simulink library "GTPR_Library"  (R2021a)
(part 7 of 8)

Mddq = [ddq1.*(ILAxx.*sin(alphaAA-pi./2.0).^2+ILAyy.*cos(alphaAA-pi./2.0).^2+ILAxy.*sin(alphaAA-pi./2.0).*cos(alphaAA-pi./2.0).*2.0)+((((dx-LA.*dq1.*sin(q1).*cos(alphaAA-pi./2.0)).*(y+aA.*cos(alphaAA)-eA.*cos(alphaAA)+LA.*cos(alphaAA).*cos(q1)))./lA-((dy+LA.*dq1.*sin(alphaAA-pi./2.0).*sin(q1)).*(x+aA.*sin(alphaAA)-eA.*sin(alphaAA)+LA.*cos(q1).*sin(alphaAA)))./lA).*((IlAxz.*((LA.*cos(q1).*(dy+LA.*dq1.*sin(alphaAA-pi./2.0).*sin(q1)))./lA+(LA.*cos(alphaAA).*sin(q1).*(dz+LA.*dq1.*sin(pi./2.0).*cos(q1)))./lA+(LA.*dq1.*sin(alphaAA-pi./2.0).*cos(q1).*(z+LA.*sin(q1)))./lA+(LA.*dq1.*sin(pi./2.0).*sin(q1).*(y+aA.*cos(alphaAA)-eA.*cos(alphaAA)+LA.*cos(alphaAA).*cos(q1)))./lA).*(-1.0./2.0))./lA+(IlAyz.*((LA.*cos(q1).*(dx-LA.*dq1.*sin(q1).*cos(alphaAA-pi./2.0)))./lA+(LA.*sin(alphaAA).*sin(q1).*(dz+LA.*dq1.*sin(pi./2.0).*cos(q1)))./lA-(LA.*dq1.*cos(q1).*cos(alphaAA-pi./2.0).*(z+LA.*sin(q1)))./lA+(LA.*dq1.*sin(pi./2.0).*sin(q1).*(x+aA.*sin(alphaAA)-eA.*sin(alphaAA)+LA.*cos(q1).*sin(alphaAA)))./lA))./(lA.*2.0)+(IlAzz.*((LA.*cos(alphaAA).*sin(q1).*(dx-LA.*dq1.*sin(q1).*cos(alphaAA-pi./2.0)))./lA-(LA.*sin(alphaAA).*sin(q1).*(dy+LA.*dq1.*sin(alphaAA-pi./2.0).*sin(q1)))./lA+(LA.*dq1.*sin(alphaAA-pi./2.0).*cos(q1).*(x+aA.*sin(alphaAA)-eA.*sin(alphaAA)+LA.*cos(q1).*sin(alphaAA)))./lA+(LA.*dq1.*cos(q1).*cos(alphaAA-pi./2.0).*(y+aA.*cos(alphaAA)-eA.*cos(alphaAA)+LA.*cos(alphaAA).*cos(q1)))./lA))./(lA.*2.0)).*2.0)./lA+((((dx-LA.*dq1.*sin(q1).*cos(alphaAA-pi./2.0)).*(y+aA.*cos(alphaAA)-eA.*cos(alphaAA)+LA.*cos(alphaAA).*cos(q1)))./lA-((dy+LA.*dq1.*sin(alphaAA-pi./2.0).*sin(q1)).*(x+aA.*sin(alphaAA)-eA.*sin(alphaAA)+LA.*cos(q1).*sin(alphaAA)))./lA).*((IlAxz.*((LA.*sin(alphaAA-pi./2.0).*sin(q1).*(dz+LA.*dq1.*cos(q1)))./lA-(LA.*sin(pi./2.0).*cos(q1).*(dy-LA.*dq1.*cos(alphaAA).*sin(q1)))./lA+(LA.*dq1.*sin(alphaAA-pi./2.0).*cos(q1).*(z+LA.*sin(q1)))./lA+(LA.*dq1.*sin(pi./2.0).*sin(q1).*(y+aA.*cos(alphaAA)-eA.*cos(alphaAA)+LA.*cos(alphaAA).*cos(q1)))./lA))./(lA.*2.0)+(IlAyz.*((LA.*sin(pi./2.0).*cos(q1).*(dx-LA.*dq1.*sin(alphaAA).*sin(q1)))./lA+(LA.*sin(q1).*cos(alphaAA-pi./2.0).*(dz+LA.*dq1.*cos(q1)))./lA+(LA.*dq1.*cos(q1).*cos(alphaAA-pi./2.0).*(z+LA.*sin(q1)))./lA-(LA.*dq1.*sin(pi./2.0).*sin(q1).*(x+aA.*sin(alphaAA)-eA.*sin(alphaAA)+LA.*cos(q1).*sin(alphaAA)))./lA))./(lA.*2.0)-(IlAzz.*((LA.*sin(q1).*cos(alphaAA-pi./2.0).*(dy-LA.*dq1.*cos(alphaAA).*sin(q1)))./lA+(LA.*sin(alphaAA-pi./2.0).*sin(q1).*(dx-LA.*dq1.*sin(alphaAA).*sin(q1)))./lA+(LA.*dq1.*sin(alphaAA-pi./2.0).*cos(q1).*(x+aA.*sin(alphaAA)-eA.*sin(alphaAA)+LA.*cos(q1).*sin(alphaAA)))./lA+(LA.*dq1.*cos(q1).*cos(alphaAA-pi./2.0).*(y+aA.*cos(alphaAA)-eA.*cos(alphaAA)+LA.*cos(alphaAA).*cos(q1)))./lA))./(lA.*2.0)).*2.0)./lA-(((LA.*sin(q1).*cos(alphaAA-pi./2.0).*(y+aA.*cos(alphaAA)-eA.*cos(alphaAA)+LA.*cos(alphaAA).*cos(q1)))./lA+(LA.*sin(alphaAA-pi./2.0).*sin(q1).*(x+aA.*sin(alphaAA)-eA.*sin(alphaAA)+LA.*cos(q1).*sin(alphaAA)))./lA).*((IlAxz.*(((dz+LA.*dq1.*cos(q1)).*(dy+LA.*dq1.*sin(alphaAA-pi./2.0).*sin(q1)))./lA-((dy-LA.*dq1.*cos(alphaAA).*sin(q1)).*(dz+LA.*dq1.*sin(pi./2.0).*cos(q1)))./lA+((z+LA.*sin(q1)).*(ddy+LA.*dq1.^2.*sin(alphaAA-pi./2.0).*cos(q1)+LA.*ddq1.*sin(alphaAA-pi./2.0).*sin(q1)))./lA-((ddz+LA.*ddq1.*sin(pi./2.0).*cos(q1)-LA.*dq1.^2.*sin(pi./2.0).*sin(q1)).*(y+aA.*cos(alphaAA)-eA.*cos(alphaAA)+LA.*cos(alphaAA).*cos(q1)))./lA))./(lA.*2.0)-(IlAzz.*(-((dy-LA.*dq1.*cos(alphaAA).*sin(q1)).*(dx-LA.*dq1.*sin(q1).*cos(alphaAA-pi./2.0)))./lA+((dx-LA.*dq1.*sin(alphaAA).*sin(q1)).*(dy+LA.*dq1.*sin(alphaAA-pi./2.0).*sin(q1)))./lA+((ddy+LA.*dq1.^2.*sin(alphaAA-pi./2.0).*cos(q1)+LA.*ddq1.*sin(alphaAA-pi./2.0).*sin(q1)).*(x+aA.*sin(alphaAA)-eA.*sin(alphaAA)+LA.*cos(q1).*sin(alphaAA)))./lA+((-ddx+LA.*dq1.^2.*cos(q1).*cos(alphaAA-pi./2.0)+LA.*ddq1.*sin(q1).*cos(alphaAA-pi./2.0)).*(y+aA.*cos(alphaAA)-eA.*cos(alphaAA)+LA.*cos(alphaAA).*cos(q1)))./lA))./(lA.*2.0)+(IlAyz.*(((ddz+LA.*ddq1.*sin(pi./2.0).*cos(q1)-LA.*dq1.^2.*sin(pi./2.0).*sin(q1)).*(x+aA.*sin(alphaAA)-eA.*sin(alphaAA)+LA.*cos(q1).*sin(alphaAA)))./lA-((dz+LA.*dq1.*cos(q1)).*(dx-LA.*dq1.*sin(q1).*cos(alphaAA-pi./2.0)))./lA+((dx-LA.*dq1.*sin(alphaAA).*sin(q1)).*(dz+LA.*dq1.*sin(pi./2.0).*cos(q1)))./lA+((z+LA.*sin(q1)).*(-ddx+LA.*dq1.^2.*cos(q1).*cos(alphaAA-pi./2.0)+LA.*ddq1.*sin(q1).*cos(alphaAA-pi./2.0)))./lA))./(lA.*2.0)).*2.0)./lA+(((IlAxz.*(((dx-LA.*dq1.*sin(q1).*cos(alphaAA-pi./2.0)).*(y+aA.*cos(alphaAA)-eA.*cos(alphaAA)+LA.*cos(alphaAA).*cos(q1)))./lA-((dy+LA.*dq1.*sin(alphaAA-pi./2.0).*sin(q1)).*(x+aA.*sin(alphaAA)-eA.*sin(alphaAA)+LA.*cos(q1).*sin(alphaAA)))./lA).*(-1.0./2.0))./lA+(IlAxx.*(((dz+LA.*dq1.*sin(pi./2.0).*cos(q1)).*(y+aA.*cos(alphaAA)-eA.*cos(alphaAA)+LA.*cos(alphaAA).*cos(q1)))./lA-((z+LA.*sin(q1)).*(dy+LA.*dq1.*sin(alphaAA-pi./2.0).*sin(q1)))./lA))./(lA.*2.0)+(IlAxy.*(((z+LA.*sin(q1)).*(dx-LA.*dq1.*sin(q1).*cos(alphaAA-pi./2.0)))./lA-((dz+LA.*dq1.*sin(pi./2.0).*cos(q1)).*(x+aA.*sin(alphaAA)-eA.*sin(alphaAA)+LA.*cos(q1).*sin(alphaAA)))./lA))./(lA.*2.0)).*((LA.*cos(q1).*(dy+LA.*dq1.*sin(alphaAA-pi./2.0).*sin(q1)))./lA+(LA.*cos(alphaAA).*sin(q1).*(dz+LA.*dq1.*sin(pi./2.0).*cos(q1)))./lA+(LA.*dq1.*sin(alphaAA-pi./2.0).*cos(q1).*(z+LA.*sin(q1)))./lA+(LA.*dq1.*sin(pi./2.0).*sin(q1).*(y+aA.*cos(alphaAA)-eA.*cos(alphaAA)+LA.*cos(alphaAA).*cos(q1)))./lA).*2.0)./lA-(((IlAxz.*(((dx-LA.*dq1.*sin(q1).*cos(alphaAA-pi./2.0)).*(y+aA.*cos(alphaAA)-eA.*cos(alphaAA)+LA.*cos(alphaAA).*cos(q1)))./lA-((dy+LA.*dq1.*sin(alphaAA-pi./2.0).*sin(q1)).*(x+aA.*sin(alphaAA)-eA.*sin(alphaAA)+LA.*cos(q1).*sin(alphaAA)))./lA).*(-1.0./2.0))./lA+(IlAxx.*(((dz+LA.*dq1.*sin(pi./2.0).*cos(q1)).*(y+aA.*cos(alphaAA)-eA.*cos(alphaAA)+LA.*cos(alphaAA).*cos(q1)))./lA-((z+LA.*sin(q1)).*(dy+LA.*dq1.*sin(alphaAA-pi./2.0).*sin(q1)))./lA))./(lA.*2.0)+(IlAxy.*(((z+LA.*sin(q1)).*(dx-LA.*dq1.*sin(q1).*cos(alphaAA-pi./2.0)))./lA-((dz+LA.*dq1.*sin(pi./2.0).*cos(q1)).*(x+aA.*sin(alphaAA)-eA.*sin(alphaAA)+LA.*cos(q1).*sin(alphaAA)))./lA))./(lA.*2.0)).*((LA.*sin(alphaAA-pi./2.0).*sin(q1).*(dz+LA.*dq1.*cos(q1)))./lA-(LA.*sin(pi./2.0).*cos(q1).*(dy-LA.*dq1.*cos(alphaAA).*sin(q1)))./lA+(LA.*dq1.*sin(alphaAA-pi./2.0).*cos(q1).*(z+LA.*sin(q1)))./lA+(LA.*dq1.*sin(pi./2.0).*sin(q1).*(y+aA.*cos(alphaAA)-eA.*cos(alphaAA)+LA.*cos(alphaAA).*cos(q1)))./lA).*2.0)./lA-(((IlAxz.*((LA.*sin(q1).*cos(alphaAA-pi./2.0).*(y+aA.*cos(alphaAA)-eA.*cos(alphaAA)+LA.*cos(alphaAA).*cos(q1)))./lA+(LA.*sin(alphaAA-pi./2.0).*sin(q1).*(x+aA.*sin(alphaAA)-eA.*sin(alphaAA)+LA.*cos(q1).*sin(alphaAA)))./lA))./(lA.*2.0)+(IlAxx.*((LA.*sin(pi./2.0).*cos(q1).*(y+aA.*cos(alphaAA)-eA.*cos(alphaAA)+LA.*cos(alphaAA).*cos(q1)))./lA-(LA.*sin(alphaAA-pi./2.0).*sin(q1).*(z+LA.*sin(q1)))./lA))./(lA.*2.0)-(IlAxy.*((LA.*sin(q1).*cos(alphaAA-pi./2.0).*(z+LA.*sin(q1)))./lA+(LA.*sin(pi./2.0).*cos(q1).*(x+aA.*sin(alphaAA)-eA.*sin(alphaAA)+LA.*cos(q1).*sin(alphaAA)))./lA))./(lA.*2.0)).*(((dz+LA.*dq1.*cos(q1)).*(dy+LA.*dq1.*sin(alphaAA-pi./2.0).*sin(q1)))./lA-((dy-LA.*dq1.*cos(alphaAA).*sin(q1)).*(dz+LA.*dq1.*sin(pi./2.0).*cos(q1)))./lA+((z+LA.*sin(q1)).*(ddy+LA.*dq1.^2.*sin(alphaAA-pi./2.0).*cos(q1)+LA.*ddq1.*sin(alphaAA-pi./2.0).*sin(q1)))./lA-((ddz+LA.*ddq1.*sin(pi./2.0).*cos(q1)-LA.*dq1.^2.*sin(pi./2.0).*sin(q1)).*(y+aA.*cos(alphaAA)-eA.*cos(alphaAA)+LA.*cos(alphaAA).*cos(q1)))./lA).*2.0)./lA-(((IlAyz.*(((dx-LA.*dq1.*sin(q1).*cos(alphaAA-pi./2.0)).*(y+aA.*cos(alphaAA)-eA.*cos(alphaAA)+LA.*cos(alphaAA).*cos(q1)))./lA-((dy+LA.*dq1.*sin(alphaAA-pi./2.0).*sin(q1)).*(x+aA.*sin(alphaAA)-eA.*sin(alphaAA)+LA.*cos(q1).*sin(alphaAA)))./lA).*(-1.0./2.0))./lA+(IlAxy.*(((dz+LA.*dq1.*sin(pi./2.0).*cos(q1)).*(y+aA.*cos(alphaAA)-eA.*cos(alphaAA)+LA.*cos(alphaAA).*cos(q1)))./lA-((z+LA.*sin(q1)).*(dy+LA.*dq1.*sin(alphaAA-pi./2.0).*sin(q1)))./lA))./(lA.*2.0)+(IlAyy.*(((z+LA.*sin(q1)).*(dx-LA.*dq1.*sin(q1).*cos(alphaAA-pi./2.0)))./lA-((dz+LA.*dq1.*sin(pi./2.0).*cos(q1)).*(x+aA.*sin(alphaAA)-eA.*sin(alphaAA)+LA.*cos(q1).*sin(alphaAA)))./lA))./(lA.*2.0)).*((LA.*cos(q1).*(dx-LA.*dq1.*sin(q1).*cos(alphaAA-pi./2.0)))./lA+(LA.*sin(alphaAA).*sin(q1).*(dz+LA.*dq1.*sin(pi./2.0).*cos(q1)))./lA-(LA.*dq1.*cos(q1).*cos(alphaAA-pi./2.0).*(z+LA.*sin(q1)))./lA+(LA.*dq1.*sin(pi./2.0).*sin(q1).*(x+aA.*sin(alphaAA)-eA.*sin(alphaAA)+LA.*cos(q1).*sin(alphaAA)))./lA).*2.0)./lA-(((IlAyz.*(((dx-LA.*dq1.*sin(q1).*cos(alphaAA-pi./2.0)).*(y+aA.*cos(alphaAA)-eA.*cos(alphaAA)+LA.*cos(alphaAA).*cos(q1)))./lA-((dy+LA.*dq1.*sin(alphaAA-pi./2.0).*sin(q1)).*(x+aA.*sin(alphaAA)-eA.*sin(alphaAA)+LA.*cos(q1).*sin(alphaAA)))./lA).*(-1.0./2.0))./lA+(IlAxy.*(((dz+LA.*dq1.*sin(pi./2.0).*cos(q1)).*(y+aA.*cos(alphaAA)-eA.*cos(alphaAA)+LA.*cos(alphaAA).*cos(q1)))./lA-((z+LA.*sin(q1)).*(dy+LA.*dq1.*sin(alphaAA-pi./2.0).*sin(q1)))./lA))./(lA.*2.0)+(IlAyy.*(((z+LA.*sin(q1)).*(dx-LA.*dq1.*sin(q1).*cos(alphaAA-pi./2.0)))./lA-((dz+LA.*dq1.*sin(pi./2.0).*cos(q1)).*(x+aA.*sin(alphaAA)-eA.*sin(alphaAA)+LA.*cos(q1).*sin(alphaAA)))./lA))./(lA.*2.0)).*((LA.*sin(pi./2.0).*cos(q1).*(dx-LA.*dq1.*sin(alphaAA).*sin(q1)))./lA+(LA.*sin(q1).*cos(alphaAA-pi./2.0).*(dz+LA.*dq1.*cos(q1)))./lA+(LA.*dq1.*cos(q1).*cos(alphaAA-pi./2.0).*(z+LA.*sin(q1)))./lA-(LA.*dq1.*sin(pi./2.0).*sin(q1).*(x+aA.*sin(alphaAA)-eA.*sin(alphaAA)+LA.*cos(q1).*sin(alphaAA)))./lA).*2.0)./lA-((((dz+LA.*dq1.*sin(pi./2.0).*cos(q1)).*(y+aA.*cos(alphaAA)-eA.*cos(alphaAA)+LA.*cos(alphaAA).*cos(q1)))./lA-((z+LA.*sin(q1)).*(dy+LA.*dq1.*sin(alphaAA-pi./2.0).*sin(q1)))./lA).*((IlAxx.*((LA.*cos(q1).*(dy+LA.*dq1.*sin(alphaAA-pi./2.0).*sin(q1)))./lA+(LA.*cos(alphaAA).*sin(q1).*(dz+LA.*dq1.*sin(pi./2.0).*cos(q1)))./lA+(LA.*dq1.*sin(alphaAA-pi./2.0).*cos(q1).*(z+LA.*sin(q1)))./lA+(LA.*dq1.*sin(pi./2.0).*sin(q1).*(y+aA.*cos(alphaAA)-eA.*cos(alphaAA)+LA.*cos(alphaAA).*cos(q1)))./lA).*(-1.0./2.0))./lA+(IlAxy.*((LA.*cos(q1).*(dx-LA.*dq1.*sin(q1).*cos(alphaAA-pi./2.0)))./lA+(LA.*sin(alphaAA).*sin(q1).*(dz+LA.*dq1.*sin(pi./2.0).*cos(q1)))./lA-(LA.*dq1.*cos(q1).*cos(alphaAA-pi./2.0).*(z+LA.*sin(q1)))./lA+(LA.*dq1.*sin(pi./2.0).*sin(q1).*(x+aA.*sin(alphaAA)-eA.*sin(alphaAA)+LA.*cos(q1).*sin(alphaAA)))./lA))./(lA.*2.0)+(IlAxz.*((LA.*cos(alphaAA).*sin(q1).*(dx-LA.*dq1.*sin(q1).*cos(alphaAA-pi./2.0)))./lA-(LA.*sin(alphaAA).*sin(q1).*(dy+LA.*dq1.*sin(alphaAA-pi./2.0).*sin(q1)))./lA+(LA.*dq1.*sin(alphaAA-pi./2.0).*cos(q1).*(x+aA.*sin(alphaAA)-eA.*sin(alphaAA)+LA.*cos(q1).*sin(alphaAA)))./lA+(LA.*dq1.*cos(q1).*cos(alphaAA-pi./2.0).*(y+aA.*cos(alphaAA)-eA.*cos(alphaAA)+LA.*cos(alphaAA).*cos(q1)))./lA))./(lA.*2.0)).*2.0)./lA-((((dz+LA.*dq1.*sin(pi./2.0).*cos(q1)).*(y+aA.*cos(alphaAA)-eA.*cos(alphaAA)+LA.*cos(alphaAA).*cos(q1)))./lA-((z+LA.*sin(q1)).*(dy+LA.*dq1.*sin(alphaAA-pi./2.0).*sin(q1)))./lA).*((IlAxx.*((LA.*sin(alphaAA-pi./2.0).*sin(q1).*(dz+LA.*dq1.*cos(q1)))./lA-(LA.*sin(pi./2.0).*cos(q1).*(dy-LA.*dq1.*cos(alphaAA).*sin(q1)))./lA+(LA.*dq1.*sin(alphaAA-pi./2.0).*cos(q1).*(z+LA.*sin(q1)))./lA+(LA.*dq1.*sin(pi./2.0).*sin(q1).*(y+aA.*cos(alphaAA)-eA.*cos(alphaAA)+LA.*cos(alphaAA).*cos(q1)))./lA))./(lA.*2.0)+(IlAxy.*((LA.*sin(pi./2.0).*cos(q1).*(dx-LA.*dq1.*sin(alphaAA).*sin(q1)))./lA+(LA.*sin(q1).*cos(alphaAA-pi./2.0).*(dz+LA.*dq1.*cos(q1)))./lA+(LA.*dq1.*cos(q1).*cos(alphaAA-pi./2.0).*(z+LA.*sin(q1)))./lA-(LA.*dq1.*sin(pi./2.0).*sin(q1).*(x+aA.*sin(alphaAA)-eA.*sin(alphaAA)+LA.*cos(q1).*sin(alphaAA)))./lA))./(lA.*2.0)-(IlAxz.*((LA.*sin(q1).*cos(alphaAA-pi./2.0).*(dy-LA.*dq1.*cos(alphaAA).*sin(q1)))./lA+(LA.*sin(alphaAA-pi./2.0).*sin(q1).*(dx-LA.*dq1.*sin(alphaAA).*sin(q1)))./lA+(LA.*dq1.*sin(alphaAA-pi./2.0).*cos(q1).*(x+aA.*sin(alphaAA)-eA.*sin(alphaAA)+LA.*cos(q1).*sin(alphaAA)))./lA+(LA.*dq1.*cos(q1).*cos(alphaAA-pi./2.0).*(y+aA.*cos(alphaAA)-eA.*cos(alphaAA)+LA.*cos(alphaAA).*cos(q1)))./lA))./(lA.*2.0)).*2.0)./lA-(((LA.*sin(pi./2.0).*cos(q1).*(y+aA.*cos(alphaAA)-eA.*cos(alphaAA)+LA.*cos(alphaAA).*cos(q1)))./lA-(LA.*sin(alphaAA-pi./2.0).*sin(q1).*(z+LA.*sin(q1)))./lA).*((IlAxx.*(((dz+LA.*dq1.*cos(q1)).*(dy+LA.*dq1.*sin(alphaAA-pi./2.0).*sin(q1)))./lA-((dy-LA.*dq1.*cos(alphaAA).*sin(q1)).*(dz+LA.*dq1.*sin(pi./2.0).*cos(q1)))./lA+((z+LA.*sin(q1)).*(ddy+LA.*dq1.^2.*sin(alphaAA-pi./2.0).*cos(q1)+LA.*ddq1.*sin(alphaAA-pi./2.0).*sin(q1)))./lA-((ddz+LA.*ddq1.*sin(pi./2.0).*cos(q1)-LA.*dq1.^2.*sin(pi./2.0).*sin(q1)).*(y+aA.*cos(alphaAA)-eA.*cos(alphaAA)+LA.*cos(alphaAA).*cos(q1)))./lA))./(lA.*2.0)-(IlAxz.*(-((dy-LA.*dq1.*cos(alphaAA).*sin(q1)).*(dx-LA.*dq1.*sin(q1).*cos(alphaAA-pi./2.0)))./lA+((dx-LA.*dq1.*sin(alphaAA).*sin(q1)).*(dy+LA.*dq1.*sin(alphaAA-pi./2.0).*sin(q1)))./lA+((ddy+LA.*dq1.^2.*sin(alphaAA-pi./2.0).*cos(q1)+LA.*ddq1.*sin(alphaAA-pi./2.0).*sin(q1)).*(x+aA.*sin(alphaAA)-eA.*sin(alphaAA)+LA.*cos(q1).*sin(alphaAA)))./lA+((-ddx+LA.*dq1.^2.*cos(q1).*cos(alphaAA-pi./2.0)+LA.*ddq1.*sin(q1).*cos(alphaAA-pi./2.0)).*(y+aA.*cos(alphaAA)-eA.*cos(alphaAA)+LA.*cos(alphaAA).*cos(q1)))./lA))./(lA.*2.0)+(IlAxy.*(((ddz+LA.*ddq1.*sin(pi./2.0).*cos(q1)-LA.*dq1.^2.*sin(pi./2.0).*sin(q1)).*(x+aA.*sin(alphaAA)-eA.*sin(alphaAA)+LA.*cos(q1).*sin(alphaAA)))./lA-((dz+LA.*dq1.*cos(q1)).*(dx-LA.*dq1.*sin(q1).*cos(alphaAA-pi./2.0)))./lA+((dx-LA.*dq1.*sin(alphaAA).*sin(q1)).*(dz+LA.*dq1.*sin(pi./2.0).*cos(q1)))./lA+((z+LA.*sin(q1)).*(-ddx+LA.*dq1.^2.*cos(q1).*cos(alphaAA-pi./2.0)+LA.*ddq1.*sin(q1).*cos(alphaAA-pi./2.0)))./lA))./(lA.*2.0)).*2.0)./lA-(((IlAzz.*(((dx-LA.*dq1.*sin(q1).*cos(alphaAA-pi./2.0)).*(y+aA.*cos(alphaAA)-eA.*cos(alphaAA)+LA.*cos(alphaAA).*cos(q1)))./lA-((dy+LA.*dq1.*sin(alphaAA-pi./2.0).*sin(q1)).*(x+aA.*sin(alphaAA)-eA.*sin(alphaAA)+LA.*cos(q1).*sin(alphaAA)))./lA).*(-1.0./2.0))./lA+(IlAxz.*(((dz+LA.*dq1.*sin(pi./2.0).*cos(q1)).*(y+aA.*cos(alphaAA)-eA.*cos(alphaAA)+LA.*cos(alphaAA).*cos(q1)))./lA-((z+LA.*sin(q1)).*(dy+LA.*dq1.*sin(alphaAA-pi./2.0).*sin(q1)))./lA))./(lA.*2.0)+(IlAyz.*(((z+LA.*sin(q1)).*(dx-LA.*dq1.*sin(q1).*cos(alphaAA-pi./2.0)))./lA-((dz+LA.*dq1.*sin(pi./2.0).*cos(q1)).*(x+aA.*sin(alphaAA)-eA.*sin(alphaAA)+LA.*cos(q1).*sin(alphaAA)))./lA))./(lA.*2.0)).*((LA.*cos(alphaAA).*sin(q1).*(dx-LA.*dq1.*sin(q1).*cos(alphaAA-pi./2.0)))./lA-(LA.*sin(alphaAA).*sin(q1).*(dy+LA.*dq1.*sin(alphaAA-pi./2.0).*sin(q1)))./lA+(LA.*dq1.*sin(alphaAA-pi./2.0).*cos(q1).*(x+aA.*sin(alphaAA)-eA.*sin(alphaAA)+LA.*cos(q1).*sin(alphaAA)))./lA+(LA.*dq1.*cos(q1).*cos(alphaAA-pi./2.0).*(y+aA.*cos(alphaAA)-eA.*cos(alphaAA)+LA.*cos(alphaAA).*cos(q1)))./lA).*2.0)./lA+(((IlAzz.*(((dx-LA.*dq1.*sin(q1).*cos(alphaAA-pi./2.0)).*(y+aA.*cos(alphaAA)-eA.*cos(alphaAA)+LA.*cos(alphaAA).*cos(q1)))./lA-((dy+LA.*dq1.*sin(alphaAA-pi./2.0).*sin(q1)).*(x+aA.*sin(alphaAA)-eA.*sin(alphaAA)+LA.*cos(q1).*sin(alphaAA)))./lA).*(-1.0./2.0))./lA+(IlAxz.*(((dz+LA.*dq1.*sin(pi./2.0).*cos(q1)).*(y+aA.*cos(alphaAA)-eA.*cos(alphaAA)+LA.*cos(alphaAA).*cos(q1)))./lA-((z+LA.*sin(q1)).*(dy+LA.*dq1.*sin(alphaAA-pi./2.0).*sin(q1)))./lA))./(lA.*2.0)+(IlAyz.*(((z+LA.*sin(q1)).*(dx-LA.*dq1.*sin(q1).*cos(alphaAA-pi./2.0)))./lA-((dz+LA.*dq1.*sin(pi./2.0).*cos(q1)).*(x+aA.*sin(alphaAA)-eA.*sin(alphaAA)+LA.*cos(q1).*sin(alphaAA)))./lA))./(lA.*2.0)).*((LA.*sin(q1).*cos(alphaAA-pi./2.0).*(dy-LA.*dq1.*cos(alphaAA).*sin(q1)))./lA+(LA.*sin(alphaAA-pi./2.0).*sin(q1).*(dx-LA.*dq1.*sin(alphaAA).*sin(q1)))./lA+(LA.*dq1.*sin(alphaAA-pi./2.0).*cos(q1).*(x+aA.*sin(alphaAA)-eA.*sin(alphaAA)+LA.*cos(q1).*sin(alphaAA)))./lA+(LA.*dq1.*cos(q1).*cos(alphaAA-pi./2.0).*(y+aA.*cos(alphaAA)-eA.*cos(alphaAA)+LA.*cos(alphaAA).*cos(q1)))./lA).*2.0)./lA-((((z+LA.*sin(q1)).*(dx-LA.*dq1.*sin(q1).*cos(alphaAA-pi./2.0)))./lA-((dz+LA.*dq1.*sin(pi./2.0).*cos(q1)).*(x+aA.*sin(alphaAA)-eA.*sin(alphaAA)+LA.*cos(q1).*sin(alphaAA)))./lA).*((IlAxy.*((LA.*cos(q1).*(dy+LA.*dq1.*sin(alphaAA-pi./2.0).*sin(q1)))./lA+(LA.*cos(alphaAA).*sin(q1).*(dz+LA.*dq1.*sin(pi./2.0).*cos(q1)))./lA+(LA.*dq1.*sin(alphaAA-pi./2.0).*cos(q1).*(z+LA.*sin(q1)))./lA+(LA.*dq1.*sin(pi./2.0).*sin(q1).*(y+aA.*cos(alphaAA)-eA.*cos(alphaAA)+LA.*cos(alphaAA).*cos(q1)))./lA).*(-1.0./2.0))./lA+(IlAyy.*((LA.*cos(q1).*(dx-LA.*dq1.*sin(q1).*cos(alphaAA-pi./2.0)))./lA+(LA.*sin(alphaAA).*sin(q1).*(dz+LA.*dq1.*sin(pi./2.0).*cos(q1)))./lA-(LA.*dq1.*cos(q1).*cos(alphaAA-pi./2.0).*(z+LA.*sin(q1)))./lA+(LA.*dq1.*sin(pi./2.0).*sin(q1).*(x+aA.*sin(alphaAA)-eA.*sin(alphaAA)+LA.*cos(q1).*sin(alphaAA)))./lA))./(lA.*2.0)+(IlAyz.*((LA.*cos(alphaAA).*sin(q1).*(dx-LA.*dq1.*sin(q1).*cos(alphaAA-pi./2.0)))./lA-(LA.*sin(alphaAA).*sin(q1).*(dy+LA.*dq1.*sin(alphaAA-pi./2.0).*sin(q1)))./lA+(LA.*dq1.*sin(alphaAA-pi./2.0).*cos(q1).*(x+aA.*sin(alphaAA)-eA.*sin(alphaAA)+LA.*cos(q1).*sin(alphaAA)))./lA+(LA.*dq1.*cos(q1).*cos(alphaAA-pi./2.0).*(y+aA.*cos(alphaAA)-eA.*cos(alphaAA)+LA.*cos(alphaAA).*cos(q1)))./lA))./(lA.*2.0)).*2.0)./lA-((((z+LA.*sin(q1)).*(dx-LA.*dq1.*sin(q1).*cos(alphaAA-pi./2.0)))./lA-((dz+LA.*dq1.*sin(pi./2.0).*cos(q1)).*(x+aA.*sin(alphaAA)-eA.*sin(alphaAA)+LA.*cos(q1).*sin(alphaAA)))./lA).*((IlAxy.*((LA.*sin(alphaAA-pi./2.0).*sin(q1).*(dz+LA.*dq1.*cos(q1)))./lA-(LA.*sin(pi./2.0).*cos(q1).*(dy-LA.*dq1.*cos(alphaAA).*sin(q1)))./lA+(LA.*dq1.*sin(alphaAA-pi./2.0).*cos(q1).*(z+LA.*sin(q1)))./lA+(LA.*dq1.*sin(pi./2.0).*sin(q1).*(y+aA.*cos(alphaAA)-eA.*cos(alphaAA)+LA.*cos(alphaAA).*cos(q1)))./lA))./(lA.*2.0)+(IlAyy.*((LA.*sin(pi./2.0).*cos(q1).*(dx-LA.*dq1.*sin(alphaAA).*sin(q1)))./lA+(LA.*sin(q1).*cos(alphaAA-pi./2.0).*(dz+LA.*dq1.*cos(q1)))./lA+(LA.*dq1.*cos(q1).*cos(alphaAA-pi./2.0).*(z+LA.*sin(q1)))./lA-(LA.*dq1.*sin(pi./2.0).*sin(q1).*(x+aA.*sin(alphaAA)-eA.*sin(alphaAA)+LA.*cos(q1).*sin(alphaAA)))./lA))./(lA.*2.0)-(IlAyz.*((LA.*sin(q1).*cos(alphaAA-pi./2.0).*(dy-LA.*dq1.*cos(alphaAA).*sin(q1)))./lA+(LA.*sin(alphaAA-pi./2.0).*sin(q1).*(dx-LA.*dq1.*sin(alphaAA).*sin(q1)))./lA+(LA.*dq1.*sin(alphaAA-pi./2.0).*cos(q1).*(x+aA.*sin(alphaAA)-eA.*sin(alphaAA)+LA.*cos(q1).*sin(alphaAA)))./lA+(LA.*dq1.*cos(q1).*cos(alphaAA-pi./2.0).*(y+aA.*cos(alphaAA)-eA.*cos(alphaAA)+LA.*cos(alphaAA).*cos(q1)))./lA))./(lA.*2.0)).*2.0)./lA+(((LA.*sin(q1).*cos(alphaAA-pi./2.0).*(z+LA.*sin(q1)))./lA+(LA.*sin(pi./2.0).*cos(q1).*(x+aA.*sin(alphaAA)-eA.*sin(alphaAA)+LA.*cos(q1).*sin(alphaAA)))./lA).*((IlAxy.*(((dz+LA.*dq1.*cos(q1)).*(dy+LA.*dq1.*sin(alphaAA-pi./2.0).*sin(q1)))./lA-((dy-LA.*dq1.*cos(alphaAA).*sin(q1)).*(dz+LA.*dq1.*sin(pi./2.0).*cos(q1)))./lA+((z+LA.*sin(q1)).*(ddy+LA.*dq1.^2.*sin(alphaAA-pi./2.0).*cos(q1)+LA.*ddq1.*sin(alphaAA-pi./2.0).*sin(q1)))./lA-((ddz+LA.*ddq1.*sin(pi./2.0).*cos(q1)-LA.*dq1.^2.*sin(pi./2.0).*sin(q1)).*(y+aA.*cos(alphaAA)-eA.*cos(alphaAA)+LA.*cos(alphaAA).*cos(q1)))./lA))./(lA.*2.0)-(IlAyz.*(-((dy-LA.*dq1.*cos(alphaAA).*sin(q1)).*(dx-LA.*dq1.*sin(q1).*cos(alphaAA-pi./2.0)))./lA+((dx-LA.*dq1.*sin(alphaAA).*sin(q1)).*(dy+LA.*dq1.*sin(alphaAA-pi./2.0).*sin(q1)))./lA+((ddy+LA.*dq1.^2.*sin(alphaAA-pi./2.0).*cos(q1)+LA.*ddq1.*sin(alphaAA-pi./2.0).*sin(q1)).*(x+aA.*sin(alphaAA)-eA.*sin(alphaAA)+LA.*cos(q1).*sin(alphaAA)))./lA+((-ddx+LA.*dq1.^2.*cos(q1).*cos(alphaAA-pi./2.0)+LA.*ddq1.*sin(q1).*cos(alphaAA-pi./2.0)).*(y+aA.*cos(alphaAA)-eA.*cos(alphaAA)+LA.*cos(alphaAA).*cos(q1)))./lA))./(lA.*2.0)+(IlAyy.*(((ddz+LA.*ddq1.*sin(pi./2.0).*cos(q1)-LA.*dq1.^2.*sin(pi./2.0).*sin(q1)).*(x+aA.*sin(alphaAA)-eA.*sin(alphaAA)+LA.*cos(q1).*sin(alphaAA)))./lA-((dz+LA.*dq1.*cos(q1)).*(dx-LA.*dq1.*sin(q1).*cos(alphaAA-pi./2.0)))./lA+((dx-LA.*dq1.*sin(alphaAA).*sin(q1)).*(dz+LA.*dq1.*sin(pi./2.0).*cos(q1)))./lA+((z+LA.*sin(q1)).*(-ddx+LA.*dq1.^2.*cos(q1).*cos(alphaAA-pi./2.0)+LA.*ddq1.*sin(q1).*cos(alphaAA-pi./2.0)))./lA))./(lA.*2.0)).*2.0)./lA+(((IlAzz.*((LA.*sin(q1).*cos(alphaAA-pi./2.0).*(y+aA.*cos(alphaAA)-eA.*cos(alphaAA)+LA.*cos(alphaAA).*cos(q1)))./lA+(LA.*sin(alphaAA-pi./2.0).*sin(q1).*(x+aA.*sin(alphaAA)-eA.*sin(alphaAA)+LA.*cos(q1).*sin(alphaAA)))./lA))./(lA.*2.0)+(IlAxz.*((LA.*sin(pi./2.0).*cos(q1).*(y+aA.*cos(alphaAA)-eA.*cos(alphaAA)+LA.*cos(alphaAA).*cos(q1)))./lA-(LA.*sin(alphaAA-pi./2.0).*sin(q1).*(z+LA.*sin(q1)))./lA))./(lA.*2.0)-(IlAyz.*((LA.*sin(q1).*cos(alphaAA-pi./2.0).*(z+LA.*sin(q1)))./lA+(LA.*sin(pi./2.0).*cos(q1).*(x+aA.*sin(alphaAA)-eA.*sin(alphaAA)+LA.*cos(q1).*sin(alphaAA)))./lA))./(lA.*2.0)).*(-((dy-LA.*dq1.*cos(alphaAA).*sin(q1)).*(dx-LA.*dq1.*sin(q1).*cos(alphaAA-pi./2.0)))./lA+((dx-LA.*dq1.*sin(alphaAA).*sin(q1)).*(dy+LA.*dq1.*sin(alphaAA-pi./2.0).*sin(q1)))./lA+((ddy+LA.*dq1.^2.*sin(alphaAA-pi./2.0).*cos(q1)+LA.*ddq1.*sin(alphaAA-pi./2.0).*sin(q1)).*(x+aA.*sin(alphaAA)-eA.*sin(alphaAA)+LA.*cos(q1).*sin(alphaAA)))./lA+((-ddx+LA.*dq1.^2.*cos(q1).*cos(alphaAA-pi./2.0)+LA.*ddq1.*sin(q1).*cos(alphaAA-pi./2.0)).*(y+aA.*cos(alphaAA)-eA.*cos(alphaAA)+LA.*cos(alphaAA).*cos(q1)))./lA).*2.0)./lA-(((IlAyz.*((LA.*sin(q1).*cos(alphaAA-pi./2.0).*(y+aA.*cos(alphaAA)-eA.*cos(alphaAA)+LA.*cos(alphaAA).*cos(q1)))./lA+(LA.*sin(alphaAA-pi./2.0).*sin(q1).*(x+aA.*sin(alphaAA)-eA.*sin(alphaAA)+LA.*cos(q1).*sin(alphaAA)))./lA))./(lA.*2.0)+(IlAxy.*((LA.*sin(pi./2.0).*cos(q1).*(y+aA.*cos(alphaAA)-eA.*cos(alphaAA)+LA.*cos(alphaAA).*cos(q1)))./lA-(LA.*sin(alphaAA-pi./2.0).*sin(q1).*(z+LA.*sin(q1)))./lA))./(lA.*2.0)-(IlAyy.*((LA.*sin(q1).*cos(alphaAA-pi./2.0).*(z+LA.*sin(q1)))./lA+(LA.*sin(pi./2.0).*cos(q1).*(x+aA.*sin(alphaAA)-eA.*sin(alphaAA)+LA.*cos(q1).*sin(alphaAA)))./lA))./(lA.*2.0)).*(((ddz+LA.*ddq1.*sin(pi./2.0).*cos(q1)-LA.*dq1.^2.*sin(pi./2.0).*sin(q1)).*(x+aA.*sin(alphaAA)-eA.*sin(alphaAA)+LA.*cos(q1).*sin(alphaAA)))./lA-((dz+LA.*dq1.*cos(q1)).*(dx-LA.*dq1.*sin(q1).*cos(alphaAA-pi./2.0)))./lA+((dx-LA.*dq1.*sin(alphaAA).*sin(q1)).*(dz+LA.*dq1.*sin(pi./2.0).*cos(q1)))./lA+((z+LA.*sin(q1)).*(-ddx+LA.*dq1.^2.*cos(q1).*cos(alphaAA-pi./2.0)+LA.*ddq1.*sin(q1).*cos(alphaAA-pi./2.0)))./lA).*2.0)./lA+(LA.*g.*mLA.*cos(q1))./2.0+LA.*g.*mlA.*cos(q1)-(LA.*mlA.*sin(pi./2.0).*cos(q1).*(ddz./2.0-(LA.*ddq1.*sin(pi./2.0).*cos(q1))./2.0+(LA.*dq1.^2.*sin(pi./2.0).*sin(q1))./2.0))./2.0-LA.*mlA.*sin(pi./2.0).*cos(q1).*(ddz./4.0-(LA.*ddq1.*sin(pi./2.0).*cos(q1))./4.0+(LA.*dq1.^2.*sin(pi./2.0).*sin(q1))./4.0)+(LA.*mlA.*sin(q1).*cos(alphaAA-pi./2.0).*(ddx./2.0+(LA.*dq1.^2.*cos(q1).*cos(alphaAA-pi./2.0))./2.0+(LA.*ddq1.*sin(q1).*cos(alphaAA-pi./2.0))./2.0))./2.0+LA.*mlA.*sin(q1).*cos(alphaAA-pi./2.0).*(ddx./4.0+(LA.*dq1.^2.*cos(q1).*cos(alphaAA-pi./2.0))./4.0+(LA.*ddq1.*sin(q1).*cos(alphaAA-pi./2.0))./4.0)+(LA.*mlA.*sin(alphaAA-pi./2.0).*sin(q1).*(ddy.*(-1.0./2.0)+(LA.*dq1.^2.*sin(alphaAA-pi./2.0).*cos(q1))./2.0+(LA.*ddq1.*sin(alphaAA-pi./2.0).*sin(q1))./2.0))./2.0+LA.*mlA.*sin(alphaAA-pi./2.0).*sin(q1).*(ddy.*(-1.0./4.0)+(LA.*dq1.^2.*sin(alphaAA-pi./2.0).*cos(q1))./4.0+(LA.*ddq1.*sin(alphaAA-pi./2.0).*sin(q1))./4.0);ddq2.*(ILBxx.*sin(alphaAB-pi./2.0).^2+ILByy.*cos(alphaAB-pi./2.0).^2+ILBxy.*sin(alphaAB-pi./2.0).*cos(alphaAB-pi./2.0).*2.0)+((((dx-LB.*dq2.*sin(q2).*cos(alphaAB-pi./2.0)).*(y+aB.*cos(alphaAB)-eB.*cos(alphaAB)+LB.*cos(alphaAB).*cos(q2)))./lB-((dy+LB.*dq2.*sin(alphaAB-pi./2.0).*sin(q2)).*(x+aB.*sin(alphaAB)-eB.*sin(alphaAB)+LB.*cos(q2).*sin(alphaAB)))./lB).*((IlBxz.*((LB.*cos(q2).*(dy+LB.*dq2.*sin(alphaAB-pi./2.0).*sin(q2)))./lB+(LB.*cos(alphaAB).*sin(q2).*(dz+LB.*dq2.*sin(pi./2.0).*cos(q2)))./lB+(LB.*dq2.*sin(alphaAB-pi./2.0).*cos(q2).*(z+LB.*sin(q2)))./lB+(LB.*dq2.*sin(pi./2.0).*sin(q2).*(y+aB.*cos(alphaAB)-eB.*cos(alphaAB)+LB.*cos(alphaAB).*cos(q2)))./lB).*(-1.0./2.0))./lB+(IlByz.*((LB.*cos(q2).*(dx-LB.*dq2.*sin(q2).*cos(alphaAB-pi./2.0)))./lB+(LB.*sin(alphaAB).*sin(q2).*(dz+LB.*dq2.*sin(pi./2.0).*cos(q2)))./lB-(LB.*dq2.*cos(q2).*cos(alphaAB-pi./2.0).*(z+LB.*sin(q2)))./lB+(LB.*dq2.*sin(pi./2.0).*sin(q2).*(x+aB.*sin(alphaAB)-eB.*sin(alphaAB)+LB.*cos(q2).*sin(alphaAB)))./lB))./(lB.*2.0)+(IlBzz.*((LB.*cos(alphaAB).*sin(q2).*(dx-LB.*dq2.*sin(q2).*cos(alphaAB-pi./2.0)))./lB-(LB.*sin(alphaAB).*sin(q2).*(dy+LB.*dq2.*sin(alphaAB-pi./2.0).*sin(q2)))./lB+(LB.*dq2.*sin(alphaAB-pi./2.0).*cos(q2).*(x+aB.*sin(alphaAB)-eB.*sin(alphaAB)+LB.*cos(q2).*sin(alphaAB)))./lB+(LB.*dq2.*cos(q2).*cos(alphaAB-pi./2.0).*(y+aB.*cos(alphaAB)-eB.*cos(alphaAB)+LB.*cos(alphaAB).*cos(q2)))./lB))./(lB.*2.0)).*2.0)./lB+((((dx-LB.*dq2.*sin(q2).*cos(alphaAB-pi./2.0)).*(y+aB.*cos(alphaAB)-eB.*cos(alphaAB)+LB.*cos(alphaAB).*cos(q2)))./lB-((dy+LB.*dq2.*sin(alphaAB-pi./2.0).*sin(q2)).*(x+aB.*sin(alphaAB)-eB.*sin(alphaAB)+LB.*cos(q2).*sin(alphaAB)))./lB).*((IlBxz.*((LB.*sin(alphaAB-pi./2.0).*sin(q2).*(dz+LB.*dq2.*cos(q2)))./lB-(LB.*sin(pi./2.0).*cos(q2).*(dy-LB.*dq2.*cos(alphaAB).*sin(q2)))./lB+(LB.*dq2.*sin(alphaAB-pi./2.0).*cos(q2).*(z+LB.*sin(q2)))./lB+(LB.*dq2.*sin(pi./2.0).*sin(q2).*(y+aB.*cos(alphaAB)-eB.*cos(alphaAB)+LB.*cos(alphaAB).*cos(q2)))./lB))./(lB.*2.0)+(IlByz.*((LB.*sin(pi./2.0).*cos(q2).*(dx-LB.*dq2.*sin(alphaAB).*sin(q2)))./lB+(LB.*sin(q2).*cos(alphaAB-pi./2.0).*(dz+LB.*dq2.*cos(q2)))./lB+(LB.*dq2.*cos(q2).*cos(alphaAB-pi./2.0).*(z+LB.*sin(q2)))./lB-(LB.*dq2.*sin(pi./2.0).*sin(q2).*(x+aB.*sin(alphaAB)-eB.*sin(alphaAB)+LB.*cos(q2).*sin(alphaAB)))./lB))./(lB.*2.0)-(IlBzz.*((LB.*sin(q2).*cos(alphaAB-pi./2.0).*(dy-LB.*dq2.*cos(alphaAB).*sin(q2)))./lB+(LB.*sin(alphaAB-pi./2.0).*sin(q2).*(dx-LB.*dq2.*sin(alphaAB).*sin(q2)))./lB+(LB.*dq2.*sin(alphaAB-pi./2.0).*cos(q2).*(x+aB.*sin(alphaAB)-eB.*sin(alphaAB)+LB.*cos(q2).*sin(alphaAB)))./lB+(LB.*dq2.*cos(q2).*cos(alphaAB-pi./2.0).*(y+aB.*cos(alphaAB)-eB.*cos(alphaAB)+LB.*cos(alphaAB).*cos(q2)))./lB))./(lB.*2.0)).*2.0)./lB-(((LB.*sin(q2).*cos(alphaAB-pi./2.0).*(y+aB.*cos(alphaAB)-eB.*cos(alphaAB)+LB.*cos(alphaAB).*cos(q2)))./lB+(LB.*sin(alphaAB-pi./2.0).*sin(q2).*(x+aB.*sin(alphaAB)-eB.*sin(alphaAB)+LB.*cos(q2).*sin(alphaAB)))./lB).*((IlBxz.*(((dz+LB.*dq2.*cos(q2)).*(dy+LB.*dq2.*sin(alphaAB-pi./2.0).*sin(q2)))./lB-((dy-LB.*dq2.*cos(alphaAB).*sin(q2)).*(dz+LB.*dq2.*sin(pi./2.0).*cos(q2)))./lB+((z+LB.*sin(q2)).*(ddy+LB.*dq2.^2.*sin(alphaAB-pi./2.0).*cos(q2)+LB.*ddq2.*sin(alphaAB-pi./2.0).*sin(q2)))./lB-((ddz+LB.*ddq2.*sin(pi./2.0).*cos(q2)-LB.*dq2.^2.*sin(pi./2.0).*sin(q2)).*(y+aB.*cos(alphaAB)-eB.*cos(alphaAB)+LB.*cos(alphaAB).*cos(q2)))./lB))./(lB.*2.0)-(IlBzz.*(-((dy-LB.*dq2.*cos(alphaAB).*sin(q2)).*(dx-LB.*dq2.*sin(q2).*cos(alphaAB-pi./2.0)))./lB+((dx-LB.*dq2.*sin(alphaAB).*sin(q2)).*(dy+LB.*dq2.*sin(alphaAB-pi./2.0).*sin(q2)))./lB+((ddy+LB.*dq2.^2.*sin(alphaAB-pi./2.0).*cos(q2)+LB.*ddq2.*sin(alphaAB-pi./2.0).*sin(q2)).*(x+aB.*sin(alphaAB)-eB.*sin(alphaAB)+LB.*cos(q2).*sin(alphaAB)))./lB+((-ddx+LB.*dq2.^2.*cos(q2).*cos(alphaAB-pi./2.0)+LB.*ddq2.*sin(q2).*cos(alphaAB-pi./2.0)).*(y+aB.*cos(alphaAB)-eB.*cos(alphaAB)+LB.*cos(alphaAB).*cos(q2)))./lB))./(lB.*2.0)+(IlByz.*(((ddz+LB.*ddq2.*sin(pi./2.0).*cos(q2)-LB.*dq2.^2.*sin(pi./2.0).*sin(q2)).*(x+aB.*sin(alphaAB)-eB.*sin(alphaAB)+LB.*cos(q2).*sin(alphaAB)))./lB-((dz+LB.*dq2.*cos(q2)).*(dx-LB.*dq2.*sin(q2).*cos(alphaAB-pi./2.0)))./lB+((dx-LB.*dq2.*sin(alphaAB).*sin(q2)).*(dz+LB.*dq2.*sin(pi./2.0).*cos(q2)))./lB+((z+LB.*sin(q2)).*(-ddx+LB.*dq2.^2.*cos(q2).*cos(alphaAB-pi./2.0)+LB.*ddq2.*sin(q2).*cos(alphaAB-pi./2.0)))./lB))./(lB.*2.0)).*2.0)./lB+(((IlBxz.*(((dx-LB.*dq2.*sin(q2).*cos(alphaAB-pi./2.0)).*(y+aB.*cos(alphaAB)-eB.*cos(alphaAB)+LB.*cos(alphaAB).*cos(q2)))./lB-((dy+LB.*dq2.*sin(alphaAB-pi./2.0).*sin(q2)).*(x+aB.*sin(alphaAB)-eB.*sin(alphaAB)+LB.*cos(q2).*sin(alphaAB)))./lB).*(-1.0./2.0))./lB+(IlBxx.*(((dz+LB.*dq2.*sin(pi./2.0).*cos(q2)).*(y+aB.*cos(alphaAB)-eB.*cos(alphaAB)+LB.*cos(alphaAB).*cos(q2)))./lB-((z+LB.*sin(q2)).*(dy+LB.*dq2.*sin(alphaAB-pi./2.0).*sin(q2)))./lB))./(lB.*2.0)+(IlBxy.*(((z+LB.*sin(q2)).*(dx-LB.*dq2.*sin(q2).*cos(alphaAB-pi./2.0)))./lB-((dz+LB.*dq2.*sin(pi./2.0).*cos(q2)).*(x+aB.*sin(alphaAB)-eB.*sin(alphaAB)+LB.*cos(q2).*sin(alphaAB)))./lB))./(lB.*2.0)).*((LB.*cos(q2).*(dy+LB.*dq2.*sin(alphaAB-pi./2.0).*sin(q2)))./lB+(LB.*cos(alphaAB).*sin(q2).*(dz+LB.*dq2.*sin(pi./2.0).*cos(q2)))./lB+(LB.*dq2.*sin(alphaAB-pi./2.0).*cos(q2).*(z+LB.*sin(q2)))./lB+(LB.*dq2.*sin(pi./2.0).*sin(q2).*(y+aB.*cos(alphaAB)-eB.*cos(alphaAB)+LB.*cos(alphaAB).*cos(q2)))./lB).*2.0)./lB-(((IlBxz.*(((dx-LB.*dq2.*sin(q2).*cos(alphaAB-pi./2.0)).*(y+aB.*cos(alphaAB)-eB.*cos(alphaAB)+LB.*cos(alphaAB).*cos(q2)))./lB-((dy+LB.*dq2.*sin(alphaAB-pi./2.0).*sin(q2)).*(x+aB.*sin(alphaAB)-eB.*sin(alphaAB)+LB.*cos(q2).*sin(alphaAB)))./lB).*(-1.0./2.0))./lB+(IlBxx.*(((dz+LB.*dq2.*sin(pi./2.0).*cos(q2)).*(y+aB.*cos(alphaAB)-eB.*cos(alphaAB)+LB.*cos(alphaAB).*cos(q2)))./lB-((z+LB.*sin(q2)).*(dy+LB.*dq2.*sin(alphaAB-pi./2.0).*sin(q2)))./lB))./(lB.*2.0)+(IlBxy.*(((z+LB.*sin(q2)).*(dx-LB.*dq2.*sin(q2).*cos(alphaAB-pi./2.0)))./lB-((dz+LB.*dq2.*sin(pi./2.0).*cos(q2)).*(x+aB.*sin(alphaAB)-eB.*sin(alphaAB)+LB.*cos(q2).*sin(alphaAB)))./lB))./(lB.*2.0)).*((LB.*sin(alphaAB-pi./2.0).*sin(q2).*(dz+LB.*dq2.*cos(q2)))./lB-(LB.*sin(pi./2.0).*cos(q2).*(dy-LB.*dq2.*cos(alphaAB).*sin(q2)))./lB+(LB.*dq2.*sin(alphaAB-pi./2.0).*cos(q2).*(z+LB.*sin(q2)))./lB+(LB.*dq2.*sin(pi./2.0).*sin(q2).*(y+aB.*cos(alphaAB)-eB.*cos(alphaAB)+LB.*cos(alphaAB).*cos(q2)))./lB).*2.0)./lB-(((IlBxz.*((LB.*sin(q2).*cos(alphaAB-pi./2.0).*(y+aB.*cos(alphaAB)-eB.*cos(alphaAB)+LB.*cos(alphaAB).*cos(q2)))./lB+(LB.*sin(alphaAB-pi./2.0).*sin(q2).*(x+aB.*sin(alphaAB)-eB.*sin(alphaAB)+LB.*cos(q2).*sin(alphaAB)))./lB))./(lB.*2.0)+(IlBxx.*((LB.*sin(pi./2.0).*cos(q2).*(y+aB.*cos(alphaAB)-eB.*cos(alphaAB)+LB.*cos(alphaAB).*cos(q2)))./lB-(LB.*sin(alphaAB-pi./2.0).*sin(q2).*(z+LB.*sin(q2)))./lB))./(lB.*2.0)-(IlBxy.*((LB.*sin(q2).*cos(alphaAB-pi./2.0).*(z+LB.*sin(q2)))./lB+(LB.*sin(pi./2.0).*cos(q2).*(x+aB.*sin(alphaAB)-eB.*sin(alphaAB)+LB.*cos(q2).*sin(alphaAB)))./lB))./(lB.*2.0)).*(((dz+LB.*dq2.*cos(q2)).*(dy+LB.*dq2.*sin(alphaAB-pi./2.0).*sin(q2)))./lB-((dy-LB.*dq2.*cos(alphaAB).*sin(q2)).*(dz+LB.*dq2.*sin(pi./2.0).*cos(q2)))./lB+((z+LB.*sin(q2)).*(ddy+LB.*dq2.^2.*sin(alphaAB-pi./2.0).*cos(q2)+LB.*ddq2.*sin(alphaAB-pi./2.0).*sin(q2)))./lB-((ddz+LB.*ddq2.*sin(pi./2.0).*cos(q2)-LB.*dq2.^2.*sin(pi./2.0).*sin(q2)).*(y+aB.*cos(alphaAB)-eB.*cos(alphaAB)+LB.*cos(alphaAB).*cos(q2)))./lB).*2.0)./lB-(((IlByz.*(((dx-LB.*dq2.*sin(q2).*cos(alphaAB-pi./2.0)).*(y+aB.*cos(alphaAB)-eB.*cos(alphaAB)+LB.*cos(alphaAB).*cos(q2)))./lB-((dy+LB.*dq2.*sin(alphaAB-pi./2.0).*sin(q2)).*(x+aB.*sin(alphaAB)-eB.*sin(alphaAB)+LB.*cos(q2).*sin(alphaAB)))./lB).*(-1.0./2.0))./lB+(IlBxy.*(((dz+LB.*dq2.*sin(pi./2.0).*cos(q2)).*(y+aB.*cos(alphaAB)-eB.*cos(alphaAB)+LB.*cos(alphaAB).*cos(q2)))./lB-((z+LB.*sin(q2)).*(dy+LB.*dq2.*sin(alphaAB-pi./2.0).*sin(q2)))./lB))./(lB.*2.0)+(IlByy.*(((z+LB.*sin(q2)).*(dx-LB.*dq2.*sin(q2).*cos(alphaAB-pi./2.0)))./lB-((dz+LB.*dq2.*sin(pi./2.0).*cos(q2)).*(x+aB.*sin(alphaAB)-eB.*sin(alphaAB)+LB.*cos(q2).*sin(alphaAB)))./lB))./(lB.*2.0)).*((LB.*cos(q2).*(dx-LB.*dq2.*sin(q2).*cos(alphaAB-pi./2.0)))./lB+(LB.*sin(alphaAB).*sin(q2).*(dz+LB.*dq2.*sin(pi./2.0).*cos(q2)))./lB-(LB.*dq2.*cos(q2).*cos(alphaAB-pi./2.0).*(z+LB.*sin(q2)))./lB+(LB.*dq2.*sin(pi./2.0).*sin(q2).*(x+aB.*sin(alphaAB)-eB.*sin(alphaAB)+LB.*cos(q2).*sin(alphaAB)))./lB).*2.0)./lB-(((IlByz.*(((dx-LB.*dq2.*sin(q2).*cos(alphaAB-pi./2.0)).*(y+aB.*cos(alphaAB)-eB.*cos(alphaAB)+LB.*cos(alphaAB).*cos(q2)))./lB-((dy+LB.*dq2.*sin(alphaAB-pi./2.0).*sin(q2)).*(x+aB.*sin(alphaAB)-eB.*sin(alphaAB)+LB.*cos(q2).*sin(alphaAB)))./lB).*(-1.0./2.0))./lB+(IlBxy.*(((dz+LB.*dq2.*sin(pi./2.0).*cos(q2)).*(y+aB.*cos(alphaAB)-eB.*cos(alphaAB)+LB.*cos(alphaAB).*cos(q2)))./lB-((z+LB.*sin(q2)).*(dy+LB.*dq2.*sin(alphaAB-pi./2.0).*sin(q2)))./lB))./(lB.*2.0)+(IlByy.*(((z+LB.*sin(q2)).*(dx-LB.*dq2.*sin(q2).*cos(alphaAB-pi./2.0)))./lB-((dz+LB.*dq2.*sin(pi./2.0).*cos(q2)).*(x+aB.*sin(alphaAB)-eB.*sin(alphaAB)+LB.*cos(q2).*sin(alphaAB)))./lB))./(lB.*2.0)).*((LB.*sin(pi./2.0).*cos(q2).*(dx-LB.*dq2.*sin(alphaAB).*sin(q2)))./lB+(LB.*sin(q2).*cos(alphaAB-pi./2.0).*(dz+LB.*dq2.*cos(q2)))./lB+(LB.*dq2.*cos(q2).*cos(alphaAB-pi./2.0).*(z+LB.*sin(q2)))./lB-(LB.*dq2.*sin(pi./2.0).*sin(q2).*(x+aB.*sin(alphaAB)-eB.*sin(alphaAB)+LB.*cos(q2).*sin(alphaAB)))./lB).*2.0)./lB-((((dz+LB.*dq2.*sin(pi./2.0).*cos(q2)).*(y+aB.*cos(alphaAB)-eB.*cos(alphaAB)+LB.*cos(alphaAB).*cos(q2)))./lB-((z+LB.*sin(q2)).*(dy+LB.*dq2.*sin(alphaAB-pi./2.0).*sin(q2)))./lB).*((IlBxx.*((LB.*cos(q2).*(dy+LB.*dq2.*sin(alphaAB-pi./2.0).*sin(q2)))./lB+(LB.*cos(alphaAB).*sin(q2).*(dz+LB.*dq2.*sin(pi./2.0).*cos(q2)))./lB+(LB.*dq2.*sin(alphaAB-pi./2.0).*cos(q2).*(z+LB.*sin(q2)))./lB+(LB.*dq2.*sin(pi./2.0).*sin(q2).*(y+aB.*cos(alphaAB)-eB.*cos(alphaAB)+LB.*cos(alphaAB).*cos(q2)))./lB).*(-1.0./2.0))./lB+(IlBxy.*((LB.*cos(q2).*(dx-LB.*dq2.*sin(q2).*cos(alphaAB-pi./2.0)))./lB+(LB.*sin(alphaAB).*sin(q2).*(dz+LB.*dq2.*sin(pi./2.0).*cos(q2)))./lB-(LB.*dq2.*cos(q2).*cos(alphaAB-pi./2.0).*(z+LB.*sin(q2)))./lB+(LB.*dq2.*sin(pi./2.0).*sin(q2).*(x+aB.*sin(alphaAB)-eB.*sin(alphaAB)+LB.*cos(q2).*sin(alphaAB)))./lB))./(lB.*2.0)+(IlBxz.*((LB.*cos(alphaAB).*sin(q2).*(dx-LB.*dq2.*sin(q2).*cos(alphaAB-pi./2.0)))./lB-(LB.*sin(alphaAB).*sin(q2).*(dy+LB.*dq2.*sin(alphaAB-pi./2.0).*sin(q2)))./lB+(LB.*dq2.*sin(alphaAB-pi./2.0).*cos(q2).*(x+aB.*sin(alphaAB)-eB.*sin(alphaAB)+LB.*cos(q2).*sin(alphaAB)))./lB+(LB.*dq2.*cos(q2).*cos(alphaAB-pi./2.0).*(y+aB.*cos(alphaAB)-eB.*cos(alphaAB)+LB.*cos(alphaAB).*cos(q2)))./lB))./(lB.*2.0)).*2.0)./lB-((((dz+LB.*dq2.*sin(pi./2.0).*cos(q2)).*(y+aB.*cos(alphaAB)-eB.*cos(alphaAB)+LB.*cos(alphaAB).*cos(q2)))./lB-((z+LB.*sin(q2)).*(dy+LB.*dq2.*sin(alphaAB-pi./2.0).*sin(q2)))./lB).*((IlBxx.*((LB.*sin(alphaAB-pi./2.0).*sin(q2).*(dz+LB.*dq2.*cos(q2)))./lB-(LB.*sin(pi./2.0).*cos(q2).*(dy-LB.*dq2.*cos(alphaAB).*sin(q2)))./lB+(LB.*dq2.*sin(alphaAB-pi./2.0).*cos(q2).*(z+LB.*sin(q2)))./lB+(LB.*dq2.*sin(pi./2.0).*sin(q2).*(y+aB.*cos(alphaAB)-eB.*cos(alphaAB)+LB.*cos(alphaAB).*cos(q2)))./lB))./(lB.*2.0)+(IlBxy.*((LB.*sin(pi./2.0).*cos(q2).*(dx-LB.*dq2.*sin(alphaAB).*sin(q2)))./lB+(LB.*sin(q2).*cos(alphaAB-pi./2.0).*(dz+LB.*dq2.*cos(q2)))./lB+(LB.*dq2.*cos(q2).*cos(alphaAB-pi./2.0).*(z+LB.*sin(q2)))./lB-(LB.*dq2.*sin(pi./2.0).*sin(q2).*(x+aB.*sin(alphaAB)-eB.*sin(alphaAB)+LB.*cos(q2).*sin(alphaAB)))./lB))./(lB.*2.0)-(IlBxz.*((LB.*sin(q2).*cos(alphaAB-pi./2.0).*(dy-LB.*dq2.*cos(alphaAB).*sin(q2)))./lB+(LB.*sin(alphaAB-pi./2.0).*sin(q2).*(dx-LB.*dq2.*sin(alphaAB).*sin(q2)))./lB+(LB.*dq2.*sin(alphaAB-pi./2.0).*cos(q2).*(x+aB.*sin(alphaAB)-eB.*sin(alphaAB)+LB.*cos(q2).*sin(alphaAB)))./lB+(LB.*dq2.*cos(q2).*cos(alphaAB-pi./2.0).*(y+aB.*cos(alphaAB)-eB.*cos(alphaAB)+LB.*cos(alphaAB).*cos(q2)))./lB))./(lB.*2.0)).*2.0)./lB-(((LB.*sin(pi./2.0).*cos(q2).*(y+aB.*cos(alphaAB)-eB.*cos(alphaAB)+LB.*cos(alphaAB).*cos(q2)))./lB-(LB.*sin(alphaAB-pi./2.0).*sin(q2).*(z+LB.*sin(q2)))./lB).*((IlBxx.*(((dz+LB.*dq2.*cos(q2)).*(dy+LB.*dq2.*sin(alphaAB-pi./2.0).*sin(q2)))./lB-((dy-LB.*dq2.*cos(alphaAB).*sin(q2)).*(dz+LB.*dq2.*sin(pi./2.0).*cos(q2)))./lB+((z+LB.*sin(q2)).*(ddy+LB.*dq2.^2.*sin(alphaAB-pi./2.0).*cos(q2)+LB.*ddq2.*sin(alphaAB-pi./2.0).*sin(q2)))./lB-((ddz+LB.*ddq2.*sin(pi./2.0).*cos(q2)-LB.*dq2.^2.*sin(pi./2.0).*sin(q2)).*(y+aB.*cos(alphaAB)-eB.*cos(alphaAB)+LB.*cos(alphaAB).*cos(q2)))./lB))./(lB.*2.0)-(IlBxz.*(-((dy-LB.*dq2.*cos(alphaAB).*sin(q2)).*(dx-LB.*dq2.*sin(q2).*cos(alphaAB-pi./2.0)))./lB+((dx-LB.*dq2.*sin(alphaAB).*sin(q2)).*(dy+LB.*dq2.*sin(alphaAB-pi./2.0).*sin(q2)))./lB+((ddy+LB.*dq2.^2.*sin(alphaAB-pi./2.0).*cos(q2)+LB.*ddq2.*sin(alphaAB-pi./2.0).*sin(q2)).*(x+aB.*sin(alphaAB)-eB.*sin(alphaAB)+LB.*cos(q2).*sin(alphaAB)))./lB+((-ddx+LB.*dq2.^2.*cos(q2).*cos(alphaAB-pi./2.0)+LB.*ddq2.*sin(q2).*cos(alphaAB-pi./2.0)).*(y+aB.*cos(alphaAB)-eB.*cos(alphaAB)+LB.*cos(alphaAB).*cos(q2)))./lB))./(lB.*2.0)+(IlBxy.*(((ddz+LB.*ddq2.*sin(pi./2.0).*cos(q2)-LB.*dq2.^2.*sin(pi./2.0).*sin(q2)).*(x+aB.*sin(alphaAB)-eB.*sin(alphaAB)+LB.*cos(q2).*sin(alphaAB)))./lB-((dz+LB.*dq2.*cos(q2)).*(dx-LB.*dq2.*sin(q2).*cos(alphaAB-pi./2.0)))./lB+((dx-LB.*dq2.*sin(alphaAB).*sin(q2)).*(dz+LB.*dq2.*sin(pi./2.0).*cos(q2)))./lB+((z+LB.*sin(q2)).*(-ddx+LB.*dq2.^2.*cos(q2).*cos(alphaAB-pi./2.0)+LB.*ddq2.*sin(q2).*cos(alphaAB-pi./2.0)))./lB))./(lB.*2.0)).*2.0)./lB-(((IlBzz.*(((dx-LB.*dq2.*sin(q2).*cos(alphaAB-pi./2.0)).*(y+aB.*cos(alphaAB)-eB.*cos(alphaAB)+LB.*cos(alphaAB).*cos(q2)))./lB-((dy+LB.*dq2.*sin(alphaAB-pi./2.0).*sin(q2)).*(x+aB.*sin(alphaAB)-eB.*sin(alphaAB)+LB.*cos(q2).*sin(alphaAB)))./lB).*(-1.0./2.0))./lB+(IlBxz.*(((dz+LB.*dq2.*sin(pi./2.0).*cos(q2)).*(y+aB.*cos(alphaAB)-eB.*cos(alphaAB)+LB.*cos(alphaAB).*cos(q2)))./lB-((z+LB.*sin(q2)).*(dy+LB.*dq2.*sin(alphaAB-pi./2.0).*sin(q2)))./lB))./(lB.*2.0)+(IlByz.*(((z+LB.*sin(q2)).*(dx-LB.*dq2.*sin(q2).*cos(alphaAB-pi./2.0)))./lB-((dz+LB.*dq2.*sin(pi./2.0).*cos(q2)).*(x+aB.*sin(alphaAB)-eB.*sin(alphaAB)+LB.*cos(q2).*sin(alphaAB)))./lB))./(lB.*2.0)).*((LB.*cos(alphaAB).*sin(q2).*(dx-LB.*dq2.*sin(q2).*cos(alphaAB-pi./2.0)))./lB-(LB.*sin(alphaAB).*sin(q2).*(dy+LB.*dq2.*sin(alphaAB-pi./2.0).*sin(q2)))./lB+(LB.*dq2.*sin(alphaAB-pi./2.0).*cos(q2).*(x+aB.*sin(alphaAB)-eB.*sin(alphaAB)+LB.*cos(q2).*sin(alphaAB)))./lB+(LB.*dq2.*cos(q2).*cos(alphaAB-pi./2.0).*(y+aB.*cos(alphaAB)-eB.*cos(alphaAB)+LB.*cos(alphaAB).*cos(q2)))./lB).*2.0)./lB+(((IlBzz.*(((dx-LB.*dq2.*sin(q2).*cos(alphaAB-pi./2.0)).*(y+aB.*cos(alphaAB)-eB.*cos(alphaAB)+LB.*cos(alphaAB).*cos(q2)))./lB-((dy+LB.*dq2.*sin(alphaAB-pi./2.0).*sin(q2)).*(x+aB.*sin(alphaAB)-eB.*sin(alphaAB)+LB.*cos(q2).*sin(alphaAB)))./lB).*(-1.0./2.0))./lB+(IlBxz.*(((dz+LB.*dq2.*sin(pi./2.0).*cos(q2)).*(y+aB.*cos(alphaAB)-eB.*cos(alphaAB)+LB.*cos(alphaAB).*cos(q2)))./lB-((z+LB.*sin(q2)).*(dy+LB.*dq2.*sin(alphaAB-pi./2.0).*sin(q2)))./lB))./(lB.*2.0)+(IlByz.*(((z+LB.*sin(q2)).*(dx-LB.*dq2.*sin(q2).*cos(alphaAB-pi./2.0)))./lB-((dz+LB.*dq2.*sin(pi./2.0).*cos(q2)).*(x+aB.*sin(alphaAB)-eB.*sin(alphaAB)+LB.*cos(q2).*sin(alphaAB)))./lB))./(lB.*2.0)).*((LB.*sin(q2).*cos(alphaAB-pi./2.0).*(dy-LB.*dq2.*cos(alphaAB).*sin(q2)))./lB+(LB.*sin(alphaAB-pi./2.0).*sin(q2).*(dx-LB.*dq2.*sin(alphaAB).*sin(q2)))./lB+(LB.*dq2.*sin(alphaAB-pi./2.0).*cos(q2).*(x+aB.*sin(alphaAB)-eB.*sin(alphaAB)+LB.*cos(q2).*sin(alphaAB)))./lB+(LB.*dq2.*cos(q2).*cos(alphaAB-pi./2.0).*(y+aB.*cos(alphaAB)-eB.*cos(alphaAB)+LB.*cos(alphaAB).*cos(q2)))./lB).*2.0)./lB-((((z+LB.*sin(q2)).*(dx-LB.*dq2.*sin(q2).*cos(alphaAB-pi./2.0)))./lB-((dz+LB.*dq2.*sin(pi./2.0).*cos(q2)).*(x+aB.*sin(alphaAB)-eB.*sin(alphaAB)+LB.*cos(q2).*sin(alphaAB)))./lB).*((IlBxy.*((LB.*cos(q2).*(dy+LB.*dq2.*sin(alphaAB-pi./2.0).*sin(q2)))./lB+(LB.*cos(alphaAB).*sin(q2).*(dz+LB.*dq2.*sin(pi./2.0).*cos(q2)))./lB+(LB.*dq2.*sin(alphaAB-pi./2.0).*cos(q2).*(z+LB.*sin(q2)))./lB+(LB.*dq2.*sin(pi./2.0).*sin(q2).*(y+aB.*cos(alphaAB)-eB.*cos(alphaAB)+LB.*cos(alphaAB).*cos(q2)))./lB).*(-1.0./2.0))./lB+(IlByy.*((LB.*cos(q2).*(dx-LB.*dq2.*sin(q2).*cos(alphaAB-pi./2.0)))./lB+(LB.*sin(alphaAB).*sin(q2).*(dz+LB.*dq2.*sin(pi./2.0).*cos(q2)))./lB-(LB.*dq2.*cos(q2).*cos(alphaAB-pi./2.0).*(z+LB.*sin(q2)))./lB+(LB.*dq2.*sin(pi./2.0).*sin(q2).*(x+aB.*sin(alphaAB)-eB.*sin(alphaAB)+LB.*cos(q2).*sin(alphaAB)))./lB))./(lB.*2.0)+(IlByz.*((LB.*cos(alphaAB).*sin(q2).*(dx-LB.*dq2.*sin(q2).*cos(alphaAB-pi./2.0)))./lB-(LB.*sin(alphaAB).*sin(q2).*(dy+LB.*dq2.*sin(alphaAB-pi./2.0).*sin(q2)))./lB+(LB.*dq2.*sin(alphaAB-pi./2.0).*cos(q2).*(x+aB.*sin(alphaAB)-eB.*sin(alphaAB)+LB.*cos(q2).*sin(alphaAB)))./lB+(LB.*dq2.*cos(q2).*cos(alphaAB-pi./2.0).*(y+aB.*cos(alphaAB)-eB.*cos(alphaAB)+LB.*cos(alphaAB).*cos(q2)))./lB))./(lB.*2.0)).*2.0)./lB-((((z+LB.*sin(q2)).*(dx-LB.*dq2.*sin(q2).*cos(alphaAB-pi./2.0)))./lB-((dz+LB.*dq2.*sin(pi./2.0).*cos(q2)).*(x+aB.*sin(alphaAB)-eB.*sin(alphaAB)+LB.*cos(q2).*sin(alphaAB)))./lB).*((IlBxy.*((LB.*sin(alphaAB-pi./2.0).*sin(q2).*(dz+LB.*dq2.*cos(q2)))./lB-(LB.*sin(pi./2.0).*cos(q2).*(dy-LB.*dq2.*cos(alphaAB).*sin(q2)))./lB+(LB.*dq2.*sin(alphaAB-pi./2.0).*cos(q2).*(z+LB.*sin(q2)))./lB+(LB.*dq2.*sin(pi./2.0).*sin(q2).*(y+aB.*cos(alphaAB)-eB.*cos(alphaAB)+LB.*cos(alphaAB).*cos(q2)))./lB))./(lB.*2.0)+(IlByy.*((LB.*sin(pi./2.0).*cos(q2).*(dx-LB.*dq2.*sin(alphaAB).*sin(q2)))./lB+(LB.*sin(q2).*cos(alphaAB-pi./2.0).*(dz+LB.*dq2.*cos(q2)))./lB+(LB.*dq2.*cos(q2).*cos(alphaAB-pi./2.0).*(z+LB.*sin(q2)))./lB-(LB.*dq2.*sin(pi./2.0).*sin(q2).*(x+aB.*sin(alphaAB)-eB.*sin(alphaAB)+LB.*cos(q2).*sin(alphaAB)))./lB))./(lB.*2.0)-(IlByz.*((LB.*sin(q2).*cos(alphaAB-pi./2.0).*(dy-LB.*dq2.*cos(alphaAB).*sin(q2)))./lB+(LB.*sin(alphaAB-pi./2.0).*sin(q2).*(dx-LB.*dq2.*sin(alphaAB).*sin(q2)))./lB+(LB.*dq2.*sin(alphaAB-pi./2.0).*cos(q2).*(x+aB.*sin(alphaAB)-eB.*sin(alphaAB)+LB.*cos(q2).*sin(alphaAB)))./lB+(LB.*dq2.*cos(q2).*cos(alphaAB-pi./2.0).*(y+aB.*cos(alphaAB)-eB.*cos(alphaAB)+LB.*cos(alphaAB).*cos(q2)))./lB))./(lB.*2.0)).*2.0)./lB+(((LB.*sin(q2).*cos(alphaAB-pi./2.0).*(z+LB.*sin(q2)))./lB+(LB.*sin(pi./2.0).*cos(q2).*(x+aB.*sin(alphaAB)-eB.*sin(alphaAB)+LB.*cos(q2).*sin(alphaAB)))./lB).*((IlBxy.*(((dz+LB.*dq2.*cos(q2)).*(dy+LB.*dq2.*sin(alphaAB-pi./2.0).*sin(q2)))./lB-((dy-LB.*dq2.*cos(alphaAB).*sin(q2)).*(dz+LB.*dq2.*sin(pi./2.0).*cos(q2)))./lB+((z+LB.*sin(q2)).*(ddy+LB.*dq2.^2.*sin(alphaAB-pi./2.0).*cos(q2)+LB.*ddq2.*sin(alphaAB-pi./2.0).*sin(q2)))./lB-((ddz+LB.*ddq2.*sin(pi./2.0).*cos(q2)-LB.*dq2.^2.*sin(pi./2.0).*sin(q2)).*(y+aB.*cos(alphaAB)-eB.*cos(alphaAB)+LB.*cos(alphaAB).*cos(q2)))./lB))./(lB.*2.0)-(IlByz.*(-((dy-LB.*dq2.*cos(alphaAB).*sin(q2)).*(dx-LB.*dq2.*sin(q2).*cos(alphaAB-pi./2.0)))./lB+((dx-LB.*dq2.*sin(alphaAB).*sin(q2)).*(dy+LB.*dq2.*sin(alphaAB-pi./2.0).*sin(q2)))./lB+((ddy+LB.*dq2.^2.*sin(alphaAB-pi./2.0).*cos(q2)+LB.*ddq2.*sin(alphaAB-pi./2.0).*sin(q2)).*(x+aB.*sin(alphaAB)-eB.*sin(alphaAB)+LB.*cos(q2).*sin(alphaAB)))./lB+((-ddx+LB.*dq2.^2.*cos(q2).*cos(alphaAB-pi./2.0)+LB.*ddq2.*sin(q2).*cos(alphaAB-pi./2.0)).*(y+aB.*cos(alphaAB)-eB.*cos(alphaAB)+LB.*cos(alphaAB).*cos(q2)))./lB))./(lB.*2.0)+(IlByy.*(((ddz+LB.*ddq2.*sin(pi./2.0).*cos(q2)-LB.*dq2.^2.*sin(pi./2.0).*sin(q2)).*(x+aB.*sin(alphaAB)-eB.*sin(alphaAB)+LB.*cos(q2).*sin(alphaAB)))./lB-((dz+LB.*dq2.*cos(q2)).*(dx-LB.*dq2.*sin(q2).*cos(alphaAB-pi./2.0)))./lB+((dx-LB.*dq2.*sin(alphaAB).*sin(q2)).*(dz+LB.*dq2.*sin(pi./2.0).*cos(q2)))./lB+((z+LB.*sin(q2)).*(-ddx+LB.*dq2.^2.*cos(q2).*cos(alphaAB-pi./2.0)+LB.*ddq2.*sin(q2).*cos(alphaAB-pi./2.0)))./lB))./(lB.*2.0)).*2.0)./lB+(((IlBzz.*((LB.*sin(q2).*cos(alphaAB-pi./2.0).*(y+aB.*cos(alphaAB)-eB.*cos(alphaAB)+LB.*cos(alphaAB).*cos(q2)))./lB+(LB.*sin(alphaAB-pi./2.0).*sin(q2).*(x+aB.*sin(alphaAB)-eB.*sin(alphaAB)+LB.*cos(q2).*sin(alphaAB)))./lB))./(lB.*2.0)+(IlBxz.*((LB.*sin(pi./2.0).*cos(q2).*(y+aB.*cos(alphaAB)-eB.*cos(alphaAB)+LB.*cos(alphaAB).*cos(q2)))./lB-(LB.*sin(alphaAB-pi./2.0).*sin(q2).*(z+LB.*sin(q2)))./lB))./(lB.*2.0)-(IlByz.*((LB.*sin(q2).*cos(alphaAB-pi./2.0).*(z+LB.*sin(q2)))./lB+(LB.*sin(pi./2.0).*cos(q2).*(x+aB.*sin(alphaAB)-eB.*sin(alphaAB)+LB.*cos(q2).*sin(alphaAB)))./lB))./(lB.*2.0)).*(-((dy-LB.*dq2.*cos(alphaAB).*sin(q2)).*(dx-LB.*dq2.*sin(q2).*cos(alphaAB-pi./2.0)))./lB+((dx-LB.*dq2.*sin(alphaAB).*sin(q2)).*(dy+LB.*dq2.*sin(alphaAB-pi./2.0).*sin(q2)))./lB+((ddy+LB.*dq2.^2.*sin(alphaAB-pi./2.0).*cos(q2)+LB.*ddq2.*sin(alphaAB-pi./2.0).*sin(q2)).*(x+aB.*sin(alphaAB)-eB.*sin(alphaAB)+LB.*cos(q2).*sin(alphaAB)))./lB+((-ddx+LB.*dq2.^2.*cos(q2).*cos(alphaAB-pi./2.0)+LB.*ddq2.*sin(q2).*cos(alphaAB-pi./2.0)).*(y+aB.*cos(alphaAB)-eB.*cos(alphaAB)+LB.*cos(alphaAB).*cos(q2)))./lB).*2.0)./lB-(((IlByz.*((LB.*sin(q2).*cos(alphaAB-pi./2.0).*(y+aB.*cos(alphaAB)-eB.*cos(alphaAB)+LB.*cos(alphaAB).*cos(q2)))./lB+(LB.*sin(alphaAB-pi./2.0).*sin(q2).*(x+aB.*sin(alphaAB)-eB.*sin(alphaAB)+LB.*cos(q2).*sin(alphaAB)))./lB))./(lB.*2.0)+(IlBxy.*((LB.*sin(pi./2.0).*cos(q2).*(y+aB.*cos(alphaAB)-eB.*cos(alphaAB)+LB.*cos(alphaAB).*cos(q2)))./lB-(LB.*sin(alphaAB-pi./2.0).*sin(q2).*(z+LB.*sin(q2)))./lB))./(lB.*2.0)-(IlByy.*((LB.*sin(q2).*cos(alphaAB-pi./2.0).*(z+LB.*sin(q2)))./lB+(LB.*sin(pi./2.0).*cos(q2).*(x+aB.*sin(alphaAB)-eB.*sin(alphaAB)+LB.*cos(q2).*sin(alphaAB)))./lB))./(lB.*2.0)).*(((ddz+LB.*ddq2.*sin(pi./2.0).*cos(q2)-LB.*dq2.^2.*sin(pi./2.0).*sin(q2)).*(x+aB.*sin(alphaAB)-eB.*sin(alphaAB)+LB.*cos(q2).*sin(alphaAB)))./lB-((dz+LB.*dq2.*cos(q2)).*(dx-LB.*dq2.*sin(q2).*cos(alphaAB-pi./2.0)))./lB+((dx-LB.*dq2.*sin(alphaAB).*sin(q2)).*(dz+LB.*dq2.*sin(pi./2.0).*cos(q2)))./lB+((z+LB.*sin(q2)).*(-ddx+LB.*dq2.^2.*cos(q2).*cos(alphaAB-pi./2.0)+LB.*ddq2.*sin(q2).*cos(alphaAB-pi./2.0)))./lB).*2.0)./lB+(LB.*g.*mLB.*cos(q2))./2.0+LB.*g.*mlB.*cos(q2)-(LB.*mlB.*sin(pi./2.0).*cos(q2).*(ddz./2.0-(LB.*ddq2.*sin(pi./2.0).*cos(q2))./2.0+(LB.*dq2.^2.*sin(pi./2.0).*sin(q2))./2.0))./2.0-LB.*mlB.*sin(pi./2.0).*cos(q2).*(ddz./4.0-(LB.*ddq2.*sin(pi./2.0).*cos(q2))./4.0+(LB.*dq2.^2.*sin(pi./2.0).*sin(q2))./4.0)+(LB.*mlB.*sin(q2).*cos(alphaAB-pi./2.0).*(ddx./2.0+(LB.*dq2.^2.*cos(q2).*cos(alphaAB-pi./2.0))./2.0+(LB.*ddq2.*sin(q2).*cos(alphaAB-pi./2.0))./2.0))./2.0+LB.*mlB.*sin(q2).*cos(alphaAB-pi./2.0).*(ddx./4.0+(LB.*dq2.^2.*cos(q2).*cos(alphaAB-pi./2.0))./4.0+(LB.*ddq2.*sin(q2).*cos(alphaAB-pi./2.0))./4.0)+(LB.*mlB.*sin(alphaAB-pi./2.0).*sin(q2).*(ddy.*(-1.0./2.0)+(LB.*dq2.^2.*sin(alphaAB-pi./2.0).*cos(q2))./2.0+(LB.*ddq2.*sin(alphaAB-pi./2.0).*sin(q2))./2.0))./2.0+LB.*mlB.*sin(alphaAB-pi./2.0).*sin(q2).*(ddy.*(-1.0./4.0)+(LB.*dq2.^2.*sin(alphaAB-pi./2.0).*cos(q2))./4.0+(LB.*ddq2.*sin(alphaAB-pi./2.0).*sin(q2))./4.0);ddq3.*(ILCxx.*sin(alphaAC-pi./2.0).^2+ILCyy.*cos(alphaAC-pi./2.0).^2+ILCxy.*sin(alphaAC-pi./2.0).*cos(alphaAC-pi./2.0).*2.0)+((((dx-LC.*dq3.*sin(q3).*cos(alphaAC-pi./2.0)).*(y+aC.*cos(alphaAC)-eC.*cos(alphaAC)+LC.*cos(alphaAC).*cos(q3)))./lC-((dy+LC.*dq3.*sin(alphaAC-pi./2.0).*sin(q3)).*(x+aC.*sin(alphaAC)-eC.*sin(alphaAC)+LC.*cos(q3).*sin(alphaAC)))./lC).*((IlCxz.*((LC.*cos(q3).*(dy+LC.*dq3.*sin(alphaAC-pi./2.0).*sin(q3)))./lC+(LC.*cos(alphaAC).*sin(q3).*(dz+LC.*dq3.*sin(pi./2.0).*cos(q3)))./lC+(LC.*dq3.*sin(alphaAC-pi./2.0).*cos(q3).*(z+LC.*sin(q3)))./lC+(LC.*dq3.*sin(pi./2.0).*sin(q3).*(y+aC.*cos(alphaAC)-eC.*cos(alphaAC)+LC.*cos(alphaAC).*cos(q3)))./lC).*(-1.0./2.0))./lC+(IlCyz.*((LC.*cos(q3).*(dx-LC.*dq3.*sin(q3).*cos(alphaAC-pi./2.0)))./lC+(LC.*sin(alphaAC).*sin(q3).*(dz+LC.*dq3.*sin(pi./2.0).*cos(q3)))./lC-(LC.*dq3.*cos(q3).*cos(alphaAC-pi./2.0).*(z+LC.*sin(q3)))./lC+(LC.*dq3.*sin(pi./2.0).*sin(q3).*(x+aC.*sin(alphaAC)-eC.*sin(alphaAC)+LC.*cos(q3).*sin(alphaAC)))./lC))./(lC.*2.0)+(IlCzz.*((LC.*cos(alphaAC).*sin(q3).*(dx-LC.*dq3.*sin(q3).*cos(alphaAC-pi./2.0)))./lC-(LC.*sin(alphaAC).*sin(q3).*(dy+LC.*dq3.*sin(alphaAC-pi./2.0).*sin(q3)))./lC+(LC.*dq3.*sin(alphaAC-pi./2.0).*cos(q3).*(x+aC.*sin(alphaAC)-eC.*sin(alphaAC)+LC.*cos(q3).*sin(alphaAC)))./lC+(LC.*dq3.*cos(q3).*cos(alphaAC-pi./2.0).*(y+aC.*cos(alphaAC)-eC.*cos(alphaAC)+LC.*cos(alphaAC).*cos(q3)))./lC))./(lC.*2.0)).*2.0)./lC+((((dx-LC.*dq3.*sin(q3).*cos(alphaAC-pi./2.0)).*(y+aC.*cos(alphaAC)-eC.*cos(alphaAC)+LC.*cos(alphaAC).*cos(q3)))./lC-((dy+LC.*dq3.*sin(alphaAC-pi./2.0).*sin(q3)).*(x+aC.*sin(alphaAC)-eC.*sin(alphaAC)+LC.*cos(q3).*sin(alphaAC)))./lC).*((IlCxz.*((LC.*sin(alphaAC-pi./2.0).*sin(q3).*(dz+LC.*dq3.*cos(q3)))./lC-(LC.*sin(pi./2.0).*cos(q3).*(dy-LC.*dq3.*cos(alphaAC).*sin(q3)))./lC+(LC.*dq3.*sin(alphaAC-pi./2.0).*cos(q3).*(z+LC.*sin(q3)))./lC+(LC.*dq3.*sin(pi./2.0).*sin(q3).*(y+aC.*cos(alphaAC)-eC.*cos(alphaAC)+LC.*cos(alphaAC).*cos(q3)))./lC))./(lC.*2.0)+(IlCyz.*((LC.*sin(pi./2.0).*cos(q3).*(dx-LC.*dq3.*sin(alphaAC).*sin(q3)))./lC+(LC.*sin(q3).*cos(alphaAC-pi./2.0).*(dz+LC.*dq3.*cos(q3)))./lC+(LC.*dq3.*cos(q3).*cos(alphaAC-pi./2.0).*(z+LC.*sin(q3)))./lC-(LC.*dq3.*sin(pi./2.0).*sin(q3).*(x+aC.*sin(alphaAC)-eC.*sin(alphaAC)+LC.*cos(q3).*sin(alphaAC)))./lC))./(lC.*2.0)-(IlCzz.*((LC.*sin(q3).*cos(alphaAC-pi./2.0).*(dy-LC.*dq3.*cos(alphaAC).*sin(q3)))./lC+(LC.*sin(alphaAC-pi./2.0).*sin(q3).*(dx-LC.*dq3.*sin(alphaAC).*sin(q3)))./lC+(LC.*dq3.*sin(alphaAC-pi./2.0).*cos(q3).*(x+aC.*sin(alphaAC)-eC.*sin(alphaAC)+LC.*cos(q3).*sin(alphaAC)))./lC+(LC.*dq3.*cos(q3).*cos(alphaAC-pi./2.0).*(y+aC.*cos(alphaAC)-eC.*cos(alphaAC)+LC.*cos(alphaAC).*cos(q3)))./lC))./(lC.*2.0)).*2.0)./lC-(((LC.*sin(q3).*cos(alphaAC-pi./2.0).*(y+aC.*cos(alphaAC)-eC.*cos(alphaAC)+LC.*cos(alphaAC).*cos(q3)))./lC+(LC.*sin(alphaAC-pi./2.0).*sin(q3).*(x+aC.*sin(alphaAC)-eC.*sin(alphaAC)+LC.*cos(q3).*sin(alphaAC)))./lC).*((IlCxz.*(((dz+LC.*dq3.*cos(q3)).*(dy+LC.*dq3.*sin(alphaAC-pi./2.0).*sin(q3)))./lC-((dy-LC.*dq3.*cos(alphaAC).*sin(q3)).*(dz+LC.*dq3.*sin(pi./2.0).*cos(q3)))./lC+((z+LC.*sin(q3)).*(ddy+LC.*dq3.^2.*sin(alphaAC-pi./2.0).*cos(q3)+LC.*ddq3.*sin(alphaAC-pi./2.0).*sin(q3)))./lC-((ddz+LC.*ddq3.*sin(pi./2.0).*cos(q3)-LC.*dq3.^2.*sin(pi./2.0).*sin(q3)).*(y+aC.*cos(alphaAC)-eC.*cos(alphaAC)+LC.*cos(alphaAC).*cos(q3)))./lC))./(lC.*2.0)-(IlCzz.*(-((dy-LC.*dq3.*cos(alphaAC).*sin(q3)).*(dx-LC.*dq3.*sin(q3).*cos(alphaAC-pi./2.0)))./lC+((dx-LC.*dq3.*sin(alphaAC).*sin(q3)).*(dy+LC.*dq3.*sin(alphaAC-pi./2.0).*sin(q3)))./lC+((ddy+LC.*dq3.^2.*sin(alphaAC-pi./2.0).*cos(q3)+LC.*ddq3.*sin(alphaAC-pi./2.0).*sin(q3)).*(x+aC.*sin(alphaAC)-eC.*sin(alphaAC)+LC.*cos(q3).*sin(alphaAC)))./lC+((-ddx+LC.*dq3.^2.*cos(q3).*cos(alphaAC-pi./2.0)+LC.*ddq3.*sin(q3).*cos(alphaAC-pi./2.0)).*(y+aC.*cos(alphaAC)-eC.*cos(alphaAC)+LC.*cos(alphaAC).*cos(q3)))./lC))./(lC.*2.0)+(IlCyz.*(((ddz+LC.*ddq3.*sin(pi./2.0).*cos(q3)-LC.*dq3.^2.*sin(pi./2.0).*sin(q3)).*(x+aC.*sin(alphaAC)-eC.*sin(alphaAC)+LC.*cos(q3).*sin(alphaAC)))./lC-((dz+LC.*dq3.*cos(q3)).*(dx-LC.*dq3.*sin(q3).*cos(alphaAC-pi./2.0)))./lC+((dx-LC.*dq3.*sin(alphaAC).*sin(q3)).*(dz+LC.*dq3.*sin(pi./2.0).*cos(q3)))./lC+((z+LC.*sin(q3)).*(-ddx+LC.*dq3.^2.*cos(q3).*cos(alphaAC-pi./2.0)+LC.*ddq3.*sin(q3).*cos(alphaAC-pi./2.0)))./lC))./(lC.*2.0)).*2.0)./lC+(((IlCxz.*(((dx-LC.*dq3.*sin(q3).*cos(alphaAC-pi./2.0)).*(y+aC.*cos(alphaAC)-eC.*cos(alphaAC)+LC.*cos(alphaAC).*cos(q3)))./lC-((dy+LC.*dq3.*sin(alphaAC-pi./2.0).*sin(q3)).*(x+aC.*sin(alphaAC)-eC.*sin(alphaAC)+LC.*cos(q3).*sin(alphaAC)))./lC).*(-1.0./2.0))./lC+(IlCxx.*(((dz+LC.*dq3.*sin(pi./2.0).*cos(q3)).*(y+aC.*cos(alphaAC)-eC.*cos(alphaAC)+LC.*cos(alphaAC).*cos(q3)))./lC-((z+LC.*sin(q3)).*(dy+LC.*dq3.*sin(alphaAC-pi./2.0).*sin(q3)))./lC))./(lC.*2.0)+(IlCxy.*(((z+LC.*sin(q3)).*(dx-LC.*dq3.*sin(q3).*cos(alphaAC-pi./2.0)))./lC-((dz+LC.*dq3.*sin(pi./2.0).*cos(q3)).*(x+aC.*sin(alphaAC)-eC.*sin(alphaAC)+LC.*cos(q3).*sin(alphaAC)))./lC))./(lC.*2.0)).*((LC.*cos(q3).*(dy+LC.*dq3.*sin(alphaAC-pi./2.0).*sin(q3)))./lC+(LC.*cos(alphaAC).*sin(q3).*(dz+LC.*dq3.*sin(pi./2.0).*cos(q3)))./lC+(LC.*dq3.*sin(alphaAC-pi./2.0).*cos(q3).*(z+LC.*sin(q3)))./lC+(LC.*dq3.*sin(pi./2.0).*sin(q3).*(y+aC.*cos(alphaAC)-eC.*cos(alphaAC)+LC.*cos(alphaAC).*cos(q3)))./lC).*2.0)./lC-(((IlCxz.*(((dx-LC.*dq3.*sin(q3).*cos(alphaAC-pi./2.0)).*(y+aC.*cos(alphaAC)-eC.*cos(alphaAC)+LC.*cos(alphaAC).*cos(q3)))./lC-((dy+LC.*dq3.*sin(alphaAC-pi./2.0).*sin(q3)).*(x+aC.*sin(alphaAC)-eC.*sin(alphaAC)+LC.*cos(q3).*sin(alphaAC)))./lC).*(-1.0./2.0))./lC+(IlCxx.*(((dz+LC.*dq3.*sin(pi./2.0).*cos(q3)).*(y+aC.*cos(alphaAC)-eC.*cos(alphaAC)+LC.*cos(alphaAC).*cos(q3)))./lC-((z+LC.*sin(q3)).*(dy+LC.*dq3.*sin(alphaAC-pi./2.0).*sin(q3)))./lC))./(lC.*2.0)+(IlCxy.*(((z+LC.*sin(q3)).*(dx-LC.*dq3.*sin(q3).*cos(alphaAC-pi./2.0)))./lC-((dz+LC.*dq3.*sin(pi./2.0).*cos(q3)).*(x+aC.*sin(alphaAC)-eC.*sin(alphaAC)+LC.*cos(q3).*sin(alphaAC)))./lC))./(lC.*2.0)).*((LC.*sin(alphaAC-pi./2.0).*sin(q3).*(dz+LC.*dq3.*cos(q3)))./lC-(LC.*sin(pi./2.0).*cos(q3).*(dy-LC.*dq3.*cos(alphaAC).*sin(q3)))./lC+(LC.*dq3.*sin(alphaAC-pi./2.0).*cos(q3).*(z+LC.*sin(q3)))./lC+(LC.*dq3.*sin(pi./2.0).*sin(q3).*(y+aC.*cos(alphaAC)-eC.*cos(alphaAC)+LC.*cos(alphaAC).*cos(q3)))./lC).*2.0)./lC-(((IlCxz.*((LC.*sin(q3).*cos(alphaAC-pi./2.0).*(y+aC.*cos(alphaAC)-eC.*cos(alphaAC)+LC.*cos(alphaAC).*cos(q3)))./lC+(LC.*sin(alphaAC-pi./2.0).*sin(q3).*(x+aC.*sin(alphaAC)-eC.*sin(alphaAC)+LC.*cos(q3).*sin(alphaAC)))./lC))./(lC.*2.0)+(IlCxx.*((LC.*sin(pi./2.0).*cos(q3).*(y+aC.*cos(alphaAC)-eC.*cos(alphaAC)+LC.*cos(alphaAC).*cos(q3)))./lC-(LC.*sin(alphaAC-pi./2.0).*sin(q3).*(z+LC.*sin(q3)))./lC))./(lC.*2.0)-(IlCxy.*((LC.*sin(q3).*cos(alphaAC-pi./2.0).*(z+LC.*sin(q3)))./lC+(LC.*sin(pi./2.0).*cos(q3).*(x+aC.*sin(alphaAC)-eC.*sin(alphaAC)+LC.*cos(q3).*sin(alphaAC)))./lC))./(lC.*2.0)).*(((dz+LC.*dq3.*cos(q3)).*(dy+LC.*dq3.*sin(alphaAC-pi./2.0).*sin(q3)))./lC-((dy-LC.*dq3.*cos(alphaAC).*sin(q3)).*(dz+LC.*dq3.*sin(pi./2.0).*cos(q3)))./lC+((z+LC.*sin(q3)).*(ddy+LC.*dq3.^2.*sin(alphaAC-pi./2.0).*cos(q3)+LC.*ddq3.*sin(alphaAC-pi./2.0).*sin(q3)))./lC-((ddz+LC.*ddq3.*sin(pi./2.0).*cos(q3)-LC.*dq3.^2.*sin(pi./2.0).*sin(q3)).*(y+aC.*cos(alphaAC)-eC.*cos(alphaAC)+LC.*cos(alphaAC).*cos(q3)))./lC).*2.0)./lC-(((IlCyz.*(((dx-LC.*dq3.*sin(q3).*cos(alphaAC-pi./2.0)).*(y+aC.*cos(alphaAC)-eC.*cos(alphaAC)+LC.*cos(alphaAC).*cos(q3)))./lC-((dy+LC.*dq3.*sin(alphaAC-pi./2.0).*sin(q3)).*(x+aC.*sin(alphaAC)-eC.*sin(alphaAC)+LC.*cos(q3).*sin(alphaAC)))./lC).*(-1.0./2.0))./lC+(IlCxy.*(((dz+LC.*dq3.*sin(pi./2.0).*cos(q3)).*(y+aC.*cos(alphaAC)-eC.*cos(alphaAC)+LC.*cos(alphaAC).*cos(q3)))./lC-((z+LC.*sin(q3)).*(dy+LC.*dq3.*sin(alphaAC-pi./2.0).*sin(q3)))./lC))./(lC.*2.0)+(IlCyy.*(((z+LC.*sin(q3)).*(dx-LC.*dq3.*sin(q3).*cos(alphaAC-pi./2.0)))./lC-((dz+LC.*dq3.*sin(pi./2.0).*cos(q3)).*(x+aC.*sin(alphaAC)-eC.*sin(alphaAC)+LC.*cos(q3).*sin(alphaAC)))./lC))./(lC.*2.0)).*((LC.*cos(q3).*(dx-LC.*dq3.*sin(q3).*cos(alphaAC-pi./2.0)))./lC+(LC.*sin(alphaAC).*sin(q3).*(dz+LC.*dq3.*sin(pi./2.0).*cos(q3)))./lC-(LC.*dq3.*cos(q3).*cos(alphaAC-pi./2.0).*(z+LC.*sin(q3)))./lC+(LC.*dq3.*sin(pi./2.0).*sin(q3).*(x+aC.*sin(alphaAC)-eC.*sin(alphaAC)+LC.*cos(q3).*sin(alphaAC)))./lC).*2.0)./lC-(((IlCyz.*(((dx-LC.*dq3.*sin(q3).*cos(alphaAC-pi./2.0)).*(y+aC.*cos(alphaAC)-eC.*cos(alphaAC)+LC.*cos(alphaAC).*cos(q3)))./lC-((dy+LC.*dq3.*sin(alphaAC-pi./2.0).*sin(q3)).*(x+aC.*sin(alphaAC)-eC.*sin(alphaAC)+LC.*cos(q3).*sin(alphaAC)))./lC).*(-1.0./2.0))./lC+(IlCxy.*(((dz+LC.*dq3.*sin(pi./2.0).*cos(q3)).*(y+aC.*cos(alphaAC)-eC.*cos(alphaAC)+LC.*cos(alphaAC).*cos(q3)))./lC-((z+LC.*sin(q3)).*(dy+LC.*dq3.*sin(alphaAC-pi./2.0).*sin(q3)))./lC))./(lC.*2.0)+(IlCyy.*(((z+LC.*sin(q3)).*(dx-LC.*dq3.*sin(q3).*cos(alphaAC-pi./2.0)))./lC-((dz+LC.*dq3.*sin(pi./2.0).*cos(q3)).*(x+aC.*sin(alphaAC)-eC.*sin(alphaAC)+LC.*cos(q3).*sin(alphaAC)))./lC))./(lC.*2.0)).*((LC.*sin(pi./2.0).*cos(q3).*(dx-LC.*dq3.*sin(alphaAC).*sin(q3)))./lC+(LC.*sin(q3).*cos(alphaAC-pi./2.0).*(dz+LC.*dq3.*cos(q3)))./lC+(LC.*dq3.*cos(q3).*cos(alphaAC-pi./2.0).*(z+LC.*sin(q3)))./lC-(LC.*dq3.*sin(pi./2.0).*sin(q3).*(x+aC.*sin(alphaAC)-eC.*sin(alphaAC)+LC.*cos(q3).*sin(alphaAC)))./lC).*2.0)./lC-((((dz+LC.*dq3.*sin(pi./2.0).*cos(q3)).*(y+aC.*cos(alphaAC)-eC.*cos(alphaAC)+LC.*cos(alphaAC).*cos(q3)))./lC-((z+LC.*sin(q3)).*(dy+LC.*dq3.*sin(alphaAC-pi./2.0).*sin(q3)))./lC).*((IlCxx.*((LC.*cos(q3).*(dy+LC.*dq3.*sin(alphaAC-pi./2.0).*sin(q3)))./lC+(LC.*cos(alphaAC).*sin(q3).*(dz+LC.*dq3.*sin(pi./2.0).*cos(q3)))./lC+(LC.*dq3.*sin(alphaAC-pi./2.0).*cos(q3).*(z+LC.*sin(q3)))./lC+(LC.*dq3.*sin(pi./2.0).*sin(q3).*(y+aC.*cos(alphaAC)-eC.*cos(alphaAC)+LC.*cos(alphaAC).*cos(q3)))./lC).*(-1.0./2.0))./lC+(IlCxy.*((LC.*cos(q3).*(dx-LC.*dq3.*sin(q3).*cos(alphaAC-pi./2.0)))./lC+(LC.*sin(alphaAC).*sin(q3).*(dz+LC.*dq3.*sin(pi./2.0).*cos(q3)))./lC-(LC.*dq3.*cos(q3).*cos(alphaAC-pi./2.0).*(z+LC.*sin(q3)))./lC+(LC.*dq3.*sin(pi./2.0).*sin(q3).*(x+aC.*sin(alphaAC)-eC.*sin(alphaAC)+LC.*cos(q3).*sin(alphaAC)))./lC))./(lC.*2.0)+(IlCxz.*((LC.*cos(alphaAC).*sin(q3).*(dx-LC.*dq3.*sin(q3).*cos(alphaAC-pi./2.0)))./lC-(LC.*sin(alphaAC).*sin(q3).*(dy+LC.*dq3.*sin(alphaAC-pi./2.0).*sin(q3)))./lC+(LC.*dq3.*sin(alphaAC-pi./2.0).*cos(q3).*(x+aC.*sin(alphaAC)-eC.*sin(alphaAC)+LC.*cos(q3).*sin(alphaAC)))./lC+(LC.*dq3.*cos(q3).*cos(alphaAC-pi./2.0).*(y+aC.*cos(alphaAC)-eC.*cos(alphaAC)+LC.*cos(alphaAC).*cos(q3)))./lC))./(lC.*2.0)).*2.0)./lC-((((dz+LC.*dq3.*sin(pi./2.0).*cos(q3)).*(y+aC.*cos(alphaAC)-eC.*cos(alphaAC)+LC.*cos(alphaAC).*cos(q3)))./lC-((z+LC.*sin(q3)).*(dy+LC.*dq3.*sin(alphaAC-pi./2.0).*sin(q3)))./lC).*((IlCxx.*((LC.*sin(alphaAC-pi./2.0).*sin(q3).*(dz+LC.*dq3.*cos(q3)))./lC-(LC.*sin(pi./2.0).*cos(q3).*(dy-LC.*dq3.*cos(alphaAC).*sin(q3)))./lC+(LC.*dq3.*sin(alphaAC-pi./2.0).*cos(q3).*(z+LC.*sin(q3)))./lC+(LC.*dq3.*sin(pi./2.0).*sin(q3).*(y+aC.*cos(alphaAC)-eC.*cos(alphaAC)+LC.*cos(alphaAC).*cos(q3)))./lC))./(lC.*2.0)+(IlCxy.*((LC.*sin(pi./2.0).*cos(q3).*(dx-LC.*dq3.*sin(alphaAC).*sin(q3)))./lC+(LC.*sin(q3).*cos(alphaAC-pi./2.0).*(dz+LC.*dq3.*cos(q3)))./lC+(LC.*dq3.*cos(q3).*cos(alphaAC-pi./2.0).*(z+LC.*sin(q3)))./lC-(LC.*dq3.*sin(pi./2.0).*sin(q3).*(x+aC.*sin(alphaAC)-eC.*sin(alphaAC)+LC.*cos(q3).*sin(alphaAC)))./lC))./(lC.*2.0)-(IlCxz.*((LC.*sin(q3).*cos(alphaAC-pi./2.0).*(dy-LC.*dq3.*cos(alphaAC).*sin(q3)))./lC+(LC.*sin(alphaAC-pi./2.0).*sin(q3).*(dx-LC.*dq3.*sin(alphaAC).*sin(q3)))./lC+(LC.*dq3.*sin(alphaAC-pi./2.0).*cos(q3).*(x+aC.*sin(alphaAC)-eC.*sin(alphaAC)+LC.*cos(q3).*sin(alphaAC)))./lC+(LC.*dq3.*cos(q3).*cos(alphaAC-pi./2.0).*(y+aC.*cos(alphaAC)-eC.*cos(alphaAC)+LC.*cos(alphaAC).*cos(q3)))./lC))./(lC.*2.0)).*2.0)./lC-(((LC.*sin(pi./2.0).*cos(q3).*(y+aC.*cos(alphaAC)-eC.*cos(alphaAC)+LC.*cos(alphaAC).*cos(q3)))./lC-(LC.*sin(alphaAC-pi./2.0).*sin(q3).*(z+LC.*sin(q3)))./lC).*((IlCxx.*(((dz+LC.*dq3.*cos(q3)).*(dy+LC.*dq3.*sin(alphaAC-pi./2.0).*sin(q3)))./lC-((dy-LC.*dq3.*cos(alphaAC).*sin(q3)).*(dz+LC.*dq3.*sin(pi./2.0).*cos(q3)))./lC+((z+LC.*sin(q3)).*(ddy+LC.*dq3.^2.*sin(alphaAC-pi./2.0).*cos(q3)+LC.*ddq3.*sin(alphaAC-pi./2.0).*sin(q3)))./lC-((ddz+LC.*ddq3.*sin(pi./2.0).*cos(q3)-LC.*dq3.^2.*sin(pi./2.0).*sin(q3)).*(y+aC.*cos(alphaAC)-eC.*cos(alphaAC)+LC.*cos(alphaAC).*cos(q3)))./lC))./(lC.*2.0)-(IlCxz.*(-((dy-LC.*dq3.*cos(alphaAC).*sin(q3)).*(dx-LC.*dq3.*sin(q3).*cos(alphaAC-pi./2.0)))./lC+((dx-LC.*dq3.*sin(alphaAC).*sin(q3)).*(dy+LC.*dq3.*sin(alphaAC-pi./2.0).*sin(q3)))./lC+((ddy+LC.*dq3.^2.*sin(alphaAC-pi./2.0).*cos(q3)+LC.*ddq3.*sin(alphaAC-pi./2.0).*sin(q3)).*(x+aC.*sin(alphaAC)-eC.*sin(alphaAC)+LC.*cos(q3).*sin(alphaAC)))./lC+((-ddx+LC.*dq3.^2.*cos(q3).*cos(alphaAC-pi./2.0)+LC.*ddq3.*sin(q3).*cos(alphaAC-pi./2.0)).*(y+aC.*cos(alphaAC)-eC.*cos(alphaAC)+LC.*cos(alphaAC).*cos(q3)))./lC))./(lC.*2.0)+(IlCxy.*(((ddz+LC.*ddq3.*sin(pi./2.0).*cos(q3)-LC.*dq3.^2.*sin(pi./2.0).*sin(q3)).*(x+aC.*sin(alphaAC)-eC.*sin(alphaAC)+LC.*cos(q3).*sin(alphaAC)))./lC-((dz+LC.*dq3.*cos(q3)).*(dx-LC.*dq3.*sin(q3).*cos(alphaAC-pi./2.0)))./lC+((dx-LC.*dq3.*sin(alphaAC).*sin(q3)).*(dz+LC.*dq3.*sin(pi./2.0).*cos(q3)))./lC+((z+LC.*sin(q3)).*(-ddx+LC.*dq3.^2.*cos(q3).*cos(alphaAC-pi./2.0)+LC.*ddq3.*sin(q3).*cos(alphaAC-pi./2.0)))./lC))./(lC.*2.0)).*2.0)./lC-(((IlCzz.*(((dx-LC.*dq3.*sin(q3).*cos(alphaAC-pi./2.0)).*(y+aC.*cos(alphaAC)-eC.*cos(alphaAC)+LC.*cos(alphaAC).*cos(q3)))./lC-((dy+LC.*dq3.*sin(alphaAC-pi./2.0).*sin(q3)).*(x+aC.*sin(alphaAC)-eC.*sin(alphaAC)+LC.*cos(q3).*sin(alphaAC)))./lC).*(-1.0./2.0))./lC+(IlCxz.*(((dz+LC.*dq3.*sin(pi./2.0).*cos(q3)).*(y+aC.*cos(alphaAC)-eC.*cos(alphaAC)+LC.*cos(alphaAC).*cos(q3)))./lC-((z+LC.*sin(q3)).*(dy+LC.*dq3.*sin(alphaAC-pi./2.0).*sin(q3)))./lC))./(lC.*2.0)+(IlCyz.*(((z+LC.*sin(q3)).*(dx-LC.*dq3.*sin(q3).*cos(alphaAC-pi./2.0)))./lC-((dz+LC.*dq3.*sin(pi./2.0).*cos(q3)).*(x+aC.*sin(alphaAC)-eC.*sin(alphaAC)+LC.*cos(q3).*sin(alphaAC)))./lC))./(lC.*2.0)).*((LC.*cos(alphaAC).*sin(q3).*(dx-LC.*dq3.*sin(q3).*cos(alphaAC-pi./2.0)))./lC-(LC.*sin(alphaAC).*sin(q3).*(dy+LC.*dq3.*sin(alphaAC-pi./2.0).*sin(q3)))./lC+(LC.*dq3.*sin(alphaAC-pi./2.0).*cos(q3).*(x+aC.*sin(alphaAC)-eC.*sin(alphaAC)+LC.*cos(q3).*sin(alphaAC)))./lC+(LC.*dq3.*cos(q3).*cos(alphaAC-pi./2.0).*(y+aC.*cos(alphaAC)-eC.*cos(alphaAC)+LC.*cos(alphaAC).*cos(q3)))./lC).*2.0)./lC+(((IlCzz.*(((dx-LC.*dq3.*sin(q3).*cos(alphaAC-pi./2.0)).*(y+aC.*cos(alphaAC)-eC.*cos(alphaAC)+LC.*cos(alphaAC).*cos(q3)))./lC-((dy+LC.*dq3.*sin(alphaAC-pi./2.0).*sin(q3)).*(x+aC.*sin(alphaAC)-eC.*sin(alphaAC)+LC.*cos(q3).*sin(alphaAC)))./lC).*(-1.0./2.0))./lC+(IlCxz.*(((dz+LC.*dq3.*sin(pi./2.0).*cos(q3)).*(y+aC.*cos(alphaAC)-eC.*cos(alphaAC)+LC.*cos(alphaAC).*cos(q3)))./lC-((z+LC.*sin(q3)).*(dy+LC.*dq3.*sin(alphaAC-pi./2.0).*sin(q3)))./lC))./(lC.*2.0)+(IlCyz.*(((z+LC.*sin(q3)).*(dx-LC.*dq3.*sin(q3).*cos(alphaAC-pi./2.0)))./lC-((dz+LC.*dq3.*sin(pi./2.0).*cos(q3)).*(x+aC.*sin(alphaAC)-eC.*sin(alphaAC)+LC.*cos(q3).*sin(alphaAC)))./lC))./(lC.*2.0)).*((LC.*sin(q3).*cos(alphaAC-pi./2.0).*(dy-LC.*dq3.*cos(alphaAC).*sin(q3)))./lC+(LC.*sin(alphaAC-pi./2.0).*sin(q3).*(dx-LC.*dq3.*sin(alphaAC).*sin(q3)))./lC+(LC.*dq3.*sin(alphaAC-pi./2.0).*cos(q3).*(x+aC.*sin(alphaAC)-eC.*sin(alphaAC)+LC.*cos(q3).*sin(alphaAC)))./lC+(LC.*dq3.*cos(q3).*cos(alphaAC-pi./2.0).*(y+aC.*cos(alphaAC)-eC.*cos(alphaAC)+LC.*cos(alphaAC).*cos(q3)))./lC).*2.0)./lC-((((z+LC.*sin(q3)).*(dx-LC.*dq3.*sin(q3).*cos(alphaAC-pi./2.0)))./lC-((dz+LC.*dq3.*sin(pi./2.0).*cos(q3)).*(x+aC.*sin(alphaAC)-eC.*sin(alphaAC)+LC.*cos(q3).*sin(alphaAC)))./lC).*((IlCxy.*((LC.*cos(q3).*(dy+LC.*dq3.*sin(alphaAC-pi./2.0).*sin(q3)))./lC+(LC.*cos(alphaAC).*sin(q3).*(dz+LC.*dq3.*sin(pi./2.0).*cos(q3)))./lC+(LC.*dq3.*sin(alphaAC-pi./2.0).*cos(q3).*(z+LC.*sin(q3)))./lC+(LC.*dq3.*sin(pi./2.0).*sin(q3).*(y+aC.*cos(alphaAC)-eC.*cos(alphaAC)+LC.*cos(alphaAC).*cos(q3)))./lC).*(-1.0./2.0))./lC+(IlCyy.*((LC.*cos(q3).*(dx-LC.*dq3.*sin(q3).*cos(alphaAC-pi./2.0)))./lC+(LC.*sin(alphaAC).*sin(q3).*(dz+LC.*dq3.*sin(pi./2.0).*cos(q3)))./lC-(LC.*dq3.*cos(q3).*cos(alphaAC-pi./2.0).*(z+LC.*sin(q3)))./lC+(LC.*dq3.*sin(pi./2.0).*sin(q3).*(x+aC.*sin(alphaAC)-eC.*sin(alphaAC)+LC.*cos(q3).*sin(alphaAC)))./lC))./(lC.*2.0)+(IlCyz.*((LC.*cos(alphaAC).*sin(q3).*(dx-LC.*dq3.*sin(q3).*cos(alphaAC-pi./2.0)))./lC-(LC.*sin(alphaAC).*sin(q3).*(dy+LC.*dq3.*sin(alphaAC-pi./2.0).*sin(q3)))./lC+(LC.*dq3.*sin(alphaAC-pi./2.0).*cos(q3).*(x+aC.*sin(alphaAC)-eC.*sin(alphaAC)+LC.*cos(q3).*sin(alphaAC)))./lC+(LC.*dq3.*cos(q3).*cos(alphaAC-pi./2.0).*(y+aC.*cos(alphaAC)-eC.*cos(alphaAC)+LC.*cos(alphaAC).*cos(q3)))./lC))./(lC.*2.0)).*2.0)./lC-((((z+LC.*sin(q3)).*(dx-LC.*dq3.*sin(q3).*cos(alphaAC-pi./2.0)))./lC-((dz+LC.*dq3.*sin(pi./2.0).*cos(q3)).*(x+aC.*sin(alphaAC)-eC.*sin(alphaAC)+LC.*cos(q3).*sin(alphaAC)))./lC).*((IlCxy.*((LC.*sin(alphaAC-pi./2.0).*sin(q3).*(dz+LC.*dq3.*cos(q3)))./lC-(LC.*sin(pi./2.0).*cos(q3).*(dy-LC.*dq3.*cos(alphaAC).*sin(q3)))./lC+(LC.*dq3.*sin(alphaAC-pi./2.0).*cos(q3).*(z+LC.*sin(q3)))./lC+(LC.*dq3.*sin(pi./2.0).*sin(q3).*(y+aC.*cos(alphaAC)-eC.*cos(alphaAC)+LC.*cos(alphaAC).*cos(q3)))./lC))./(lC.*2.0)+(IlCyy.*((LC.*sin(pi./2.0).*cos(q3).*(dx-LC.*dq3.*sin(alphaAC).*sin(q3)))./lC+(LC.*sin(q3).*cos(alphaAC-pi./2.0).*(dz+LC.*dq3.*cos(q3)))./lC+(LC.*dq3.*cos(q3).*cos(alphaAC-pi./2.0).*(z+LC.*sin(q3)))./lC-(LC.*dq3.*sin(pi./2.0).*sin(q3).*(x+aC.*sin(alphaAC)-eC.*sin(alphaAC)+LC.*cos(q3).*sin(alphaAC)))./lC))./(lC.*2.0)-(IlCyz.*((LC.*sin(q3).*cos(alphaAC-pi./2.0).*(dy-LC.*dq3.*cos(alphaAC).*sin(q3)))./lC+(LC.*sin(alphaAC-pi./2.0).*sin(q3).*(dx-LC.*dq3.*sin(alphaAC).*sin(q3)))./lC+(LC.*dq3.*sin(alphaAC-pi./2.0).*cos(q3).*(x+aC.*sin(alphaAC)-eC.*sin(alphaAC)+LC.*cos(q3).*sin(alphaAC)))./lC+(LC.*dq3.*cos(q3).*cos(alphaAC-pi./2.0).*(y+aC.*cos(alphaAC)-eC.*cos(alphaAC)+LC.*cos(alphaAC).*cos(q3)))./lC))./(lC.*2.0)).*2.0)./lC+(((LC.*sin(q3).*cos(alphaAC-pi./2.0).*(z+LC.*sin(q3)))./lC+(LC.*sin(pi./2.0).*cos(q3).*(x+aC.*sin(alphaAC)-eC.*sin(alphaAC)+LC.*cos(q3).*sin(alphaAC)))./lC).*((IlCxy.*(((dz+LC.*dq3.*cos(q3)).*(dy+LC.*dq3.*sin(alphaAC-pi./2.0).*sin(q3)))./lC-((dy-LC.*dq3.*cos(alphaAC).*sin(q3)).*(dz+LC.*dq3.*sin(pi./2.0).*cos(q3)))./lC+((z+LC.*sin(q3)).*(ddy+LC.*dq3.^2.*sin(alphaAC-pi./2.0).*cos(q3)+LC.*ddq3.*sin(alphaAC-pi./2.0).*sin(q3)))./lC-((ddz+LC.*ddq3.*sin(pi./2.0).*cos(q3)-LC.*dq3.^2.*sin(pi./2.0).*sin(q3)).*(y+aC.*cos(alphaAC)-eC.*cos(alphaAC)+LC.*cos(alphaAC).*cos(q3)))./lC))./(lC.*2.0)-(IlCyz.*(-((dy-LC.*dq3.*cos(alphaAC).*sin(q3)).*(dx-LC.*dq3.*sin(q3).*cos(alphaAC-pi./2.0)))./lC+((dx-LC.*dq3.*sin(alphaAC).*sin(q3)).*(dy+LC.*dq3.*sin(alphaAC-pi./2.0).*sin(q3)))./lC+((ddy+LC.*dq3.^2.*sin(alphaAC-pi./2.0).*cos(q3)+LC.*ddq3.*sin(alphaAC-pi./2.0).*sin(q3)).*(x+aC.*sin(alphaAC)-eC.*sin(alphaAC)+LC.*cos(q3).*sin(alphaAC)))./lC+((-ddx+LC.*dq3.^2.*cos(q3).*cos(alphaAC-pi./2.0)+LC.*ddq3.*sin(q3).*cos(alphaAC-pi./2.0)).*(y+aC.*cos(alphaAC)-eC.*cos(alphaAC)+LC.*cos(alphaAC).*cos(q3)))./lC))./(lC.*2.0)+(IlCyy.*(((ddz+LC.*ddq3.*sin(pi./2.0).*cos(q3)-LC.*dq3.^2.*sin(pi./2.0).*sin(q3)).*(x+aC.*sin(alphaAC)-eC.*sin(alphaAC)+LC.*cos(q3).*sin(alphaAC)))./lC-((dz+LC.*dq3.*cos(q3)).*(dx-LC.*dq3.*sin(q3).*cos(alphaAC-pi./2.0)))./lC+((dx-LC.*dq3.*sin(alphaAC).*sin(q3)).*(dz+LC.*dq3.*sin(pi./2.0).*cos(q3)))./lC+((z+LC.*sin(q3)).*(-ddx+LC.*dq3.^2.*cos(q3).*cos(alphaAC-pi./2.0)+LC.*ddq3.*sin(q3).*cos(alphaAC-pi./2.0)))./lC))./(lC.*2.0)).*2.0)./lC+(((IlCzz.*((LC.*sin(q3).*cos(alphaAC-pi./2.0).*(y+aC.*cos(alphaAC)-eC.*cos(alphaAC)+LC.*cos(alphaAC).*cos(q3)))./lC+(LC.*sin(alphaAC-pi./2.0).*sin(q3).*(x+aC.*sin(alphaAC)-eC.*sin(alphaAC)+LC.*cos(q3).*sin(alphaAC)))./lC))./(lC.*2.0)+(IlCxz.*((LC.*sin(pi./2.0).*cos(q3).*(y+aC.*cos(alphaAC)-eC.*cos(alphaAC)+LC.*cos(alphaAC).*cos(q3)))./lC-(LC.*sin(alphaAC-pi./2.0).*sin(q3).*(z+LC.*sin(q3)))./lC))./(lC.*2.0)-(IlCyz.*((LC.*sin(q3).*cos(alphaAC-pi./2.0).*(z+LC.*sin(q3)))./lC+(LC.*sin(pi./2.0).*cos(q3).*(x+aC.*sin(alphaAC)-eC.*sin(alphaAC)+LC.*cos(q3).*sin(alphaAC)))./lC))./(lC.*2.0)).*(-((dy-LC.*dq3.*cos(alphaAC).*sin(q3)).*(dx-LC.*dq3.*sin(q3).*cos(alphaAC-pi./2.0)))./lC+((dx-LC.*dq3.*sin(alphaAC).*sin(q3)).*(dy+LC.*dq3.*sin(alphaAC-pi./2.0).*sin(q3)))./lC+((ddy+LC.*dq3.^2.*sin(alphaAC-pi./2.0).*cos(q3)+LC.*ddq3.*sin(alphaAC-pi./2.0).*sin(q3)).*(x+aC.*sin(alphaAC)-eC.*sin(alphaAC)+LC.*cos(q3).*sin(alphaAC)))./lC+((-ddx+LC.*dq3.^2.*cos(q3).*cos(alphaAC-pi./2.0)+LC.*ddq3.*sin(q3).*cos(alphaAC-pi./2.0)).*(y+aC.*cos(alphaAC)-eC.*cos(alphaAC)+LC.*cos(alphaAC).*cos(q3)))./lC).*2.0)./lC-(((IlCyz.*((LC.*sin(q3).*cos(alphaAC-pi./2.0).*(y+aC.*cos(alphaAC)-eC.*cos(alphaAC)+LC.*cos(alphaAC).*cos(q3)))./lC+(LC.*sin(alphaAC-pi./2.0).*sin(q3).*(x+aC.*sin(alphaAC)-eC.*sin(alphaAC)+LC.*cos(q3).*sin(alphaAC)))./lC))./(lC.*2.0)+(IlCxy.*((LC.*sin(pi./2.0).*cos(q3).*(y+aC.*cos(alphaAC)-eC.*cos(alphaAC)+LC.*cos(alphaAC).*cos(q3)))./lC-(LC.*sin(alphaAC-pi./2.0).*sin(q3).*(z+LC.*sin(q3)))./lC))./(lC.*2.0)-(IlCyy.*((LC.*sin(q3).*cos(alphaAC-pi./2.0).*(z+LC.*sin(q3)))./lC+(LC.*sin(pi./2.0).*cos(q3).*(x+aC.*sin(alphaAC)-eC.*sin(alphaAC)+LC.*cos(q3).*sin(alphaAC)))./lC))./(lC.*2.0)).*(((ddz+LC.*ddq3.*sin(pi./2.0).*cos(q3)-LC.*dq3.^2.*sin(pi./2.0).*sin(q3)).*(x+aC.*sin(alphaAC)-eC.*sin(alphaAC)+LC.*cos(q3).*sin(alphaAC)))./lC-((dz+LC.*dq3.*cos(q3)).*(dx-LC.*dq3.*sin(q3).*cos(alphaAC-pi./2.0)))./lC+((dx-LC.*dq3.*sin(alphaAC).*sin(q3)).*(dz+LC.*dq3.*sin(pi./2.0).*cos(q3)))./lC+((z+LC.*sin(q3)).*(-ddx+LC.*dq3.^2.*cos(q3).*cos(alphaAC-pi./2.0)+LC.*ddq3.*sin(q3).*cos(alphaAC-pi./2.0)))./lC).*2.0)./lC+(LC.*g.*mLC.*cos(q3))./2.0+LC.*g.*mlC.*cos(q3)-(LC.*mlC.*sin(pi./2.0).*cos(q3).*(ddz./2.0-(LC.*ddq3.*sin(pi./2.0).*cos(q3))./2.0+(LC.*dq3.^2.*sin(pi./2.0).*sin(q3))./2.0))./2.0-LC.*mlC.*sin(pi./2.0).*cos(q3).*(ddz./4.0-(LC.*ddq3.*sin(pi./2.0).*cos(q3))./4.0+(LC.*dq3.^2.*sin(pi./2.0).*sin(q3))./4.0)+(LC.*mlC.*sin(q3).*cos(alphaAC-pi./2.0).*(ddx./2.0+(LC.*dq3.^2.*cos(q3).*cos(alphaAC-pi./2.0))./2.0+(LC.*ddq3.*sin(q3).*cos(alphaAC-pi./2.0))./2.0))./2.0+LC.*mlC.*sin(q3).*cos(alphaAC-pi./2.0).*(ddx./4.0+(LC.*dq3.^2.*cos(q3).*cos(alphaAC-pi./2.0))./4.0+(LC.*ddq3.*sin(q3).*cos(alphaAC-pi./2.0))./4.0)+(LC.*mlC.*sin(alphaAC-pi./2.0).*sin(q3).*(ddy.*(-1.0./2.0)+(LC.*dq3.^2.*sin(alphaAC-pi./2.0).*cos(q3))./2.0+(LC.*ddq3.*sin(alphaAC-pi./2.0).*sin(q3))./2.0))./2.0+LC.*mlC.*sin(alphaAC-pi./2.0).*sin(q3).*(ddy.*(-1.0./4.0)+(LC.*dq3.^2.*sin(alphaAC-pi./2.0).*cos(q3))./4.0+(LC.*ddq3.*sin(alphaAC-pi./2.0).*sin(q3))./4.0)];
dGammasdq = reshape([LA.*cos(q1).*(z+LA.*sin(q1)).*2.0-LA.*cos(alphaAA).*sin(q1).*(y+aA.*cos(alphaAA)-eA.*cos(alphaAA)+LA.*cos(alphaAA).*cos(q1)).*2.0-LA.*sin(alphaAA).*sin(q1).*(x+aA.*sin(alphaAA)-eA.*sin(alphaAA)+LA.*cos(q1).*sin(alphaAA)).*2.0,0.0,0.0,0.0,LB.*cos(q2).*(z+LB.*sin(q2)).*2.0-LB.*cos(alphaAB).*sin(q2).*(y+aB.*cos(alphaAB)-eB.*cos(alphaAB)+LB.*cos(alphaAB).*cos(q2)).*2.0-LB.*sin(alphaAB).*sin(q2).*(x+aB.*sin(alphaAB)-eB.*sin(alphaAB)+LB.*cos(q2).*sin(alphaAB)).*2.0,0.0,0.0,0.0,LC.*cos(q3).*(z+LC.*sin(q3)).*2.0-LC.*cos(alphaAC).*sin(q3).*(y+aC.*cos(alphaAC)-eC.*cos(alphaAC)+LC.*cos(alphaAC).*cos(q3)).*2.0-LC.*sin(alphaAC).*sin(q3).*(x+aC.*sin(alphaAC)-eC.*sin(alphaAC)+LC.*cos(q3).*sin(alphaAC)).*2.0],[3,3]);


lambda = dGammasdxyz\(Mxyz - J'*Fext);

lambdaA = lambda(1);
lambdaB = lambda(2);
lambdaC = lambda(3);

M = reshape([ILAxx.*sin(alphaAA-pi./2.0).^2+ILAyy.*cos(alphaAA-pi./2.0).^2+(((LA.*sin(pi./2.0).*cos(q1).*(y+aA.*cos(alphaAA)-eA.*cos(alphaAA)+LA.*cos(alphaAA).*cos(q1)))./lA-(LA.*sin(alphaAA-pi./2.0).*sin(q1).*(z+LA.*sin(q1)))./lA).*((IlAxz.*((LA.*sin(q1).*cos(alphaAA-pi./2.0).*(y+aA.*cos(alphaAA)-eA.*cos(alphaAA)+LA.*cos(alphaAA).*cos(q1)))./lA+(LA.*sin(alphaAA-pi./2.0).*sin(q1).*(x+aA.*sin(alphaAA)-eA.*sin(alphaAA)+LA.*cos(q1).*sin(alphaAA)))./lA))./(lA.*2.0)+(IlAxx.*((LA.*sin(pi./2.0).*cos(q1).*(y+aA.*cos(alphaAA)-eA.*cos(alphaAA)+LA.*cos(alphaAA).*cos(q1)))./lA-(LA.*sin(alphaAA-pi./2.0).*sin(q1).*(z+LA.*sin(q1)))./lA))./(lA.*2.0)-(IlAxy.*((LA.*sin(q1).*cos(alphaAA-pi./2.0).*(z+LA.*sin(q1)))./lA+(LA.*sin(pi./2.0).*cos(q1).*(x+aA.*sin(alphaAA)-eA.*sin(alphaAA)+LA.*cos(q1).*sin(alphaAA)))./lA))./(lA.*2.0)).*4.0)./lA-(((LA.*sin(q1).*cos(alphaAA-pi./2.0).*(z+LA.*sin(q1)))./lA+(LA.*sin(pi./2.0).*cos(q1).*(x+aA.*sin(alphaAA)-eA.*sin(alphaAA)+LA.*cos(q1).*sin(alphaAA)))./lA).*((IlAyz.*((LA.*sin(q1).*cos(alphaAA-pi./2.0).*(y+aA.*cos(alphaAA)-eA.*cos(alphaAA)+LA.*cos(alphaAA).*cos(q1)))./lA+(LA.*sin(alphaAA-pi./2.0).*sin(q1).*(x+aA.*sin(alphaAA)-eA.*sin(alphaAA)+LA.*cos(q1).*sin(alphaAA)))./lA))./(lA.*2.0)+(IlAxy.*((LA.*sin(pi./2.0).*cos(q1).*(y+aA.*cos(alphaAA)-eA.*cos(alphaAA)+LA.*cos(alphaAA).*cos(q1)))./lA-(LA.*sin(alphaAA-pi./2.0).*sin(q1).*(z+LA.*sin(q1)))./lA))./(lA.*2.0)-(IlAyy.*((LA.*sin(q1).*cos(alphaAA-pi./2.0).*(z+LA.*sin(q1)))./lA+(LA.*sin(pi./2.0).*cos(q1).*(x+aA.*sin(alphaAA)-eA.*sin(alphaAA)+LA.*cos(q1).*sin(alphaAA)))./lA))./(lA.*2.0)).*4.0)./lA+ILAxy.*sin(alphaAA-pi./2.0).*cos(alphaAA-pi./2.0).*2.0+(((LA.*sin(q1).*cos(alphaAA-pi./2.0).*(y+aA.*cos(alphaAA)-eA.*cos(alphaAA)+LA.*cos(alphaAA).*cos(q1)))./lA+(LA.*sin(alphaAA-pi./2.0).*sin(q1).*(x+aA.*sin(alphaAA)-eA.*sin(alphaAA)+LA.*cos(q1).*sin(alphaAA)))./lA).*((IlAzz.*((LA.*sin(q1).*cos(alphaAA-pi./2.0).*(y+aA.*cos(alphaAA)-eA.*cos(alphaAA)+LA.*cos(alphaAA).*cos(q1)))./lA+(LA.*sin(alphaAA-pi./2.0).*sin(q1).*(x+aA.*sin(alphaAA)-eA.*sin(alphaAA)+LA.*cos(q1).*sin(alphaAA)))./lA))./(lA.*2.0)+(IlAxz.*((LA.*sin(pi./2.0).*cos(q1).*(y+aA.*cos(alphaAA)-eA.*cos(alphaAA)+LA.*cos(alphaAA).*cos(q1)))./lA-(LA.*sin(alphaAA-pi./2.0).*sin(q1).*(z+LA.*sin(q1)))./lA))./(lA.*2.0)-(IlAyz.*((LA.*sin(q1).*cos(alphaAA-pi./2.0).*(z+LA.*sin(q1)))./lA+(LA.*sin(pi./2.0).*cos(q1).*(x+aA.*sin(alphaAA)-eA.*sin(alphaAA)+LA.*cos(q1).*sin(alphaAA)))./lA))./(lA.*2.0)).*4.0)./lA+(LA.^2.*mlA.*sin(q1).^2.*cos(alphaAA-pi./2.0).^2)./2.0+(LA.^2.*mlA.*sin(alphaAA-pi./2.0).^2.*sin(q1).^2)./2.0+(LA.^2.*mlA.*sin(pi./2.0).^2.*cos(q1).^2)./2.0,0.0,0.0,0.0,ILBxx.*sin(alphaAB-pi./2.0).^2+ILByy.*cos(alphaAB-pi./2.0).^2+(((LB.*sin(pi./2.0).*cos(q2).*(y+aB.*cos(alphaAB)-eB.*cos(alphaAB)+LB.*cos(alphaAB).*cos(q2)))./lB-(LB.*sin(alphaAB-pi./2.0).*sin(q2).*(z+LB.*sin(q2)))./lB).*((IlBxz.*((LB.*sin(q2).*cos(alphaAB-pi./2.0).*(y+aB.*cos(alphaAB)-eB.*cos(alphaAB)+LB.*cos(alphaAB).*cos(q2)))./lB+(LB.*sin(alphaAB-pi./2.0).*sin(q2).*(x+aB.*sin(alphaAB)-eB.*sin(alphaAB)+LB.*cos(q2).*sin(alphaAB)))./lB))./(lB.*2.0)+(IlBxx.*((LB.*sin(pi./2.0).*cos(q2).*(y+aB.*cos(alphaAB)-eB.*cos(alphaAB)+LB.*cos(alphaAB).*cos(q2)))./lB-(LB.*sin(alphaAB-pi./2.0).*sin(q2).*(z+LB.*sin(q2)))./lB))./(lB.*2.0)-(IlBxy.*((LB.*sin(q2).*cos(alphaAB-pi./2.0).*(z+LB.*sin(q2)))./lB+(LB.*sin(pi./2.0).*cos(q2).*(x+aB.*sin(alphaAB)-eB.*sin(alphaAB)+LB.*cos(q2).*sin(alphaAB)))./lB))./(lB.*2.0)).*4.0)./lB-(((LB.*sin(q2).*cos(alphaAB-pi./2.0).*(z+LB.*sin(q2)))./lB+(LB.*sin(pi./2.0).*cos(q2).*(x+aB.*sin(alphaAB)-eB.*sin(alphaAB)+LB.*cos(q2).*sin(alphaAB)))./lB).*((IlByz.*((LB.*sin(q2).*cos(alphaAB-pi./2.0).*(y+aB.*cos(alphaAB)-eB.*cos(alphaAB)+LB.*cos(alphaAB).*cos(q2)))./lB+(LB.*sin(alphaAB-pi./2.0).*sin(q2).*(x+aB.*sin(alphaAB)-eB.*sin(alphaAB)+LB.*cos(q2).*sin(alphaAB)))./lB))./(lB.*2.0)+(IlBxy.*((LB.*sin(pi./2.0).*cos(q2).*(y+aB.*cos(alphaAB)-eB.*cos(alphaAB)+LB.*cos(alphaAB).*cos(q2)))./lB-(LB.*sin(alphaAB-pi./2.0).*sin(q2).*(z+LB.*sin(q2)))./lB))./(lB.*2.0)-(IlByy.*((LB.*sin(q2).*cos(alphaAB-pi./2.0).*(z+LB.*sin(q2)))./lB+(LB.*sin(pi./2.0).*cos(q2).*(x+aB.*sin(alphaAB)-eB.*sin(alphaAB)+LB.*cos(q2).*sin(alphaAB)))./lB))./(lB.*2.0)).*4.0)./lB+ILBxy.*sin(alphaAB-pi./2.0).*cos(alphaAB-pi./2.0).*2.0+(((LB.*sin(q2).*cos(alphaAB-pi./2.0).*(y+aB.*cos(alphaAB)-eB.*cos(alphaAB)+LB.*cos(alphaAB).*cos(q2)))./lB+(LB.*sin(alphaAB-pi./2.0).*sin(q2).*(x+aB.*sin(alphaAB)-eB.*sin(alphaAB)+LB.*cos(q2).*sin(alphaAB)))./lB).*((IlBzz.*((LB.*sin(q2).*cos(alphaAB-pi./2.0).*(y+aB.*cos(alphaAB)-eB.*cos(alphaAB)+LB.*cos(alphaAB).*cos(q2)))./lB+(LB.*sin(alphaAB-pi./2.0).*sin(q2).*(x+aB.*sin(alphaAB)-eB.*sin(alphaAB)+LB.*cos(q2).*sin(alphaAB)))./lB))./(lB.*2.0)+(IlBxz.*((LB.*sin(pi./2.0).*cos(q2).*(y+aB.*cos(alphaAB)-eB.*cos(alphaAB)+LB.*cos(alphaAB).*cos(q2)))./lB-(LB.*sin(alphaAB-pi./2.0).*sin(q2).*(z+LB.*sin(q2)))./lB))./(lB.*2.0)-(IlByz.*((LB.*sin(q2).*cos(alphaAB-pi./2.0).*(z+LB.*sin(q2)))./lB+(LB.*sin(pi./2.0).*cos(q2).*(x+aB.*sin(alphaAB)-eB.*sin(alphaAB)+LB.*cos(q2).*sin(alphaAB)))./lB))./(lB.*2.0)).*4.0)./lB+(LB.^2.*mlB.*sin(q2).^2.*cos(alphaAB-pi./2.0).^2)./2.0+(LB.^2.*mlB.*sin(alphaAB-pi./2.0).^2.*sin(q2).^2)./2.0+(LB.^2.*mlB.*sin(pi./2.0).^2.*cos(q2).^2)./2.0,0.0,0.0,0.0,ILCxx.*sin(alphaAC-pi./2.0).^2+ILCyy.*cos(alphaAC-pi./2.0).^2+(((LC.*sin(pi./2.0).*cos(q3).*(y+aC.*cos(alphaAC)-eC.*cos(alphaAC)+LC.*cos(alphaAC).*cos(q3)))./lC-(LC.*sin(alphaAC-pi./2.0).*sin(q3).*(z+LC.*sin(q3)))./lC).*((IlCxz.*((LC.*sin(q3).*cos(alphaAC-pi./2.0).*(y+aC.*cos(alphaAC)-eC.*cos(alphaAC)+LC.*cos(alphaAC).*cos(q3)))./lC+(LC.*sin(alphaAC-pi./2.0).*sin(q3).*(x+aC.*sin(alphaAC)-eC.*sin(alphaAC)+LC.*cos(q3).*sin(alphaAC)))./lC))./(lC.*2.0)+(IlCxx.*((LC.*sin(pi./2.0).*cos(q3).*(y+aC.*cos(alphaAC)-eC.*cos(alphaAC)+LC.*cos(alphaAC).*cos(q3)))./lC-(LC.*sin(alphaAC-pi./2.0).*sin(q3).*(z+LC.*sin(q3)))./lC))./(lC.*2.0)-(IlCxy.*((LC.*sin(q3).*cos(alphaAC-pi./2.0).*(z+LC.*sin(q3)))./lC+(LC.*sin(pi./2.0).*cos(q3).*(x+aC.*sin(alphaAC)-eC.*sin(alphaAC)+LC.*cos(q3).*sin(alphaAC)))./lC))./(lC.*2.0)).*4.0)./lC-(((LC.*sin(q3).*cos(alphaAC-pi./2.0).*(z+LC.*sin(q3)))./lC+(LC.*sin(pi./2.0).*cos(q3).*(x+aC.*sin(alphaAC)-eC.*sin(alphaAC)+LC.*cos(q3).*sin(alphaAC)))./lC).*((IlCyz.*((LC.*sin(q3).*cos(alphaAC-pi./2.0).*(y+aC.*cos(alphaAC)-eC.*cos(alphaAC)+LC.*cos(alphaAC).*cos(q3)))./lC+(LC.*sin(alphaAC-pi./2.0).*sin(q3).*(x+aC.*sin(alphaAC)-eC.*sin(alphaAC)+LC.*cos(q3).*sin(alphaAC)))./lC))./(lC.*2.0)+(IlCxy.*((LC.*sin(pi./2.0).*cos(q3).*(y+aC.*cos(alphaAC)-eC.*cos(alphaAC)+LC.*cos(alphaAC).*cos(q3)))./lC-(LC.*sin(alphaAC-pi./2.0).*sin(q3).*(z+LC.*sin(q3)))./lC))./(lC.*2.0)-(IlCyy.*((LC.*sin(q3).*cos(alphaAC-pi./2.0).*(z+LC.*sin(q3)))./lC+(LC.*sin(pi./2.0).*cos(q3).*(x+aC.*sin(alphaAC)-eC.*sin(alphaAC)+LC.*cos(q3).*sin(alphaAC)))./lC))./(lC.*2.0)).*4.0)./lC+ILCxy.*sin(alphaAC-pi./2.0).*cos(alphaAC-pi./2.0).*2.0+(((LC.*sin(q3).*cos(alphaAC-pi./2.0).*(y+aC.*cos(alphaAC)-eC.*cos(alphaAC)+LC.*cos(alphaAC).*cos(q3)))./lC+(LC.*sin(alphaAC-pi./2.0).*sin(q3).*(x+aC.*sin(alphaAC)-eC.*sin(alphaAC)+LC.*cos(q3).*sin(alphaAC)))./lC).*((IlCzz.*((LC.*sin(q3).*cos(alphaAC-pi./2.0).*(y+aC.*cos(alphaAC)-eC.*cos(alphaAC)+LC.*cos(alphaAC).*cos(q3)))./lC+(LC.*sin(alphaAC-pi./2.0).*sin(q3).*(x+aC.*sin(alphaAC)-eC.*sin(alphaAC)+LC.*cos(q3).*sin(alphaAC)))./lC))./(lC.*2.0)+(IlCxz.*((LC.*sin(pi./2.0).*cos(q3).*(y+aC.*cos(alphaAC)-eC.*cos(alphaAC)+LC.*cos(alphaAC).*cos(q3)))./lC-(LC.*sin(alphaAC-pi./2.0).*sin(q3).*(z+LC.*sin(q3)))./lC))./(lC.*2.0)-(IlCyz.*((LC.*sin(q3).*cos(alphaAC-pi./2.0).*(z+LC.*sin(q3)))./lC+(LC.*sin(pi./2.0).*cos(q3).*(x+aC.*sin(alphaAC)-eC.*sin(alphaAC)+LC.*cos(q3).*sin(alphaAC)))./lC))./(lC.*2.0)).*4.0)./lC+(LC.^2.*mlC.*sin(q3).^2.*cos(alphaAC-pi./2.0).^2)./2.0+(LC.^2.*mlC.*sin(alphaAC-pi./2.0).^2.*sin(q3).^2)./2.0+(LC.^2.*mlC.*sin(pi./2.0).^2.*cos(q3).^2)./2.0],[3,3]);
f = [-lambdaA.*(LA.*cos(q1).*(z+LA.*sin(q1)).*-2.0+LA.*cos(alphaAA).*sin(q1).*(y+aA.*cos(alphaAA)-eA.*cos(alphaAA)+LA.*cos(alphaAA).*cos(q1)).*2.0+LA.*sin(alphaAA).*sin(q1).*(x+aA.*sin(alphaAA)-eA.*sin(alphaAA)+LA.*cos(q1).*sin(alphaAA)).*2.0)-((((dx-LA.*dq1.*sin(q1).*cos(alphaAA-pi./2.0)).*(y+aA.*cos(alphaAA)-eA.*cos(alphaAA)+LA.*cos(alphaAA).*cos(q1)))./lA-((dy+LA.*dq1.*sin(alphaAA-pi./2.0).*sin(q1)).*(x+aA.*sin(alphaAA)-eA.*sin(alphaAA)+LA.*cos(q1).*sin(alphaAA)))./lA).*((IlAxz.*((LA.*cos(q1).*(dy+LA.*dq1.*sin(alphaAA-pi./2.0).*sin(q1)))./lA+(LA.*cos(alphaAA).*sin(q1).*(dz+LA.*dq1.*sin(pi./2.0).*cos(q1)))./lA+(LA.*dq1.*sin(alphaAA-pi./2.0).*cos(q1).*(z+LA.*sin(q1)))./lA+(LA.*dq1.*sin(pi./2.0).*sin(q1).*(y+aA.*cos(alphaAA)-eA.*cos(alphaAA)+LA.*cos(alphaAA).*cos(q1)))./lA).*(-1.0./2.0))./lA+(IlAyz.*((LA.*cos(q1).*(dx-LA.*dq1.*sin(q1).*cos(alphaAA-pi./2.0)))./lA+(LA.*sin(alphaAA).*sin(q1).*(dz+LA.*dq1.*sin(pi./2.0).*cos(q1)))./lA-(LA.*dq1.*cos(q1).*cos(alphaAA-pi./2.0).*(z+LA.*sin(q1)))./lA+(LA.*dq1.*sin(pi./2.0).*sin(q1).*(x+aA.*sin(alphaAA)-eA.*sin(alphaAA)+LA.*cos(q1).*sin(alphaAA)))./lA))./(lA.*2.0)+(IlAzz.*((LA.*cos(alphaAA).*sin(q1).*(dx-LA.*dq1.*sin(q1).*cos(alphaAA-pi./2.0)))./lA-(LA.*sin(alphaAA).*sin(q1).*(dy+LA.*dq1.*sin(alphaAA-pi./2.0).*sin(q1)))./lA+(LA.*dq1.*sin(alphaAA-pi./2.0).*cos(q1).*(x+aA.*sin(alphaAA)-eA.*sin(alphaAA)+LA.*cos(q1).*sin(alphaAA)))./lA+(LA.*dq1.*cos(q1).*cos(alphaAA-pi./2.0).*(y+aA.*cos(alphaAA)-eA.*cos(alphaAA)+LA.*cos(alphaAA).*cos(q1)))./lA))./(lA.*2.0)).*2.0)./lA-((((dx-LA.*dq1.*sin(q1).*cos(alphaAA-pi./2.0)).*(y+aA.*cos(alphaAA)-eA.*cos(alphaAA)+LA.*cos(alphaAA).*cos(q1)))./lA-((dy+LA.*dq1.*sin(alphaAA-pi./2.0).*sin(q1)).*(x+aA.*sin(alphaAA)-eA.*sin(alphaAA)+LA.*cos(q1).*sin(alphaAA)))./lA).*((IlAxz.*((LA.*sin(alphaAA-pi./2.0).*sin(q1).*(dz+LA.*dq1.*cos(q1)))./lA-(LA.*sin(pi./2.0).*cos(q1).*(dy-LA.*dq1.*cos(alphaAA).*sin(q1)))./lA+(LA.*dq1.*sin(alphaAA-pi./2.0).*cos(q1).*(z+LA.*sin(q1)))./lA+(LA.*dq1.*sin(pi./2.0).*sin(q1).*(y+aA.*cos(alphaAA)-eA.*cos(alphaAA)+LA.*cos(alphaAA).*cos(q1)))./lA))./(lA.*2.0)+(IlAyz.*((LA.*sin(pi./2.0).*cos(q1).*(dx-LA.*dq1.*sin(alphaAA).*sin(q1)))./lA+(LA.*sin(q1).*cos(alphaAA-pi./2.0).*(dz+LA.*dq1.*cos(q1)))./lA+(LA.*dq1.*cos(q1).*cos(alphaAA-pi./2.0).*(z+LA.*sin(q1)))./lA-(LA.*dq1.*sin(pi./2.0).*sin(q1).*(x+aA.*sin(alphaAA)-eA.*sin(alphaAA)+LA.*cos(q1).*sin(alphaAA)))./lA))./(lA.*2.0)-(IlAzz.*((LA.*sin(q1).*cos(alphaAA-pi./2.0).*(dy-LA.*dq1.*cos(alphaAA).*sin(q1)))./lA+(LA.*sin(alphaAA-pi./2.0).*sin(q1).*(dx-LA.*dq1.*sin(alphaAA).*sin(q1)))./lA+(LA.*dq1.*sin(alphaAA-pi./2.0).*cos(q1).*(x+aA.*sin(alphaAA)-eA.*sin(alphaAA)+LA.*cos(q1).*sin(alphaAA)))./lA+(LA.*dq1.*cos(q1).*cos(alphaAA-pi./2.0).*(y+aA.*cos(alphaAA)-eA.*cos(alphaAA)+LA.*cos(alphaAA).*cos(q1)))./lA))./(lA.*2.0)).*2.0)./lA+(((IlAxz.*((LA.*sin(q1).*cos(alphaAA-pi./2.0).*(y+aA.*cos(alphaAA)-eA.*cos(alphaAA)+LA.*cos(alphaAA).*cos(q1)))./lA+(LA.*sin(alphaAA-pi./2.0).*sin(q1).*(x+aA.*sin(alphaAA)-eA.*sin(alphaAA)+LA.*cos(q1).*sin(alphaAA)))./lA))./(lA.*2.0)+(IlAxx.*((LA.*sin(pi./2.0).*cos(q1).*(y+aA.*cos(alphaAA)-eA.*cos(alphaAA)+LA.*cos(alphaAA).*cos(q1)))./lA-(LA.*sin(alphaAA-pi./2.0).*sin(q1).*(z+LA.*sin(q1)))./lA))./(lA.*2.0)-(IlAxy.*((LA.*sin(q1).*cos(alphaAA-pi./2.0).*(z+LA.*sin(q1)))./lA+(LA.*sin(pi./2.0).*cos(q1).*(x+aA.*sin(alphaAA)-eA.*sin(alphaAA)+LA.*cos(q1).*sin(alphaAA)))./lA))./(lA.*2.0)).*(((dz+LA.*dq1.*cos(q1)).*(dy+LA.*dq1.*sin(alphaAA-pi./2.0).*sin(q1)))./lA-((dy-LA.*dq1.*cos(alphaAA).*sin(q1)).*(dz+LA.*dq1.*sin(pi./2.0).*cos(q1)))./lA+((ddy+LA.*dq1.^2.*sin(alphaAA-pi./2.0).*cos(q1)).*(z+LA.*sin(q1)))./lA-((ddz-LA.*dq1.^2.*sin(pi./2.0).*sin(q1)).*(y+aA.*cos(alphaAA)-eA.*cos(alphaAA)+LA.*cos(alphaAA).*cos(q1)))./lA).*2.0)./lA-(((IlAxz.*(((dx-LA.*dq1.*sin(q1).*cos(alphaAA-pi./2.0)).*(y+aA.*cos(alphaAA)-eA.*cos(alphaAA)+LA.*cos(alphaAA).*cos(q1)))./lA-((dy+LA.*dq1.*sin(alphaAA-pi./2.0).*sin(q1)).*(x+aA.*sin(alphaAA)-eA.*sin(alphaAA)+LA.*cos(q1).*sin(alphaAA)))./lA).*(-1.0./2.0))./lA+(IlAxx.*(((dz+LA.*dq1.*sin(pi./2.0).*cos(q1)).*(y+aA.*cos(alphaAA)-eA.*cos(alphaAA)+LA.*cos(alphaAA).*cos(q1)))./lA-((z+LA.*sin(q1)).*(dy+LA.*dq1.*sin(alphaAA-pi./2.0).*sin(q1)))./lA))./(lA.*2.0)+(IlAxy.*(((z+LA.*sin(q1)).*(dx-LA.*dq1.*sin(q1).*cos(alphaAA-pi./2.0)))./lA-((dz+LA.*dq1.*sin(pi./2.0).*cos(q1)).*(x+aA.*sin(alphaAA)-eA.*sin(alphaAA)+LA.*cos(q1).*sin(alphaAA)))./lA))./(lA.*2.0)).*((LA.*cos(q1).*(dy+LA.*dq1.*sin(alphaAA-pi./2.0).*sin(q1)))./lA+(LA.*cos(alphaAA).*sin(q1).*(dz+LA.*dq1.*sin(pi./2.0).*cos(q1)))./lA+(LA.*dq1.*sin(alphaAA-pi./2.0).*cos(q1).*(z+LA.*sin(q1)))./lA+(LA.*dq1.*sin(pi./2.0).*sin(q1).*(y+aA.*cos(alphaAA)-eA.*cos(alphaAA)+LA.*cos(alphaAA).*cos(q1)))./lA).*2.0)./lA+(((IlAxz.*(((dx-LA.*dq1.*sin(q1).*cos(alphaAA-pi./2.0)).*(y+aA.*cos(alphaAA)-eA.*cos(alphaAA)+LA.*cos(alphaAA).*cos(q1)))./lA-((dy+LA.*dq1.*sin(alphaAA-pi./2.0).*sin(q1)).*(x+aA.*sin(alphaAA)-eA.*sin(alphaAA)+LA.*cos(q1).*sin(alphaAA)))./lA).*(-1.0./2.0))./lA+(IlAxx.*(((dz+LA.*dq1.*sin(pi./2.0).*cos(q1)).*(y+aA.*cos(alphaAA)-eA.*cos(alphaAA)+LA.*cos(alphaAA).*cos(q1)))./lA-((z+LA.*sin(q1)).*(dy+LA.*dq1.*sin(alphaAA-pi./2.0).*sin(q1)))./lA))./(lA.*2.0)+(IlAxy.*(((z+LA.*sin(q1)).*(dx-LA.*dq1.*sin(q1).*cos(alphaAA-pi./2.0)))./lA-((dz+LA.*dq1.*sin(pi./2.0).*cos(q1)).*(x+aA.*sin(alphaAA)-eA.*sin(alphaAA)+LA.*cos(q1).*sin(alphaAA)))./lA))./(lA.*2.0)).*((LA.*sin(alphaAA-pi./2.0).*sin(q1).*(dz+LA.*dq1.*cos(q1)))./lA-(LA.*sin(pi./2.0).*cos(q1).*(dy-LA.*dq1.*cos(alphaAA).*sin(q1)))./lA+(LA.*dq1.*sin(alphaAA-pi./2.0).*cos(q1).*(z+LA.*sin(q1)))./lA+(LA.*dq1.*sin(pi./2.0).*sin(q1).*(y+aA.*cos(alphaAA)-eA.*cos(alphaAA)+LA.*cos(alphaAA).*cos(q1)))./lA).*2.0)./lA+(((LA.*sin(q1).*cos(alphaAA-pi./2.0).*(y+aA.*cos(alphaAA)-eA.*cos(alphaAA)+LA.*cos(alphaAA).*cos(q1)))./lA+(LA.*sin(alphaAA-pi./2.0).*sin(q1).*(x+aA.*sin(alphaAA)-eA.*sin(alphaAA)+LA.*cos(q1).*sin(alphaAA)))./lA).*((IlAxz.*(((dz+LA.*dq1.*cos(q1)).*(dy+LA.*dq1.*sin(alphaAA-pi./2.0).*sin(q1)))./lA-((dy-LA.*dq1.*cos(alphaAA).*sin(q1)).*(dz+LA.*dq1.*sin(pi./2.0).*cos(q1)))./lA+((ddy+LA.*dq1.^2.*sin(alphaAA-pi./2.0).*cos(q1)).*(z+LA.*sin(q1)))./lA-((ddz-LA.*dq1.^2.*sin(pi./2.0).*sin(q1)).*(y+aA.*cos(alphaAA)-eA.*cos(alphaAA)+LA.*cos(alphaAA).*cos(q1)))./lA))./(lA.*2.0)-(IlAyz.*(((dz+LA.*dq1.*cos(q1)).*(dx-LA.*dq1.*sin(q1).*cos(alphaAA-pi./2.0)))./lA+((z+LA.*sin(q1)).*(ddx-LA.*dq1.^2.*cos(q1).*cos(alphaAA-pi./2.0)))./lA-((dx-LA.*dq1.*sin(alphaAA).*sin(q1)).*(dz+LA.*dq1.*sin(pi./2.0).*cos(q1)))./lA-((ddz-LA.*dq1.^2.*sin(pi./2.0).*sin(q1)).*(x+aA.*sin(alphaAA)-eA.*sin(alphaAA)+LA.*cos(q1).*sin(alphaAA)))./lA))./(lA.*2.0)+(IlAzz.*(((ddx-LA.*dq1.^2.*cos(q1).*cos(alphaAA-pi./2.0)).*(y+aA.*cos(alphaAA)-eA.*cos(alphaAA)+LA.*cos(alphaAA).*cos(q1)))./lA+((dy-LA.*dq1.*cos(alphaAA).*sin(q1)).*(dx-LA.*dq1.*sin(q1).*cos(alphaAA-pi./2.0)))./lA-((dx-LA.*dq1.*sin(alphaAA).*sin(q1)).*(dy+LA.*dq1.*sin(alphaAA-pi./2.0).*sin(q1)))./lA-((ddy+LA.*dq1.^2.*sin(alphaAA-pi./2.0).*cos(q1)).*(x+aA.*sin(alphaAA)-eA.*sin(alphaAA)+LA.*cos(q1).*sin(alphaAA)))./lA))./(lA.*2.0)).*2.0)./lA-(((IlAyz.*((LA.*sin(q1).*cos(alphaAA-pi./2.0).*(y+aA.*cos(alphaAA)-eA.*cos(alphaAA)+LA.*cos(alphaAA).*cos(q1)))./lA+(LA.*sin(alphaAA-pi./2.0).*sin(q1).*(x+aA.*sin(alphaAA)-eA.*sin(alphaAA)+LA.*cos(q1).*sin(alphaAA)))./lA))./(lA.*2.0)+(IlAxy.*((LA.*sin(pi./2.0).*cos(q1).*(y+aA.*cos(alphaAA)-eA.*cos(alphaAA)+LA.*cos(alphaAA).*cos(q1)))./lA-(LA.*sin(alphaAA-pi./2.0).*sin(q1).*(z+LA.*sin(q1)))./lA))./(lA.*2.0)-(IlAyy.*((LA.*sin(q1).*cos(alphaAA-pi./2.0).*(z+LA.*sin(q1)))./lA+(LA.*sin(pi./2.0).*cos(q1).*(x+aA.*sin(alphaAA)-eA.*sin(alphaAA)+LA.*cos(q1).*sin(alphaAA)))./lA))./(lA.*2.0)).*(((dz+LA.*dq1.*cos(q1)).*(dx-LA.*dq1.*sin(q1).*cos(alphaAA-pi./2.0)))./lA+((z+LA.*sin(q1)).*(ddx-LA.*dq1.^2.*cos(q1).*cos(alphaAA-pi./2.0)))./lA-((dx-LA.*dq1.*sin(alphaAA).*sin(q1)).*(dz+LA.*dq1.*sin(pi./2.0).*cos(q1)))./lA-((ddz-LA.*dq1.^2.*sin(pi./2.0).*sin(q1)).*(x+aA.*sin(alphaAA)-eA.*sin(alphaAA)+LA.*cos(q1).*sin(alphaAA)))./lA).*2.0)./lA+(((IlAzz.*((LA.*sin(q1).*cos(alphaAA-pi./2.0).*(y+aA.*cos(alphaAA)-eA.*cos(alphaAA)+LA.*cos(alphaAA).*cos(q1)))./lA+(LA.*sin(alphaAA-pi./2.0).*sin(q1).*(x+aA.*sin(alphaAA)-eA.*sin(alphaAA)+LA.*cos(q1).*sin(alphaAA)))./lA))./(lA.*2.0)+(IlAxz.*((LA.*sin(pi./2.0).*cos(q1).*(y+aA.*cos(alphaAA)-eA.*cos(alphaAA)+LA.*cos(alphaAA).*cos(q1)))./lA-(LA.*sin(alphaAA-pi./2.0).*sin(q1).*(z+LA.*sin(q1)))./lA))./(lA.*2.0)-(IlAyz.*((LA.*sin(q1).*cos(alphaAA-pi./2.0).*(z+LA.*sin(q1)))./lA+(LA.*sin(pi./2.0).*cos(q1).*(x+aA.*sin(alphaAA)-eA.*sin(alphaAA)+LA.*cos(q1).*sin(alphaAA)))./lA))./(lA.*2.0)).*(((ddx-LA.*dq1.^2.*cos(q1).*cos(alphaAA-pi./2.0)).*(y+aA.*cos(alphaAA)-eA.*cos(alphaAA)+LA.*cos(alphaAA).*cos(q1)))./lA+((dy-LA.*dq1.*cos(alphaAA).*sin(q1)).*(dx-LA.*dq1.*sin(q1).*cos(alphaAA-pi./2.0)))./lA-((dx-LA.*dq1.*sin(alphaAA).*sin(q1)).*(dy+LA.*dq1.*sin(alphaAA-pi./2.0).*sin(q1)))./lA-((ddy+LA.*dq1.^2.*sin(alphaAA-pi./2.0).*cos(q1)).*(x+aA.*sin(alphaAA)-eA.*sin(alphaAA)+LA.*cos(q1).*sin(alphaAA)))./lA).*2.0)./lA+(((IlAyz.*(((dx-LA.*dq1.*sin(q1).*cos(alphaAA-pi./2.0)).*(y+aA.*cos(alphaAA)-eA.*cos(alphaAA)+LA.*cos(alphaAA).*cos(q1)))./lA-((dy+LA.*dq1.*sin(alphaAA-pi./2.0).*sin(q1)).*(x+aA.*sin(alphaAA)-eA.*sin(alphaAA)+LA.*cos(q1).*sin(alphaAA)))./lA).*(-1.0./2.0))./lA+(IlAxy.*(((dz+LA.*dq1.*sin(pi./2.0).*cos(q1)).*(y+aA.*cos(alphaAA)-eA.*cos(alphaAA)+LA.*cos(alphaAA).*cos(q1)))./lA-((z+LA.*sin(q1)).*(dy+LA.*dq1.*sin(alphaAA-pi./2.0).*sin(q1)))./lA))./(lA.*2.0)+(IlAyy.*(((z+LA.*sin(q1)).*(dx-LA.*dq1.*sin(q1).*cos(alphaAA-pi./2.0)))./lA-((dz+LA.*dq1.*sin(pi./2.0).*cos(q1)).*(x+aA.*sin(alphaAA)-eA.*sin(alphaAA)+LA.*cos(q1).*sin(alphaAA)))./lA))./(lA.*2.0)).*((LA.*cos(q1).*(dx-LA.*dq1.*sin(q1).*cos(alphaAA-pi./2.0)))./lA+(LA.*sin(alphaAA).*sin(q1).*(dz+LA.*dq1.*sin(pi./2.0).*cos(q1)))./lA-(LA.*dq1.*cos(q1).*cos(alphaAA-pi./2.0).*(z+LA.*sin(q1)))./lA+(LA.*dq1.*sin(pi./2.0).*sin(q1).*(x+aA.*sin(alphaAA)-eA.*sin(alphaAA)+LA.*cos(q1).*sin(alphaAA)))./lA).*2.0)./lA+(((IlAyz.*(((dx-LA.*dq1.*sin(q1).*cos(alphaAA-pi./2.0)).*(y+aA.*cos(alphaAA)-eA.*cos(alphaAA)+LA.*cos(alphaAA).*cos(q1)))./lA-((dy+LA.*dq1.*sin(alphaAA-pi./2.0).*sin(q1)).*(x+aA.*sin(alphaAA)-eA.*sin(alphaAA)+LA.*cos(q1).*sin(alphaAA)))./lA).*(-1.0./2.0))./lA+(IlAxy.*(((dz+LA.*dq1.*sin(pi./2.0).*cos(q1)).*(y+aA.*cos(alphaAA)-eA.*cos(alphaAA)+LA.*cos(alphaAA).*cos(q1)))./lA-((z+LA.*sin(q1)).*(dy+LA.*dq1.*sin(alphaAA-pi./2.0).*sin(q1)))./lA))./(lA.*2.0)+(IlAyy.*(((z+LA.*sin(q1)).*(dx-LA.*dq1.*sin(q1).*cos(alphaAA-pi./2.0)))./lA-((dz+LA.*dq1.*sin(pi./2.0).*cos(q1)).*(x+aA.*sin(alphaAA)-eA.*sin(alphaAA)+LA.*cos(q1).*sin(alphaAA)))./lA))./(lA.*2.0)).*((LA.*sin(pi./2.0).*cos(q1).*(dx-LA.*dq1.*sin(alphaAA).*sin(q1)))./lA+(LA.*sin(q1).*cos(alphaAA-pi./2.0).*(dz+LA.*dq1.*cos(q1)))./lA+(LA.*dq1.*cos(q1).*cos(alphaAA-pi./2.0).*(z+LA.*sin(q1)))./lA-(LA.*dq1.*sin(pi./2.0).*sin(q1).*(x+aA.*sin(alphaAA)-eA.*sin(alphaAA)+LA.*cos(q1).*sin(alphaAA)))./lA).*2.0)./lA+((((dz+LA.*dq1.*sin(pi./2.0).*cos(q1)).*(y+aA.*cos(alphaAA)-eA.*cos(alphaAA)+LA.*cos(alphaAA).*cos(q1)))./lA-((z+LA.*sin(q1)).*(dy+LA.*dq1.*sin(alphaAA-pi./2.0).*sin(q1)))./lA).*((IlAxx.*((LA.*cos(q1).*(dy+LA.*dq1.*sin(alphaAA-pi./2.0).*sin(q1)))./lA+(LA.*cos(alphaAA).*sin(q1).*(dz+LA.*dq1.*sin(pi./2.0).*cos(q1)))./lA+(LA.*dq1.*sin(alphaAA-pi./2.0).*cos(q1).*(z+LA.*sin(q1)))./lA+(LA.*dq1.*sin(pi./2.0).*sin(q1).*(y+aA.*cos(alphaAA)-eA.*cos(alphaAA)+LA.*cos(alphaAA).*cos(q1)))./lA).*(-1.0./2.0))./lA+(IlAxy.*((LA.*cos(q1).*(dx-LA.*dq1.*sin(q1).*cos(alphaAA-pi./2.0)))./lA+(LA.*sin(alphaAA).*sin(q1).*(dz+LA.*dq1.*sin(pi./2.0).*cos(q1)))./lA-(LA.*dq1.*cos(q1).*cos(alphaAA-pi./2.0).*(z+LA.*sin(q1)))./lA+(LA.*dq1.*sin(pi./2.0).*sin(q1).*(x+aA.*sin(alphaAA)-eA.*sin(alphaAA)+LA.*cos(q1).*sin(alphaAA)))./lA))./(lA.*2.0)+(IlAxz.*((LA.*cos(alphaAA).*sin(q1).*(dx-LA.*dq1.*sin(q1).*cos(alphaAA-pi./2.0)))./lA-(LA.*sin(alphaAA).*sin(q1).*(dy+LA.*dq1.*sin(alphaAA-pi./2.0).*sin(q1)))./lA+(LA.*dq1.*sin(alphaAA-pi./2.0).*cos(q1).*(x+aA.*sin(alphaAA)-eA.*sin(alphaAA)+LA.*cos(q1).*sin(alphaAA)))./lA+(LA.*dq1.*cos(q1).*cos(alphaAA-pi./2.0).*(y+aA.*cos(alphaAA)-eA.*cos(alphaAA)+LA.*cos(alphaAA).*cos(q1)))./lA))./(lA.*2.0)).*2.0)./lA+((((dz+LA.*dq1.*sin(pi./2.0).*cos(q1)).*(y+aA.*cos(alphaAA)-eA.*cos(alphaAA)+LA.*cos(alphaAA).*cos(q1)))./lA-((z+LA.*sin(q1)).*(dy+LA.*dq1.*sin(alphaAA-pi./2.0).*sin(q1)))./lA).*((IlAxx.*((LA.*sin(alphaAA-pi./2.0).*sin(q1).*(dz+LA.*dq1.*cos(q1)))./lA-(LA.*sin(pi./2.0).*cos(q1).*(dy-LA.*dq1.*cos(alphaAA).*sin(q1)))./lA+(LA.*dq1.*sin(alphaAA-pi./2.0).*cos(q1).*(z+LA.*sin(q1)))./lA+(LA.*dq1.*sin(pi./2.0).*sin(q1).*(y+aA.*cos(alphaAA)-eA.*cos(alphaAA)+LA.*cos(alphaAA).*cos(q1)))./lA))./(lA.*2.0)+(IlAxy.*((LA.*sin(pi./2.0).*cos(q1).*(dx-LA.*dq1.*sin(alphaAA).*sin(q1)))./lA+(LA.*sin(q1).*cos(alphaAA-pi./2.0).*(dz+LA.*dq1.*cos(q1)))./lA+(LA.*dq1.*cos(q1).*cos(alphaAA-pi./2.0).*(z+LA.*sin(q1)))./lA-(LA.*dq1.*sin(pi./2.0).*sin(q1).*(x+aA.*sin(alphaAA)-eA.*sin(alphaAA)+LA.*cos(q1).*sin(alphaAA)))./lA))./(lA.*2.0)-(IlAxz.*((LA.*sin(q1).*cos(alphaAA-pi./2.0).*(dy-LA.*dq1.*cos(alphaAA).*sin(q1)))./lA+(LA.*sin(alphaAA-pi./2.0).*sin(q1).*(dx-LA.*dq1.*sin(alphaAA).*sin(q1)))./lA+(LA.*dq1.*sin(alphaAA-pi./2.0).*cos(q1).*(x+aA.*sin(alphaAA)-eA.*sin(alphaAA)+LA.*cos(q1).*sin(alphaAA)))./lA+(LA.*dq1.*cos(q1).*cos(alphaAA-pi./2.0).*(y+aA.*cos(alphaAA)-eA.*cos(alphaAA)+LA.*cos(alphaAA).*cos(q1)))./lA))./(lA.*2.0)).*2.0)./lA+(((IlAzz.*(((dx-LA.*dq1.*sin(q1).*cos(alphaAA-pi./2.0)).*(y+aA.*cos(alphaAA)-eA.*cos(alphaAA)+LA.*cos(alphaAA).*cos(q1)))./lA-((dy+LA.*dq1.*sin(alphaAA-pi./2.0).*sin(q1)).*(x+aA.*sin(alphaAA)-eA.*sin(alphaAA)+LA.*cos(q1).*sin(alphaAA)))./lA).*(-1.0./2.0))./lA+(IlAxz.*(((dz+LA.*dq1.*sin(pi./2.0).*cos(q1)).*(y+aA.*cos(alphaAA)-eA.*cos(alphaAA)+LA.*cos(alphaAA).*cos(q1)))./lA-((z+LA.*sin(q1)).*(dy+LA.*dq1.*sin(alphaAA-pi./2.0).*sin(q1)))./lA))./(lA.*2.0)+(IlAyz.*(((z+LA.*sin(q1)).*(dx-LA.*dq1.*sin(q1).*cos(alphaAA-pi./2.0)))./lA-((dz+LA.*dq1.*sin(pi./2.0).*cos(q1)).*(x+aA.*sin(alphaAA)-eA.*sin(alphaAA)+LA.*cos(q1).*sin(alphaAA)))./lA))./(lA.*2.0)).*((LA.*cos(alphaAA).*sin(q1).*(dx-LA.*dq1.*sin(q1).*cos(alphaAA-pi./2.0)))./lA-(LA.*sin(alphaAA).*sin(q1).*(dy+LA.*dq1.*sin(alphaAA-pi./2.0).*sin(q1)))./lA+(LA.*dq1.*sin(alphaAA-pi./2.0).*cos(q1).*(x+aA.*sin(alphaAA)-eA.*sin(alphaAA)+LA.*cos(q1).*sin(alphaAA)))./lA+(LA.*dq1.*cos(q1).*cos(alphaAA-pi./2.0).*(y+aA.*cos(alphaAA)-eA.*cos(alphaAA)+LA.*cos(alphaAA).*cos(q1)))./lA).*2.0)./lA-(((IlAzz.*(((dx-LA.*dq1.*sin(q1).*cos(alphaAA-pi./2.0)).*(y+aA.*cos(alphaAA)-eA.*cos(alphaAA)+LA.*cos(alphaAA).*cos(q1)))./lA-((dy+LA.*dq1.*sin(alphaAA-pi./2.0).*sin(q1)).*(x+aA.*sin(alphaAA)-eA.*sin(alphaAA)+LA.*cos(q1).*sin(alphaAA)))./lA).*(-1.0./2.0))./lA+(IlAxz.*(((dz+LA.*dq1.*sin(pi./2.0).*cos(q1)).*(y+aA.*cos(alphaAA)-eA.*cos(alphaAA)+LA.*cos(alphaAA).*cos(q1)))./lA-((z+LA.*sin(q1)).*(dy+LA.*dq1.*sin(alphaAA-pi./2.0).*sin(q1)))./lA))./(lA.*2.0)+(IlAyz.*(((z+LA.*sin(q1)).*(dx-LA.*dq1.*sin(q1).*cos(alphaAA-pi./2.0)))./lA-((dz+LA.*dq1.*sin(pi./2.0).*cos(q1)).*(x+aA.*sin(alphaAA)-eA.*sin(alphaAA)+LA.*cos(q1).*sin(alphaAA)))./lA))./(lA.*2.0)).*((LA.*sin(q1).*cos(alphaAA-pi./2.0).*(dy-LA.*dq1.*cos(alphaAA).*sin(q1)))./lA+(LA.*sin(alphaAA-pi./2.0).*sin(q1).*(dx-LA.*dq1.*sin(alphaAA).*sin(q1)))./lA+(LA.*dq1.*sin(alphaAA-pi./2.0).*cos(q1).*(x+aA.*sin(alphaAA)-eA.*sin(alphaAA)+LA.*cos(q1).*sin(alphaAA)))./lA+(LA.*dq1.*cos(q1).*cos(alphaAA-pi./2.0).*(y+aA.*cos(alphaAA)-eA.*cos(alphaAA)+LA.*cos(alphaAA).*cos(q1)))./lA).*2.0)./lA+((((z+LA.*sin(q1)).*(dx-LA.*dq1.*sin(q1).*cos(alphaAA-pi./2.0)))./lA-((dz+LA.*dq1.*sin(pi./2.0).*cos(q1)).*(x+aA.*sin(alphaAA)-eA.*sin(alphaAA)+LA.*cos(q1).*sin(alphaAA)))./lA).*((IlAxy.*((LA.*cos(q1).*(dy+LA.*dq1.*sin(alphaAA-pi./2.0).*sin(q1)))./lA+(LA.*cos(alphaAA).*sin(q1).*(dz+LA.*dq1.*sin(pi./2.0).*cos(q1)))./lA+(LA.*dq1.*sin(alphaAA-pi./2.0).*cos(q1).*(z+LA.*sin(q1)))./lA+(LA.*dq1.*sin(pi./2.0).*sin(q1).*(y+aA.*cos(alphaAA)-eA.*cos(alphaAA)+LA.*cos(alphaAA).*cos(q1)))./lA).*(-1.0./2.0))./lA+(IlAyy.*((LA.*cos(q1).*(dx-LA.*dq1.*sin(q1).*cos(alphaAA-pi./2.0)))./lA+(LA.*sin(alphaAA).*sin(q1).*(dz+LA.*dq1.*sin(pi./2.0).*cos(q1)))./lA-(LA.*dq1.*cos(q1).*cos(alphaAA-pi./2.0).*(z+LA.*sin(q1)))./lA+(LA.*dq1.*sin(pi./2.0).*sin(q1).*(x+aA.*sin(alphaAA)-eA.*sin(alphaAA)+LA.*cos(q1).*sin(alphaAA)))./lA))./(lA.*2.0)+(IlAyz.*((LA.*cos(alphaAA).*sin(q1).*(dx-LA.*dq1.*sin(q1).*cos(alphaAA-pi./2.0)))./lA-(LA.*sin(alphaAA).*sin(q1).*(dy+LA.*dq1.*sin(alphaAA-pi./2.0).*sin(q1)))./lA+(LA.*dq1.*sin(alphaAA-pi./2.0).*cos(q1).*(x+aA.*sin(alphaAA)-eA.*sin(alphaAA)+LA.*cos(q1).*sin(alphaAA)))./lA+(LA.*dq1.*cos(q1).*cos(alphaAA-pi./2.0).*(y+aA.*cos(alphaAA)-eA.*cos(alphaAA)+LA.*cos(alphaAA).*cos(q1)))./lA))./(lA.*2.0)).*2.0)./lA+((((z+LA.*sin(q1)).*(dx-LA.*dq1.*sin(q1).*cos(alphaAA-pi./2.0)))./lA-((dz+LA.*dq1.*sin(pi./2.0).*cos(q1)).*(x+aA.*sin(alphaAA)-eA.*sin(alphaAA)+LA.*cos(q1).*sin(alphaAA)))./lA).*((IlAxy.*((LA.*sin(alphaAA-pi./2.0).*sin(q1).*(dz+LA.*dq1.*cos(q1)))./lA-(LA.*sin(pi./2.0).*cos(q1).*(dy-LA.*dq1.*cos(alphaAA).*sin(q1)))./lA+(LA.*dq1.*sin(alphaAA-pi./2.0).*cos(q1).*(z+LA.*sin(q1)))./lA+(LA.*dq1.*sin(pi./2.0).*sin(q1).*(y+aA.*cos(alphaAA)-eA.*cos(alphaAA)+LA.*cos(alphaAA).*cos(q1)))./lA))./(lA.*2.0)+(IlAyy.*((LA.*sin(pi./2.0).*cos(q1).*(dx-LA.*dq1.*sin(alphaAA).*sin(q1)))./lA+(LA.*sin(q1).*cos(alphaAA-pi./2.0).*(dz+LA.*dq1.*cos(q1)))./lA+(LA.*dq1.*cos(q1).*cos(alphaAA-pi./2.0).*(z+LA.*sin(q1)))./lA-(LA.*dq1.*sin(pi./2.0).*sin(q1).*(x+aA.*sin(alphaAA)-eA.*sin(alphaAA)+LA.*cos(q1).*sin(alphaAA)))./lA))./(lA.*2.0)-(IlAyz.*((LA.*sin(q1).*cos(alphaAA-pi./2.0).*(dy-LA.*dq1.*cos(alphaAA).*sin(q1)))./lA+(LA.*sin(alphaAA-pi./2.0).*sin(q1).*(dx-LA.*dq1.*sin(alphaAA).*sin(q1)))./lA+(LA.*dq1.*sin(alphaAA-pi./2.0).*cos(q1).*(x+aA.*sin(alphaAA)-eA.*sin(alphaAA)+LA.*cos(q1).*sin(alphaAA)))./lA+(LA.*dq1.*cos(q1).*cos(alphaAA-pi./2.0).*(y+aA.*cos(alphaAA)-eA.*cos(alphaAA)+LA.*cos(alphaAA).*cos(q1)))./lA))./(lA.*2.0)).*2.0)./lA+(((LA.*sin(pi./2.0).*cos(q1).*(y+aA.*cos(alphaAA)-eA.*cos(alphaAA)+LA.*cos(alphaAA).*cos(q1)))./lA-(LA.*sin(alphaAA-pi./2.0).*sin(q1).*(z+LA.*sin(q1)))./lA).*((IlAxx.*(((dz+LA.*dq1.*cos(q1)).*(dy+LA.*dq1.*sin(alphaAA-pi./2.0).*sin(q1)))./lA-((dy-LA.*dq1.*cos(alphaAA).*sin(q1)).*(dz+LA.*dq1.*sin(pi./2.0).*cos(q1)))./lA+((ddy+LA.*dq1.^2.*sin(alphaAA-pi./2.0).*cos(q1)).*(z+LA.*sin(q1)))./lA-((ddz-LA.*dq1.^2.*sin(pi./2.0).*sin(q1)).*(y+aA.*cos(alphaAA)-eA.*cos(alphaAA)+LA.*cos(alphaAA).*cos(q1)))./lA))./(lA.*2.0)-(IlAxy.*(((dz+LA.*dq1.*cos(q1)).*(dx-LA.*dq1.*sin(q1).*cos(alphaAA-pi./2.0)))./lA+((z+LA.*sin(q1)).*(ddx-LA.*dq1.^2.*cos(q1).*cos(alphaAA-pi./2.0)))./lA-((dx-LA.*dq1.*sin(alphaAA).*sin(q1)).*(dz+LA.*dq1.*sin(pi./2.0).*cos(q1)))./lA-((ddz-LA.*dq1.^2.*sin(pi./2.0).*sin(q1)).*(x+aA.*sin(alphaAA)-eA.*sin(alphaAA)+LA.*cos(q1).*sin(alphaAA)))./lA))./(lA.*2.0)+(IlAxz.*(((ddx-LA.*dq1.^2.*cos(q1).*cos(alphaAA-pi./2.0)).*(y+aA.*cos(alphaAA)-eA.*cos(alphaAA)+LA.*cos(alphaAA).*cos(q1)))./lA+((dy-LA.*dq1.*cos(alphaAA).*sin(q1)).*(dx-LA.*dq1.*sin(q1).*cos(alphaAA-pi./2.0)))./lA-((dx-LA.*dq1.*sin(alphaAA).*sin(q1)).*(dy+LA.*dq1.*sin(alphaAA-pi./2.0).*sin(q1)))./lA-((ddy+LA.*dq1.^2.*sin(alphaAA-pi./2.0).*cos(q1)).*(x+aA.*sin(alphaAA)-eA.*sin(alphaAA)+LA.*cos(q1).*sin(alphaAA)))./lA))./(lA.*2.0)).*2.0)./lA-(((LA.*sin(q1).*cos(alphaAA-pi./2.0).*(z+LA.*sin(q1)))./lA+(LA.*sin(pi./2.0).*cos(q1).*(x+aA.*sin(alphaAA)-eA.*sin(alphaAA)+LA.*cos(q1).*sin(alphaAA)))./lA).*((IlAxy.*(((dz+LA.*dq1.*cos(q1)).*(dy+LA.*dq1.*sin(alphaAA-pi./2.0).*sin(q1)))./lA-((dy-LA.*dq1.*cos(alphaAA).*sin(q1)).*(dz+LA.*dq1.*sin(pi./2.0).*cos(q1)))./lA+((ddy+LA.*dq1.^2.*sin(alphaAA-pi./2.0).*cos(q1)).*(z+LA.*sin(q1)))./lA-((ddz-LA.*dq1.^2.*sin(pi./2.0).*sin(q1)).*(y+aA.*cos(alphaAA)-eA.*cos(alphaAA)+LA.*cos(alphaAA).*cos(q1)))./lA))./(lA.*2.0)-(IlAyy.*(((dz+LA.*dq1.*cos(q1)).*(dx-LA.*dq1.*sin(q1).*cos(alphaAA-pi./2.0)))./lA+((z+LA.*sin(q1)).*(ddx-LA.*dq1.^2.*cos(q1).*cos(alphaAA-pi./2.0)))./lA-((dx-LA.*dq1.*sin(alphaAA).*sin(q1)).*(dz+LA.*dq1.*sin(pi./2.0).*cos(q1)))./lA-((ddz-LA.*dq1.^2.*sin(pi./2.0).*sin(q1)).*(x+aA.*sin(alphaAA)-eA.*sin(alphaAA)+LA.*cos(q1).*sin(alphaAA)))./lA))./(lA.*2.0)+(IlAyz.*(((ddx-LA.*dq1.^2.*cos(q1).*cos(alphaAA-pi./2.0)).*(y+aA.*cos(alphaAA)-eA.*cos(alphaAA)+LA.*cos(alphaAA).*cos(q1)))./lA+((dy-LA.*dq1.*cos(alphaAA).*sin(q1)).*(dx-LA.*dq1.*sin(q1).*cos(alphaAA-pi./2.0)))./lA-((dx-LA.*dq1.*sin(alphaAA).*sin(q1)).*(dy+LA.*dq1.*sin(alphaAA-pi./2.0).*sin(q1)))./lA-((ddy+LA.*dq1.^2.*sin(alphaAA-pi./2.0).*cos(q1)).*(x+aA.*sin(alphaAA)-eA.*sin(alphaAA)+LA.*cos(q1).*sin(alphaAA)))./lA))./(lA.*2.0)).*2.0)./lA-(LA.*g.*mLA.*cos(q1))./2.0-LA.*g.*mlA.*cos(q1)-(LA.*mlA.*sin(q1).*cos(alphaAA-pi./2.0).*(ddx./2.0+(LA.*dq1.^2.*cos(q1).*cos(alphaAA-pi./2.0))./2.0))./2.0-LA.*mlA.*sin(q1).*cos(alphaAA-pi./2.0).*(ddx./4.0+(LA.*dq1.^2.*cos(q1).*cos(alphaAA-pi./2.0))./4.0)+(LA.*mlA.*sin(alphaAA-pi./2.0).*sin(q1).*(ddy./2.0-(LA.*dq1.^2.*sin(alphaAA-pi./2.0).*cos(q1))./2.0))./2.0+LA.*mlA.*sin(alphaAA-pi./2.0).*sin(q1).*(ddy./4.0-(LA.*dq1.^2.*sin(alphaAA-pi./2.0).*cos(q1))./4.0)+(LA.*mlA.*sin(pi./2.0).*cos(q1).*(ddz./2.0+(LA.*dq1.^2.*sin(pi./2.0).*sin(q1))./2.0))./2.0+LA.*mlA.*sin(pi./2.0).*cos(q1).*(ddz./4.0+(LA.*dq1.^2.*sin(pi./2.0).*sin(q1))./4.0);-lambdaB.*(LB.*cos(q2).*(z+LB.*sin(q2)).*-2.0+LB.*cos(alphaAB).*sin(q2).*(y+aB.*cos(alphaAB)-eB.*cos(alphaAB)+LB.*cos(alphaAB).*cos(q2)).*2.0+LB.*sin(alphaAB).*sin(q2).*(x+aB.*sin(alphaAB)-eB.*sin(alphaAB)+LB.*cos(q2).*sin(alphaAB)).*2.0)-((((dx-LB.*dq2.*sin(q2).*cos(alphaAB-pi./2.0)).*(y+aB.*cos(alphaAB)-eB.*cos(alphaAB)+LB.*cos(alphaAB).*cos(q2)))./lB-((dy+LB.*dq2.*sin(alphaAB-pi./2.0).*sin(q2)).*(x+aB.*sin(alphaAB)-eB.*sin(alphaAB)+LB.*cos(q2).*sin(alphaAB)))./lB).*((IlBxz.*((LB.*cos(q2).*(dy+LB.*dq2.*sin(alphaAB-pi./2.0).*sin(q2)))./lB+(LB.*cos(alphaAB).*sin(q2).*(dz+LB.*dq2.*sin(pi./2.0).*cos(q2)))./lB+(LB.*dq2.*sin(alphaAB-pi./2.0).*cos(q2).*(z+LB.*sin(q2)))./lB+(LB.*dq2.*sin(pi./2.0).*sin(q2).*(y+aB.*cos(alphaAB)-eB.*cos(alphaAB)+LB.*cos(alphaAB).*cos(q2)))./lB).*(-1.0./2.0))./lB+(IlByz.*((LB.*cos(q2).*(dx-LB.*dq2.*sin(q2).*cos(alphaAB-pi./2.0)))./lB+(LB.*sin(alphaAB).*sin(q2).*(dz+LB.*dq2.*sin(pi./2.0).*cos(q2)))./lB-(LB.*dq2.*cos(q2).*cos(alphaAB-pi./2.0).*(z+LB.*sin(q2)))./lB+(LB.*dq2.*sin(pi./2.0).*sin(q2).*(x+aB.*sin(alphaAB)-eB.*sin(alphaAB)+LB.*cos(q2).*sin(alphaAB)))./lB))./(lB.*2.0)+(IlBzz.*((LB.*cos(alphaAB).*sin(q2).*(dx-LB.*dq2.*sin(q2).*cos(alphaAB-pi./2.0)))./lB-(LB.*sin(alphaAB).*sin(q2).*(dy+LB.*dq2.*sin(alphaAB-pi./2.0).*sin(q2)))./lB+(LB.*dq2.*sin(alphaAB-pi./2.0).*cos(q2).*(x+aB.*sin(alphaAB)-eB.*sin(alphaAB)+LB.*cos(q2).*sin(alphaAB)))./lB+(LB.*dq2.*cos(q2).*cos(alphaAB-pi./2.0).*(y+aB.*cos(alphaAB)-eB.*cos(alphaAB)+LB.*cos(alphaAB).*cos(q2)))./lB))./(lB.*2.0)).*2.0)./lB-((((dx-LB.*dq2.*sin(q2).*cos(alphaAB-pi./2.0)).*(y+aB.*cos(alphaAB)-eB.*cos(alphaAB)+LB.*cos(alphaAB).*cos(q2)))./lB-((dy+LB.*dq2.*sin(alphaAB-pi./2.0).*sin(q2)).*(x+aB.*sin(alphaAB)-eB.*sin(alphaAB)+LB.*cos(q2).*sin(alphaAB)))./lB).*((IlBxz.*((LB.*sin(alphaAB-pi./2.0).*sin(q2).*(dz+LB.*dq2.*cos(q2)))./lB-(LB.*sin(pi./2.0).*cos(q2).*(dy-LB.*dq2.*cos(alphaAB).*sin(q2)))./lB+(LB.*dq2.*sin(alphaAB-pi./2.0).*cos(q2).*(z+LB.*sin(q2)))./lB+(LB.*dq2.*sin(pi./2.0).*sin(q2).*(y+aB.*cos(alphaAB)-eB.*cos(alphaAB)+LB.*cos(alphaAB).*cos(q2)))./lB))./(lB.*2.0)+(IlByz.*((LB.*sin(pi./2.0).*cos(q2).*(dx-LB.*dq2.*sin(alphaAB).*sin(q2)))./lB+(LB.*sin(q2).*cos(alphaAB-pi./2.0).*(dz+LB.*dq2.*cos(q2)))./lB+(LB.*dq2.*cos(q2).*cos(alphaAB-pi./2.0).*(z+LB.*sin(q2)))./lB-(LB.*dq2.*sin(pi./2.0).*sin(q2).*(x+aB.*sin(alphaAB)-eB.*sin(alphaAB)+LB.*cos(q2).*sin(alphaAB)))./lB))./(lB.*2.0)-(IlBzz.*((LB.*sin(q2).*cos(alphaAB-pi./2.0).*(dy-LB.*dq2.*cos(alphaAB).*sin(q2)))./lB+(LB.*sin(alphaAB-pi./2.0).*sin(q2).*(dx-LB.*dq2.*sin(alphaAB).*sin(q2)))./lB+(LB.*dq2.*sin(alphaAB-pi./2.0).*cos(q2).*(x+aB.*sin(alphaAB)-eB.*sin(alphaAB)+LB.*cos(q2).*sin(alphaAB)))./lB+(LB.*dq2.*cos(q2).*cos(alphaAB-pi./2.0).*(y+aB.*cos(alphaAB)-eB.*cos(alphaAB)+LB.*cos(alphaAB).*cos(q2)))./lB))./(lB.*2.0)).*2.0)./lB+(((IlBxz.*((LB.*sin(q2).*cos(alphaAB-pi./2.0).*(y+aB.*cos(alphaAB)-eB.*cos(alphaAB)+LB.*cos(alphaAB).*cos(q2)))./lB+(LB.*sin(alphaAB-pi./2.0).*sin(q2).*(x+aB.*sin(alphaAB)-eB.*sin(alphaAB)+LB.*cos(q2).*sin(alphaAB)))./lB))./(lB.*2.0)+(IlBxx.*((LB.*sin(pi./2.0).*cos(q2).*(y+aB.*cos(alphaAB)-eB.*cos(alphaAB)+LB.*cos(alphaAB).*cos(q2)))./lB-(LB.*sin(alphaAB-pi./2.0).*sin(q2).*(z+LB.*sin(q2)))./lB))./(lB.*2.0)-(IlBxy.*((LB.*sin(q2).*cos(alphaAB-pi./2.0).*(z+LB.*sin(q2)))./lB+(LB.*sin(pi./2.0).*cos(q2).*(x+aB.*sin(alphaAB)-eB.*sin(alphaAB)+LB.*cos(q2).*sin(alphaAB)))./lB))./(lB.*2.0)).*(((dz+LB.*dq2.*cos(q2)).*(dy+LB.*dq2.*sin(alphaAB-pi./2.0).*sin(q2)))./lB-((dy-LB.*dq2.*cos(alphaAB).*sin(q2)).*(dz+LB.*dq2.*sin(pi./2.0).*cos(q2)))./lB+((ddy+LB.*dq2.^2.*sin(alphaAB-pi./2.0).*cos(q2)).*(z+LB.*sin(q2)))./lB-((ddz-LB.*dq2.^2.*sin(pi./2.0).*sin(q2)).*(y+aB.*cos(alphaAB)-eB.*cos(alphaAB)+LB.*cos(alphaAB).*cos(q2)))./lB).*2.0)./lB-(((IlBxz.*(((dx-LB.*dq2.*sin(q2).*cos(alphaAB-pi./2.0)).*(y+aB.*cos(alphaAB)-eB.*cos(alphaAB)+LB.*cos(alphaAB).*cos(q2)))./lB-((dy+LB.*dq2.*sin(alphaAB-pi./2.0).*sin(q2)).*(x+aB.*sin(alphaAB)-eB.*sin(alphaAB)+LB.*cos(q2).*sin(alphaAB)))./lB).*(-1.0./2.0))./lB+(IlBxx.*(((dz+LB.*dq2.*sin(pi./2.0).*cos(q2)).*(y+aB.*cos(alphaAB)-eB.*cos(alphaAB)+LB.*cos(alphaAB).*cos(q2)))./lB-((z+LB.*sin(q2)).*(dy+LB.*dq2.*sin(alphaAB-pi./2.0).*sin(q2)))./lB))./(lB.*2.0)+(IlBxy.*(((z+LB.*sin(q2)).*(dx-LB.*dq2.*sin(q2).*cos(alphaAB-pi./2.0)))./lB-((dz+LB.*dq2.*sin(pi./2.0).*cos(q2)).*(x+aB.*sin(alphaAB)-eB.*sin(alphaAB)+LB.*cos(q2).*sin(alphaAB)))./lB))./(lB.*2.0)).*((LB.*cos(q2).*(dy+LB.*dq2.*sin(alphaAB-pi./2.0).*sin(q2)))./lB+(LB.*cos(alphaAB).*sin(q2).*(dz+LB.*dq2.*sin(pi./2.0).*cos(q2)))./lB+(LB.*dq2.*sin(alphaAB-pi./2.0).*cos(q2).*(z+LB.*sin(q2)))./lB+(LB.*dq2.*sin(pi./2.0).*sin(q2).*(y+aB.*cos(alphaAB)-eB.*cos(alphaAB)+LB.*cos(alphaAB).*cos(q2)))./lB).*2.0)./lB+(((IlBxz.*(((dx-LB.*dq2.*sin(q2).*cos(alphaAB-pi./2.0)).*(y+aB.*cos(alphaAB)-eB.*cos(alphaAB)+LB.*cos(alphaAB).*cos(q2)))./lB-((dy+LB.*dq2.*sin(alphaAB-pi./2.0).*sin(q2)).*(x+aB.*sin(alphaAB)-eB.*sin(alphaAB)+LB.*cos(q2).*sin(alphaAB)))./lB).*(-1.0./2.0))./lB+(IlBxx.*(((dz+LB.*dq2.*sin(pi./2.0).*cos(q2)).*(y+aB.*cos(alphaAB)-eB.*cos(alphaAB)+LB.*cos(alphaAB).*cos(q2)))./lB-((z+LB.*sin(q2)).*(dy+LB.*dq2.*sin(alphaAB-pi./2.0).*sin(q2)))./lB))./(lB.*2.0)+(IlBxy.*(((z+LB.*sin(q2)).*(dx-LB.*dq2.*sin(q2).*cos(alphaAB-pi./2.0)))./lB-((dz+LB.*dq2.*sin(pi./2.0).*cos(q2)).*(x+aB.*sin(alphaAB)-eB.*sin(alphaAB)+LB.*cos(q2).*sin(alphaAB)))./lB))./(lB.*2.0)).*((LB.*sin(alphaAB-pi./2.0).*sin(q2).*(dz+LB.*dq2.*cos(q2)))./lB-(LB.*sin(pi./2.0).*cos(q2).*(dy-LB.*dq2.*cos(alphaAB).*sin(q2)))./lB+(LB.*dq2.*sin(alphaAB-pi./2.0).*cos(q2).*(z+LB.*sin(q2)))./lB+(LB.*dq2.*sin(pi./2.0).*sin(q2).*(y+aB.*cos(alphaAB)-eB.*cos(alphaAB)+LB.*cos(alphaAB).*cos(q2)))./lB).*2.0)./lB+(((LB.*sin(q2).*cos(alphaAB-pi./2.0).*(y+aB.*cos(alphaAB)-eB.*cos(alphaAB)+LB.*cos(alphaAB).*cos(q2)))./lB+(LB.*sin(alphaAB-pi./2.0).*sin(q2).*(x+aB.*sin(alphaAB)-eB.*sin(alphaAB)+LB.*cos(q2).*sin(alphaAB)))./lB).*((IlBxz.*(((dz+LB.*dq2.*cos(q2)).*(dy+LB.*dq2.*sin(alphaAB-pi./2.0).*sin(q2)))./lB-((dy-LB.*dq2.*cos(alphaAB).*sin(q2)).*(dz+LB.*dq2.*sin(pi./2.0).*cos(q2)))./lB+((ddy+LB.*dq2.^2.*sin(alphaAB-pi./2.0).*cos(q2)).*(z+LB.*sin(q2)))./lB-((ddz-LB.*dq2.^2.*sin(pi./2.0).*sin(q2)).*(y+aB.*cos(alphaAB)-eB.*cos(alphaAB)+LB.*cos(alphaAB).*cos(q2)))./lB))./(lB.*2.0)-(IlByz.*(((dz+LB.*dq2.*cos(q2)).*(dx-LB.*dq2.*sin(q2).*cos(alphaAB-pi./2.0)))./lB+((z+LB.*sin(q2)).*(ddx-LB.*dq2.^2.*cos(q2).*cos(alphaAB-pi./2.0)))./lB-((dx-LB.*dq2.*sin(alphaAB).*sin(q2)).*(dz+LB.*dq2.*sin(pi./2.0).*cos(q2)))./lB-((ddz-LB.*dq2.^2.*sin(pi./2.0).*sin(q2)).*(x+aB.*sin(alphaAB)-eB.*sin(alphaAB)+LB.*cos(q2).*sin(alphaAB)))./lB))./(lB.*2.0)+(IlBzz.*(((ddx-LB.*dq2.^2.*cos(q2).*cos(alphaAB-pi./2.0)).*(y+aB.*cos(alphaAB)-eB.*cos(alphaAB)+LB.*cos(alphaAB).*cos(q2)))./lB+((dy-LB.*dq2.*cos(alphaAB).*sin(q2)).*(dx-LB.*dq2.*sin(q2).*cos(alphaAB-pi./2.0)))./lB-((dx-LB.*dq2.*sin(alphaAB).*sin(q2)).*(dy+LB.*dq2.*sin(alphaAB-pi./2.0).*sin(q2)))./lB-((ddy+LB.*dq2.^2.*sin(alphaAB-pi./2.0).*cos(q2)).*(x+aB.*sin(alphaAB)-eB.*sin(alphaAB)+LB.*cos(q2).*sin(alphaAB)))./lB))./(lB.*2.0)).*2.0)./lB-(((IlByz.*((LB.*sin(q2).*cos(alphaAB-pi./2.0).*(y+aB.*cos(alphaAB)-eB.*cos(alphaAB)+LB.*cos(alphaAB).*cos(q2)))./lB+(LB.*sin(alphaAB-pi./2.0).*sin(q2).*(x+aB.*sin(alphaAB)-eB.*sin(alphaAB)+LB.*cos(q2).*sin(alphaAB)))./lB))./(lB.*2.0)+(IlBxy.*((LB.*sin(pi./2.0).*cos(q2).*(y+aB.*cos(alphaAB)-eB.*cos(alphaAB)+LB.*cos(alphaAB).*cos(q2)))./lB-(LB.*sin(alphaAB-pi./2.0).*sin(q2).*(z+LB.*sin(q2)))./lB))./(lB.*2.0)-(IlByy.*((LB.*sin(q2).*cos(alphaAB-pi./2.0).*(z+LB.*sin(q2)))./lB+(LB.*sin(pi./2.0).*cos(q2).*(x+aB.*sin(alphaAB)-eB.*sin(alphaAB)+LB.*cos(q2).*sin(alphaAB)))./lB))./(lB.*2.0)).*(((dz+LB.*dq2.*cos(q2)).*(dx-LB.*dq2.*sin(q2).*cos(alphaAB-pi./2.0)))./lB+((z+LB.*sin(q2)).*(ddx-LB.*dq2.^2.*cos(q2).*cos(alphaAB-pi./2.0)))./lB-((dx-LB.*dq2.*sin(alphaAB).*sin(q2)).*(dz+LB.*dq2.*sin(pi./2.0).*cos(q2)))./lB-((ddz-LB.*dq2.^2.*sin(pi./2.0).*sin(q2)).*(x+aB.*sin(alphaAB)-eB.*sin(alphaAB)+LB.*cos(q2).*sin(alphaAB)))./lB).*2.0)./lB+(((IlBzz.*((LB.*sin(q2).*cos(alphaAB-pi./2.0).*(y+aB.*cos(alphaAB)-eB.*cos(alphaAB)+LB.*cos(alphaAB).*cos(q2)))./lB+(LB.*sin(alphaAB-pi./2.0).*sin(q2).*(x+aB.*sin(alphaAB)-eB.*sin(alphaAB)+LB.*cos(q2).*sin(alphaAB)))./lB))./(lB.*2.0)+(IlBxz.*((LB.*sin(pi./2.0).*cos(q2).*(y+aB.*cos(alphaAB)-eB.*cos(alphaAB)+LB.*cos(alphaAB).*cos(q2)))./lB-(LB.*sin(alphaAB-pi./2.0).*sin(q2).*(z+LB.*sin(q2)))./lB))./(lB.*2.0)-(IlByz.*((LB.*sin(q2).*cos(alphaAB-pi./2.0).*(z+LB.*sin(q2)))./lB+(LB.*sin(pi./2.0).*cos(q2).*(x+aB.*sin(alphaAB)-eB.*sin(alphaAB)+LB.*cos(q2).*sin(alphaAB)))./lB))./(lB.*2.0)).*(((ddx-LB.*dq2.^2.*cos(q2).*cos(alphaAB-pi./2.0)).*(y+aB.*cos(alphaAB)-eB.*cos(alphaAB)+LB.*cos(alphaAB).*cos(q2)))./lB+((dy-LB.*dq2.*cos(alphaAB).*sin(q2)).*(dx-LB.*dq2.*sin(q2).*cos(alphaAB-pi./2.0)))./lB-((dx-LB.*dq2.*sin(alphaAB).*sin(q2)).*(dy+LB.*dq2.*sin(alphaAB-pi./2.0).*sin(q2)))./lB-((ddy+LB.*dq2.^2.*sin(alphaAB-pi./2.0).*cos(q2)).*(x+aB.*sin(alphaAB)-eB.*sin(alphaAB)+LB.*cos(q2).*sin(alphaAB)))./lB).*2.0)./lB+(((IlByz.*(((dx-LB.*dq2.*sin(q2).*cos(alphaAB-pi./2.0)).*(y+aB.*cos(alphaAB)-eB.*cos(alphaAB)+LB.*cos(alphaAB).*cos(q2)))./lB-((dy+LB.*dq2.*sin(alphaAB-pi./2.0).*sin(q2)).*(x+aB.*sin(alphaAB)-eB.*sin(alphaAB)+LB.*cos(q2).*sin(alphaAB)))./lB).*(-1.0./2.0))./lB+(IlBxy.*(((dz+LB.*dq2.*sin(pi./2.0).*cos(q2)).*(y+aB.*cos(alphaAB)-eB.*cos(alphaAB)+LB.*cos(alphaAB).*cos(q2)))./lB-((z+LB.*sin(q2)).*(dy+LB.*dq2.*sin(alphaAB-pi./2.0).*sin(q2)))./lB))./(lB.*2.0)+(IlByy.*(((z+LB.*sin(q2)).*(dx-LB.*dq2.*sin(q2).*cos(alphaAB-pi./2.0)))./lB-((dz+LB.*dq2.*sin(pi./2.0).*cos(q2)).*(x+aB.*sin(alphaAB)-eB.*sin(alphaAB)+LB.*cos(q2).*sin(alphaAB)))./lB))./(lB.*2.0)).*((LB.*cos(q2).*(dx-LB.*dq2.*sin(q2).*cos(alphaAB-pi./2.0)))./lB+(LB.*sin(alphaAB).*sin(q2).*(dz+LB.*dq2.*sin(pi./2.0).*cos(q2)))./lB-(LB.*dq2.*cos(q2).*cos(alphaAB-pi./2.0).*(z+LB.*sin(q2)))./lB+(LB.*dq2.*sin(pi./2.0).*sin(q2).*(x+aB.*sin(alphaAB)-eB.*sin(alphaAB)+LB.*cos(q2).*sin(alphaAB)))./lB).*2.0)./lB+(((IlByz.*(((dx-LB.*dq2.*sin(q2).*cos(alphaAB-pi./2.0)).*(y+aB.*cos(alphaAB)-eB.*cos(alphaAB)+LB.*cos(alphaAB).*cos(q2)))./lB-((dy+LB.*dq2.*sin(alphaAB-pi./2.0).*sin(q2)).*(x+aB.*sin(alphaAB)-eB.*sin(alphaAB)+LB.*cos(q2).*sin(alphaAB)))./lB).*(-1.0./2.0))./lB+(IlBxy.*(((dz+LB.*dq2.*sin(pi./2.0).*cos(q2)).*(y+aB.*cos(alphaAB)-eB.*cos(alphaAB)+LB.*cos(alphaAB).*cos(q2)))./lB-((z+LB.*sin(q2)).*(dy+LB.*dq2.*sin(alphaAB-pi./2.0).*sin(q2)))./lB))./(lB.*2.0)+(IlByy.*(((z+LB.*sin(q2)).*(dx-LB.*dq2.*sin(q2).*cos(alphaAB-pi./2.0)))./lB-((dz+LB.*dq2.*sin(pi./2.0).*cos(q2)).*(x+aB.*sin(alphaAB)-eB.*sin(alphaAB)+LB.*cos(q2).*sin(alphaAB)))./lB))./(lB.*2.0)).*((LB.*sin(pi./2.0).*cos(q2).*(dx-LB.*dq2.*sin(alphaAB).*sin(q2)))./lB+(LB.*sin(q2).*cos(alphaAB-pi./2.0).*(dz+LB.*dq2.*cos(q2)))./lB+(LB.*dq2.*cos(q2).*cos(alphaAB-pi./2.0).*(z+LB.*sin(q2)))./lB-(LB.*dq2.*sin(pi./2.0).*sin(q2).*(x+aB.*sin(alphaAB)-eB.*sin(alphaAB)+LB.*cos(q2).*sin(alphaAB)))./lB).*2.0)./lB+((((dz+LB.*dq2.*sin(pi./2.0).*cos(q2)).*(y+aB.*cos(alphaAB)-eB.*cos(alphaAB)+LB.*cos(alphaAB).*cos(q2)))./lB-((z+LB.*sin(q2)).*(dy+LB.*dq2.*sin(alphaAB-pi./2.0).*sin(q2)))./lB).*((IlBxx.*((LB.*cos(q2).*(dy+LB.*dq2.*sin(alphaAB-pi./2.0).*sin(q2)))./lB+(LB.*cos(alphaAB).*sin(q2).*(dz+LB.*dq2.*sin(pi./2.0).*cos(q2)))./lB+(LB.*dq2.*sin(alphaAB-pi./2.0).*cos(q2).*(z+LB.*sin(q2)))./lB+(LB.*dq2.*sin(pi./2.0).*sin(q2).*(y+aB.*cos(alphaAB)-eB.*cos(alphaAB)+LB.*cos(alphaAB).*cos(q2)))./lB).*(-1.0./2.0))./lB+(IlBxy.*((LB.*cos(q2).*(dx-LB.*dq2.*sin(q2).*cos(alphaAB-pi./2.0)))./lB+(LB.*sin(alphaAB).*sin(q2).*(dz+LB.*dq2.*sin(pi./2.0).*cos(q2)))./lB-(LB.*dq2.*cos(q2).*cos(alphaAB-pi./2.0).*(z+LB.*sin(q2)))./lB+(LB.*dq2.*sin(pi./2.0).*sin(q2).*(x+aB.*sin(alphaAB)-eB.*sin(alphaAB)+LB.*cos(q2).*sin(alphaAB)))./lB))./(lB.*2.0)+(IlBxz.*((LB.*cos(alphaAB).*sin(q2).*(dx-LB.*dq2.*sin(q2).*cos(alphaAB-pi./2.0)))./lB-(LB.*sin(alphaAB).*sin(q2).*(dy+LB.*dq2.*sin(alphaAB-pi./2.0).*sin(q2)))./lB+(LB.*dq2.*sin(alphaAB-pi./2.0).*cos(q2).*(x+aB.*sin(alphaAB)-eB.*sin(alphaAB)+LB.*cos(q2).*sin(alphaAB)))./lB+(LB.*dq2.*cos(q2).*cos(alphaAB-pi./2.0).*(y+aB.*cos(alphaAB)-eB.*cos(alphaAB)+LB.*cos(alphaAB).*cos(q2)))./lB))./(lB.*2.0)).*2.0)./lB+((((dz+LB.*dq2.*sin(pi./2.0).*cos(q2)).*(y+aB.*cos(alphaAB)-eB.*cos(alphaAB)+LB.*cos(alphaAB).*cos(q2)))./lB-((z+LB.*sin(q2)).*(dy+LB.*dq2.*sin(alphaAB-pi./2.0).*sin(q2)))./lB).*((IlBxx.*((LB.*sin(alphaAB-pi./2.0).*sin(q2).*(dz+LB.*dq2.*cos(q2)))./lB-(LB.*sin(pi./2.0).*cos(q2).*(dy-LB.*dq2.*cos(alphaAB).*sin(q2)))./lB+(LB.*dq2.*sin(alphaAB-pi./2.0).*cos(q2).*(z+LB.*sin(q2)))./lB+(LB.*dq2.*sin(pi./2.0).*sin(q2).*(y+aB.*cos(alphaAB)-eB.*cos(alphaAB)+LB.*cos(alphaAB).*cos(q2)))./lB))./(lB.*2.0)+(IlBxy.*((LB.*sin(pi./2.0).*cos(q2).*(dx-LB.*dq2.*sin(alphaAB).*sin(q2)))./lB+(LB.*sin(q2).*cos(alphaAB-pi./2.0).*(dz+LB.*dq2.*cos(q2)))./lB+(LB.*dq2.*cos(q2).*cos(alphaAB-pi./2.0).*(z+LB.*sin(q2)))./lB-(LB.*dq2.*sin(pi./2.0).*sin(q2).*(x+aB.*sin(alphaAB)-eB.*sin(alphaAB)+LB.*cos(q2).*sin(alphaAB)))./lB))./(lB.*2.0)-(IlBxz.*((LB.*sin(q2).*cos(alphaAB-pi./2.0).*(dy-LB.*dq2.*cos(alphaAB).*sin(q2)))./lB+(LB.*sin(alphaAB-pi./2.0).*sin(q2).*(dx-LB.*dq2.*sin(alphaAB).*sin(q2)))./lB+(LB.*dq2.*sin(alphaAB-pi./2.0).*cos(q2).*(x+aB.*sin(alphaAB)-eB.*sin(alphaAB)+LB.*cos(q2).*sin(alphaAB)))./lB+(LB.*dq2.*cos(q2).*cos(alphaAB-pi./2.0).*(y+aB.*cos(alphaAB)-eB.*cos(alphaAB)+LB.*cos(alphaAB).*cos(q2)))./lB))./(lB.*2.0)).*2.0)./lB+(((IlBzz.*(((dx-LB.*dq2.*sin(q2).*cos(alphaAB-pi./2.0)).*(y+aB.*cos(alphaAB)-eB.*cos(alphaAB)+LB.*cos(alphaAB).*cos(q2)))./lB-((dy+LB.*dq2.*sin(alphaAB-pi./2.0).*sin(q2)).*(x+aB.*sin(alphaAB)-eB.*sin(alphaAB)+LB.*cos(q2).*sin(alphaAB)))./lB).*(-1.0./2.0))./lB+(IlBxz.*(((dz+LB.*dq2.*sin(pi./2.0).*cos(q2)).*(y+aB.*cos(alphaAB)-eB.*cos(alphaAB)+LB.*cos(alphaAB).*cos(q2)))./lB-((z+LB.*sin(q2)).*(dy+LB.*dq2.*sin(alphaAB-pi./2.0).*sin(q2)))./lB))./(lB.*2.0)+(IlByz.*(((z+LB.*sin(q2)).*(dx-LB.*dq2.*sin(q2).*cos(alphaAB-pi./2.0)))./lB-((dz+LB.*dq2.*sin(pi./2.0).*cos(q2)).*(x+aB.*sin(alphaAB)-eB.*sin(alphaAB)+LB.*cos(q2).*sin(alphaAB)))./lB))./(lB.*2.0)).*((LB.*cos(alphaAB).*sin(q2).*(dx-LB.*dq2.*sin(q2).*cos(alphaAB-pi./2.0)))./lB-(LB.*sin(alphaAB).*sin(q2).*(dy+LB.*dq2.*sin(alphaAB-pi./2.0).*sin(q2)))./lB+(LB.*dq2.*sin(alphaAB-pi./2.0).*cos(q2).*(x+aB.*sin(alphaAB)-eB.*sin(alphaAB)+LB.*cos(q2).*sin(alphaAB)))./lB+(LB.*dq2.*cos(q2).*cos(alphaAB-pi./2.0).*(y+aB.*cos(alphaAB)-eB.*cos(alphaAB)+LB.*cos(alphaAB).*cos(q2)))./lB).*2.0)./lB-(((IlBzz.*(((dx-LB.*dq2.*sin(q2).*cos(alphaAB-pi./2.0)).*(y+aB.*cos(alphaAB)-eB.*cos(alphaAB)+LB.*cos(alphaAB).*cos(q2)))./lB-((dy+LB.*dq2.*sin(alphaAB-pi./2.0).*sin(q2)).*(x+aB.*sin(alphaAB)-eB.*sin(alphaAB)+LB.*cos(q2).*sin(alphaAB)))./lB).*(-1.0./2.0))./lB+(IlBxz.*(((dz+LB.*dq2.*sin(pi./2.0).*cos(q2)).*(y+aB.*cos(alphaAB)-eB.*cos(alphaAB)+LB.*cos(alphaAB).*cos(q2)))./lB-((z+LB.*sin(q2)).*(dy+LB.*dq2.*sin(alphaAB-pi./2.0).*sin(q2)))./lB))./(lB.*2.0)+(IlByz.*(((z+LB.*sin(q2)).*(dx-LB.*dq2.*sin(q2).*cos(alphaAB-pi./2.0)))./lB-((dz+LB.*dq2.*sin(pi./2.0).*cos(q2)).*(x+aB.*sin(alphaAB)-eB.*sin(alphaAB)+LB.*cos(q2).*sin(alphaAB)))./lB))./(lB.*2.0)).*((LB.*sin(q2).*cos(alphaAB-pi./2.0).*(dy-LB.*dq2.*cos(alphaAB).*sin(q2)))./lB+(LB.*sin(alphaAB-pi./2.0).*sin(q2).*(dx-LB.*dq2.*sin(alphaAB).*sin(q2)))./lB+(LB.*dq2.*sin(alphaAB-pi./2.0).*cos(q2).*(x+aB.*sin(alphaAB)-eB.*sin(alphaAB)+LB.*cos(q2).*sin(alphaAB)))./lB+(LB.*dq2.*cos(q2).*cos(alphaAB-pi./2.0).*(y+aB.*cos(alphaAB)-eB.*cos(alphaAB)+LB.*cos(alphaAB).*cos(q2)))./lB).*2.0)./lB+((((z+LB.*sin(q2)).*(dx-LB.*dq2.*sin(q2).*cos(alphaAB-pi./2.0)))./lB-((dz+LB.*dq2.*sin(pi./2.0).*cos(q2)).*(x+aB.*sin(alphaAB)-eB.*sin(alphaAB)+LB.*cos(q2).*sin(alphaAB)))./lB).*((IlBxy.*((LB.*cos(q2).*(dy+LB.*dq2.*sin(alphaAB-pi./2.0).*sin(q2)))./lB+(LB.*cos(alphaAB).*sin(q2).*(dz+LB.*dq2.*sin(pi./2.0).*cos(q2)))./lB+(LB.*dq2.*sin(alphaAB-pi./2.0).*cos(q2).*(z+LB.*sin(q2)))./lB+(LB.*dq2.*sin(pi./2.0).*sin(q2).*(y+aB.*cos(alphaAB)-eB.*cos(alphaAB)+LB.*cos(alphaAB).*cos(q2)))./lB).*(-1.0./2.0))./lB+(IlByy.*((LB.*cos(q2).*(dx-LB.*dq2.*sin(q2).*cos(alphaAB-pi./2.0)))./lB+(LB.*sin(alphaAB).*sin(q2).*(dz+LB.*dq2.*sin(pi./2.0).*cos(q2)))./lB-(LB.*dq2.*cos(q2).*cos(alphaAB-pi./2.0).*(z+LB.*sin(q2)))./lB+(LB.*dq2.*sin(pi./2.0).*sin(q2).*(x+aB.*sin(alphaAB)-eB.*sin(alphaAB)+LB.*cos(q2).*sin(alphaAB)))./lB))./(lB.*2.0)+(IlByz.*((LB.*cos(alphaAB).*sin(q2).*(dx-LB.*dq2.*sin(q2).*cos(alphaAB-pi./2.0)))./lB-(LB.*sin(alphaAB).*sin(q2).*(dy+LB.*dq2.*sin(alphaAB-pi./2.0).*sin(q2)))./lB+(LB.*dq2.*sin(alphaAB-pi./2.0).*cos(q2).*(x+aB.*sin(alphaAB)-eB.*sin(alphaAB)+LB.*cos(q2).*sin(alphaAB)))./lB+(LB.*dq2.*cos(q2).*cos(alphaAB-pi./2.0).*(y+aB.*cos(alphaAB)-eB.*cos(alphaAB)+LB.*cos(alphaAB).*cos(q2)))./lB))./(lB.*2.0)).*2.0)./lB+((((z+LB.*sin(q2)).*(dx-LB.*dq2.*sin(q2).*cos(alphaAB-pi./2.0)))./lB-((dz+LB.*dq2.*sin(pi./2.0).*cos(q2)).*(x+aB.*sin(alphaAB)-eB.*sin(alphaAB)+LB.*cos(q2).*sin(alphaAB)))./lB).*((IlBxy.*((LB.*sin(alphaAB-pi./2.0).*sin(q2).*(dz+LB.*dq2.*cos(q2)))./lB-(LB.*sin(pi./2.0).*cos(q2).*(dy-LB.*dq2.*cos(alphaAB).*sin(q2)))./lB+(LB.*dq2.*sin(alphaAB-pi./2.0).*cos(q2).*(z+LB.*sin(q2)))./lB+(LB.*dq2.*sin(pi./2.0).*sin(q2).*(y+aB.*cos(alphaAB)-eB.*cos(alphaAB)+LB.*cos(alphaAB).*cos(q2)))./lB))./(lB.*2.0)+(IlByy.*((LB.*sin(pi./2.0).*cos(q2).*(dx-LB.*dq2.*sin(alphaAB).*sin(q2)))./lB+(LB.*sin(q2).*cos(alphaAB-pi./2.0).*(dz+LB.*dq2.*cos(q2)))./lB+(LB.*dq2.*cos(q2).*cos(alphaAB-pi./2.0).*(z+LB.*sin(q2)))./lB-(LB.*dq2.*sin(pi./2.0).*sin(q2).*(x+aB.*sin(alphaAB)-eB.*sin(alphaAB)+LB.*cos(q2).*sin(alphaAB)))./lB))./(lB.*2.0)-(IlByz.*((LB.*sin(q2).*cos(alphaAB-pi./2.0).*(dy-LB.*dq2.*cos(alphaAB).*sin(q2)))./lB+(LB.*sin(alphaAB-pi./2.0).*sin(q2).*(dx-LB.*dq2.*sin(alphaAB).*sin(q2)))./lB+(LB.*dq2.*sin(alphaAB-pi./2.0).*cos(q2).*(x+aB.*sin(alphaAB)-eB.*sin(alphaAB)+LB.*cos(q2).*sin(alphaAB)))./lB+(LB.*dq2.*cos(q2).*cos(alphaAB-pi./2.0).*(y+aB.*cos(alphaAB)-eB.*cos(alphaAB)+LB.*cos(alphaAB).*cos(q2)))./lB))./(lB.*2.0)).*2.0)./lB+(((LB.*sin(pi./2.0).*cos(q2).*(y+aB.*cos(alphaAB)-eB.*cos(alphaAB)+LB.*cos(alphaAB).*cos(q2)))./lB-(LB.*sin(alphaAB-pi./2.0).*sin(q2).*(z+LB.*sin(q2)))./lB).*((IlBxx.*(((dz+LB.*dq2.*cos(q2)).*(dy+LB.*dq2.*sin(alphaAB-pi./2.0).*sin(q2)))./lB-((dy-LB.*dq2.*cos(alphaAB).*sin(q2)).*(dz+LB.*dq2.*sin(pi./2.0).*cos(q2)))./lB+((ddy+LB.*dq2.^2.*sin(alphaAB-pi./2.0).*cos(q2)).*(z+LB.*sin(q2)))./lB-((ddz-LB.*dq2.^2.*sin(pi./2.0).*sin(q2)).*(y+aB.*cos(alphaAB)-eB.*cos(alphaAB)+LB.*cos(alphaAB).*cos(q2)))./lB))./(lB.*2.0)-(IlBxy.*(((dz+LB.*dq2.*cos(q2)).*(dx-LB.*dq2.*sin(q2).*cos(alphaAB-pi./2.0)))./lB+((z+LB.*sin(q2)).*(ddx-LB.*dq2.^2.*cos(q2).*cos(alphaAB-pi./2.0)))./lB-((dx-LB.*dq2.*sin(alphaAB).*sin(q2)).*(dz+LB.*dq2.*sin(pi./2.0).*cos(q2)))./lB-((ddz-LB.*dq2.^2.*sin(pi./2.0).*sin(q2)).*(x+aB.*sin(alphaAB)-eB.*sin(alphaAB)+LB.*cos(q2).*sin(alphaAB)))./lB))./(lB.*2.0)+(IlBxz.*(((ddx-LB.*dq2.^2.*cos(q2).*cos(alphaAB-pi./2.0)).*(y+aB.*cos(alphaAB)-eB.*cos(alphaAB)+LB.*cos(alphaAB).*cos(q2)))./lB+((dy-LB.*dq2.*cos(alphaAB).*sin(q2)).*(dx-LB.*dq2.*sin(q2).*cos(alphaAB-pi./2.0)))./lB-((dx-LB.*dq2.*sin(alphaAB).*sin(q2)).*(dy+LB.*dq2.*sin(alphaAB-pi./2.0).*sin(q2)))./lB-((ddy+LB.*dq2.^2.*sin(alphaAB-pi./2.0).*cos(q2)).*(x+aB.*sin(alphaAB)-eB.*sin(alphaAB)+LB.*cos(q2).*sin(alphaAB)))./lB))./(lB.*2.0)).*2.0)./lB-(((LB.*sin(q2).*cos(alphaAB-pi./2.0).*(z+LB.*sin(q2)))./lB+(LB.*sin(pi./2.0).*cos(q2).*(x+aB.*sin(alphaAB)-eB.*sin(alphaAB)+LB.*cos(q2).*sin(alphaAB)))./lB).*((IlBxy.*(((dz+LB.*dq2.*cos(q2)).*(dy+LB.*dq2.*sin(alphaAB-pi./2.0).*sin(q2)))./lB-((dy-LB.*dq2.*cos(alphaAB).*sin(q2)).*(dz+LB.*dq2.*sin(pi./2.0).*cos(q2)))./lB+((ddy+LB.*dq2.^2.*sin(alphaAB-pi./2.0).*cos(q2)).*(z+LB.*sin(q2)))./lB-((ddz-LB.*dq2.^2.*sin(pi./2.0).*sin(q2)).*(y+aB.*cos(alphaAB)-eB.*cos(alphaAB)+LB.*cos(alphaAB).*cos(q2)))./lB))./(lB.*2.0)-(IlByy.*(((dz+LB.*dq2.*cos(q2)).*(dx-LB.*dq2.*sin(q2).*cos(alphaAB-pi./2.0)))./lB+((z+LB.*sin(q2)).*(ddx-LB.*dq2.^2.*cos(q2).*cos(alphaAB-pi./2.0)))./lB-((dx-LB.*dq2.*sin(alphaAB).*sin(q2)).*(dz+LB.*dq2.*sin(pi./2.0).*cos(q2)))./lB-((ddz-LB.*dq2.^2.*sin(pi./2.0).*sin(q2)).*(x+aB.*sin(alphaAB)-eB.*sin(alphaAB)+LB.*cos(q2).*sin(alphaAB)))./lB))./(lB.*2.0)+(IlByz.*(((ddx-LB.*dq2.^2.*cos(q2).*cos(alphaAB-pi./2.0)).*(y+aB.*cos(alphaAB)-eB.*cos(alphaAB)+LB.*cos(alphaAB).*cos(q2)))./lB+((dy-LB.*dq2.*cos(alphaAB).*sin(q2)).*(dx-LB.*dq2.*sin(q2).*cos(alphaAB-pi./2.0)))./lB-((dx-LB.*dq2.*sin(alphaAB).*sin(q2)).*(dy+LB.*dq2.*sin(alphaAB-pi./2.0).*sin(q2)))./lB-((ddy+LB.*dq2.^2.*sin(alphaAB-pi./2.0).*cos(q2)).*(x+aB.*sin(alphaAB)-eB.*sin(alphaAB)+LB.*cos(q2).*sin(alphaAB)))./lB))./(lB.*2.0)).*2.0)./lB-(LB.*g.*mLB.*cos(q2))./2.0-LB.*g.*mlB.*cos(q2)-(LB.*mlB.*sin(q2).*cos(alphaAB-pi./2.0).*(ddx./2.0+(LB.*dq2.^2.*cos(q2).*cos(alphaAB-pi./2.0))./2.0))./2.0-LB.*mlB.*sin(q2).*cos(alphaAB-pi./2.0).*(ddx./4.0+(LB.*dq2.^2.*cos(q2).*cos(alphaAB-pi./2.0))./4.0)+(LB.*mlB.*sin(alphaAB-pi./2.0).*sin(q2).*(ddy./2.0-(LB.*dq2.^2.*sin(alphaAB-pi./2.0).*cos(q2))./2.0))./2.0+LB.*mlB.*sin(alphaAB-pi./2.0).*sin(q2).*(ddy./4.0-(LB.*dq2.^2.*sin(alphaAB-pi./2.0).*cos(q2))./4.0)+(LB.*mlB.*sin(pi./2.0).*cos(q2).*(ddz./2.0+(LB.*dq2.^2.*sin(pi./2.0).*sin(q2))./2.0))./2.0+LB.*mlB.*sin(pi./2.0).*cos(q2).*(ddz./4.0+(LB.*dq2.^2.*sin(pi./2.0).*sin(q2))./4.0);-lambdaC.*(LC.*cos(q3).*(z+LC.*sin(q3)).*-2.0+LC.*cos(alphaAC).*sin(q3).*(y+aC.*cos(alphaAC)-eC.*cos(alphaAC)+LC.*cos(alphaAC).*cos(q3)).*2.0+LC.*sin(alphaAC).*sin(q3).*(x+aC.*sin(alphaAC)-eC.*sin(alphaAC)+LC.*cos(q3).*sin(alphaAC)).*2.0)-((((dx-LC.*dq3.*sin(q3).*cos(alphaAC-pi./2.0)).*(y+aC.*cos(alphaAC)-eC.*cos(alphaAC)+LC.*cos(alphaAC).*cos(q3)))./lC-((dy+LC.*dq3.*sin(alphaAC-pi./2.0).*sin(q3)).*(x+aC.*sin(alphaAC)-eC.*sin(alphaAC)+LC.*cos(q3).*sin(alphaAC)))./lC).*((IlCxz.*((LC.*cos(q3).*(dy+LC.*dq3.*sin(alphaAC-pi./2.0).*sin(q3)))./lC+(LC.*cos(alphaAC).*sin(q3).*(dz+LC.*dq3.*sin(pi./2.0).*cos(q3)))./lC+(LC.*dq3.*sin(alphaAC-pi./2.0).*cos(q3).*(z+LC.*sin(q3)))./lC+(LC.*dq3.*sin(pi./2.0).*sin(q3).*(y+aC.*cos(alphaAC)-eC.*cos(alphaAC)+LC.*cos(alphaAC).*cos(q3)))./lC).*(-1.0./2.0))./lC+(IlCyz.*((LC.*cos(q3).*(dx-LC.*dq3.*sin(q3).*cos(alphaAC-pi./2.0)))./lC+(LC.*sin(alphaAC).*sin(q3).*(dz+LC.*dq3.*sin(pi./2.0).*cos(q3)))./lC-(LC.*dq3.*cos(q3).*cos(alphaAC-pi./2.0).*(z+LC.*sin(q3)))./lC+(LC.*dq3.*sin(pi./2.0).*sin(q3).*(x+aC.*sin(alphaAC)-eC.*sin(alphaAC)+LC.*cos(q3).*sin(alphaAC)))./lC))./(lC.*2.0)+(IlCzz.*((LC.*cos(alphaAC).*sin(q3).*(dx-LC.*dq3.*sin(q3).*cos(alphaAC-pi./2.0)))./lC-(LC.*sin(alphaAC).*sin(q3).*(dy+LC.*dq3.*sin(alphaAC-pi./2.0).*sin(q3)))./lC+(LC.*dq3.*sin(alphaAC-pi./2.0).*cos(q3).*(x+aC.*sin(alphaAC)-eC.*sin(alphaAC)+LC.*cos(q3).*sin(alphaAC)))./lC+(LC.*dq3.*cos(q3).*cos(alphaAC-pi./2.0).*(y+aC.*cos(alphaAC)-eC.*cos(alphaAC)+LC.*cos(alphaAC).*cos(q3)))./lC))./(lC.*2.0)).*2.0)./lC-((((dx-LC.*dq3.*sin(q3).*cos(alphaAC-pi./2.0)).*(y+aC.*cos(alphaAC)-eC.*cos(alphaAC)+LC.*cos(alphaAC).*cos(q3)))./lC-((dy+LC.*dq3.*sin(alphaAC-pi./2.0).*sin(q3)).*(x+aC.*sin(alphaAC)-eC.*sin(alphaAC)+LC.*cos(q3).*sin(alphaAC)))./lC).*((IlCxz.*((LC.*sin(alphaAC-pi./2.0).*sin(q3).*(dz+LC.*dq3.*cos(q3)))./lC-(LC.*sin(pi./2.0).*cos(q3).*(dy-LC.*dq3.*cos(alphaAC).*sin(q3)))./lC+(LC.*dq3.*sin(alphaAC-pi./2.0).*cos(q3).*(z+LC.*sin(q3)))./lC+(LC.*dq3.*sin(pi./2.0).*sin(q3).*(y+aC.*cos(alphaAC)-eC.*cos(alphaAC)+LC.*cos(alphaAC).*cos(q3)))./lC))./(lC.*2.0)+(IlCyz.*((LC.*sin(pi./2.0).*cos(q3).*(dx-LC.*dq3.*sin(alphaAC).*sin(q3)))./lC+(LC.*sin(q3).*cos(alphaAC-pi./2.0).*(dz+LC.*dq3.*cos(q3)))./lC+(LC.*dq3.*cos(q3).*cos(alphaAC-pi./2.0).*(z+LC.*sin(q3)))./lC-(LC.*dq3.*sin(pi./2.0).*sin(q3).*(x+aC.*sin(alphaAC)-eC.*sin(alphaAC)+LC.*cos(q3).*sin(alphaAC)))./lC))./(lC.*2.0)-(IlCzz.*((LC.*sin(q3).*cos(alphaAC-pi./2.0).*(dy-LC.*dq3.*cos(alphaAC).*sin(q3)))./lC+(LC.*sin(alphaAC-pi./2.0).*sin(q3).*(dx-LC.*dq3.*sin(alphaAC).*sin(q3)))./lC+(LC.*dq3.*sin(alphaAC-pi./2.0).*cos(q3).*(x+aC.*sin(alphaAC)-eC.*sin(alphaAC)+LC.*cos(q3).*sin(alphaAC)))./lC+(LC.*dq3.*cos(q3).*cos(alphaAC-pi./2.0).*(y+aC.*cos(alphaAC)-eC.*cos(alphaAC)+LC.*cos(alphaAC).*cos(q3)))./lC))./(lC.*2.0)).*2.0)./lC+(((IlCxz.*((LC.*sin(q3).*cos(alphaAC-pi./2.0).*(y+aC.*cos(alphaAC)-eC.*cos(alphaAC)+LC.*cos(alphaAC).*cos(q3)))./lC+(LC.*sin(alphaAC-pi./2.0).*sin(q3).*(x+aC.*sin(alphaAC)-eC.*sin(alphaAC)+LC.*cos(q3).*sin(alphaAC)))./lC))./(lC.*2.0)+(IlCxx.*((LC.*sin(pi./2.0).*cos(q3).*(y+aC.*cos(alphaAC)-eC.*cos(alphaAC)+LC.*cos(alphaAC).*cos(q3)))./lC-(LC.*sin(alphaAC-pi./2.0).*sin(q3).*(z+LC.*sin(q3)))./lC))./(lC.*2.0)-(IlCxy.*((LC.*sin(q3).*cos(alphaAC-pi./2.0).*(z+LC.*sin(q3)))./lC+(LC.*sin(pi./2.0).*cos(q3).*(x+aC.*sin(alphaAC)-eC.*sin(alphaAC)+LC.*cos(q3).*sin(alphaAC)))./lC))./(lC.*2.0)).*(((dz+LC.*dq3.*cos(q3)).*(dy+LC.*dq3.*sin(alphaAC-pi./2.0).*sin(q3)))./lC-((dy-LC.*dq3.*cos(alphaAC).*sin(q3)).*(dz+LC.*dq3.*sin(pi./2.0).*cos(q3)))./lC+((ddy+LC.*dq3.^2.*sin(alphaAC-pi./2.0).*cos(q3)).*(z+LC.*sin(q3)))./lC-((ddz-LC.*dq3.^2.*sin(pi./2.0).*sin(q3)).*(y+aC.*cos(alphaAC)-eC.*cos(alphaAC)+LC.*cos(alphaAC).*cos(q3)))./lC).*2.0)./lC-(((IlCxz.*(((dx-LC.*dq3.*sin(q3).*cos(alphaAC-pi./2.0)).*(y+aC.*cos(alphaAC)-eC.*cos(alphaAC)+LC.*cos(alphaAC).*cos(q3)))./lC-((dy+LC.*dq3.*sin(alphaAC-pi./2.0).*sin(q3)).*(x+aC.*sin(alphaAC)-eC.*sin(alphaAC)+LC.*cos(q3).*sin(alphaAC)))./lC).*(-1.0./2.0))./lC+(IlCxx.*(((dz+LC.*dq3.*sin(pi./2.0).*cos(q3)).*(y+aC.*cos(alphaAC)-eC.*cos(alphaAC)+LC.*cos(alphaAC).*cos(q3)))./lC-((z+LC.*sin(q3)).*(dy+LC.*dq3.*sin(alphaAC-pi./2.0).*sin(q3)))./lC))./(lC.*2.0)+(IlCxy.*(((z+LC.*sin(q3)).*(dx-LC.*dq3.*sin(q3).*cos(alphaAC-pi./2.0)))./lC-((dz+LC.*dq3.*sin(pi./2.0).*cos(q3)).*(x+aC.*sin(alphaAC)-eC.*sin(alphaAC)+LC.*cos(q3).*sin(alphaAC)))./lC))./(lC.*2.0)).*((LC.*cos(q3).*(dy+LC.*dq3.*sin(alphaAC-pi./2.0).*sin(q3)))./lC+(LC.*cos(alphaAC).*sin(q3).*(dz+LC.*dq3.*sin(pi./2.0).*cos(q3)))./lC+(LC.*dq3.*sin(alphaAC-pi./2.0).*cos(q3).*(z+LC.*sin(q3)))./lC+(LC.*dq3.*sin(pi./2.0).*sin(q3).*(y+aC.*cos(alphaAC)-eC.*cos(alphaAC)+LC.*cos(alphaAC).*cos(q3)))./lC).*2.0)./lC+(((IlCxz.*(((dx-LC.*dq3.*sin(q3).*cos(alphaAC-pi./2.0)).*(y+aC.*cos(alphaAC)-eC.*cos(alphaAC)+LC.*cos(alphaAC).*cos(q3)))./lC-((dy+LC.*dq3.*sin(alphaAC-pi./2.0).*sin(q3)).*(x+aC.*sin(alphaAC)-eC.*sin(alphaAC)+LC.*cos(q3).*sin(alphaAC)))./lC).*(-1.0./2.0))./lC+(IlCxx.*(((dz+LC.*dq3.*sin(pi./2.0).*cos(q3)).*(y+aC.*cos(alphaAC)-eC.*cos(alphaAC)+LC.*cos(alphaAC).*cos(q3)))./lC-((z+LC.*sin(q3)).*(dy+LC.*dq3.*sin(alphaAC-pi./2.0).*sin(q3)))./lC))./(lC.*2.0)+(IlCxy.*(((z+LC.*sin(q3)).*(dx-LC.*dq3.*sin(q3).*cos(alphaAC-pi./2.0)))./lC-((dz+LC.*dq3.*sin(pi./2.0).*cos(q3)).*(x+aC.*sin(alphaAC)-eC.*sin(alphaAC)+LC.*cos(q3).*sin(alphaAC)))./lC))./(lC.*2.0)).*((LC.*sin(alphaAC-pi./2.0).*sin(q3).*(dz+LC.*dq3.*cos(q3)))./lC-(LC.*sin(pi./2.0).*cos(q3).*(dy-LC.*dq3.*cos(alphaAC).*sin(q3)))./lC+(LC.*dq3.*sin(alphaAC-pi./2.0).*cos(q3).*(z+LC.*sin(q3)))./lC+(LC.*dq3.*sin(pi./2.0).*sin(q3).*(y+aC.*cos(alphaAC)-eC.*cos(alphaAC)+LC.*cos(alphaAC).*cos(q3)))./lC).*2.0)./lC+(((LC.*sin(q3).*cos(alphaAC-pi./2.0).*(y+aC.*cos(alphaAC)-eC.*cos(alphaAC)+LC.*cos(alphaAC).*cos(q3)))./lC+(LC.*sin(alphaAC-pi./2.0).*sin(q3).*(x+aC.*sin(alphaAC)-eC.*sin(alphaAC)+LC.*cos(q3).*sin(alphaAC)))./lC).*((IlCxz.*(((dz+LC.*dq3.*cos(q3)).*(dy+LC.*dq3.*sin(alphaAC-pi./2.0).*sin(q3)))./lC-((dy-LC.*dq3.*cos(alphaAC).*sin(q3)).*(dz+LC.*dq3.*sin(pi./2.0).*cos(q3)))./lC+((ddy+LC.*dq3.^2.*sin(alphaAC-pi./2.0).*cos(q3)).*(z+LC.*sin(q3)))./lC-((ddz-LC.*dq3.^2.*sin(pi./2.0).*sin(q3)).*(y+aC.*cos(alphaAC)-eC.*cos(alphaAC)+LC.*cos(alphaAC).*cos(q3)))./lC))./(lC.*2.0)-(IlCyz.*(((dz+LC.*dq3.*cos(q3)).*(dx-LC.*dq3.*sin(q3).*cos(alphaAC-pi./2.0)))./lC+((z+LC.*sin(q3)).*(ddx-LC.*dq3.^2.*cos(q3).*cos(alphaAC-pi./2.0)))./lC-((dx-LC.*dq3.*sin(alphaAC).*sin(q3)).*(dz+LC.*dq3.*sin(pi./2.0).*cos(q3)))./lC-((ddz-LC.*dq3.^2.*sin(pi./2.0).*sin(q3)).*(x+aC.*sin(alphaAC)-eC.*sin(alphaAC)+LC.*cos(q3).*sin(alphaAC)))./lC))./(lC.*2.0)+(IlCzz.*(((ddx-LC.*dq3.^2.*cos(q3).*cos(alphaAC-pi./2.0)).*(y+aC.*cos(alphaAC)-eC.*cos(alphaAC)+LC.*cos(alphaAC).*cos(q3)))./lC+((dy-LC.*dq3.*cos(alphaAC).*sin(q3)).*(dx-LC.*dq3.*sin(q3).*cos(alphaAC-pi./2.0)))./lC-((dx-LC.*dq3.*sin(alphaAC).*sin(q3)).*(dy+LC.*dq3.*sin(alphaAC-pi./2.0).*sin(q3)))./lC-((ddy+LC.*dq3.^2.*sin(alphaAC-pi./2.0).*cos(q3)).*(x+aC.*sin(alphaAC)-eC.*sin(alphaAC)+LC.*cos(q3).*sin(alphaAC)))./lC))./(lC.*2.0)).*2.0)./lC-(((IlCyz.*((LC.*sin(q3).*cos(alphaAC-pi./2.0).*(y+aC.*cos(alphaAC)-eC.*cos(alphaAC)+LC.*cos(alphaAC).*cos(q3)))./lC+(LC.*sin(alphaAC-pi./2.0).*sin(q3).*(x+aC.*sin(alphaAC)-eC.*sin(alphaAC)+LC.*cos(q3).*sin(alphaAC)))./lC))./(lC.*2.0)+(IlCxy.*((LC.*sin(pi./2.0).*cos(q3).*(y+aC.*cos(alphaAC)-eC.*cos(alphaAC)+LC.*cos(alphaAC).*cos(q3)))./lC-(LC.*sin(alphaAC-pi./2.0).*sin(q3).*(z+LC.*sin(q3)))./lC))./(lC.*2.0)-(IlCyy.*((LC.*sin(q3).*cos(alphaAC-pi./2.0).*(z+LC.*sin(q3)))./lC+(LC.*sin(pi./2.0).*cos(q3).*(x+aC.*sin(alphaAC)-eC.*sin(alphaAC)+LC.*cos(q3).*sin(alphaAC)))./lC))./(lC.*2.0)).*(((dz+LC.*dq3.*cos(q3)).*(dx-LC.*dq3.*sin(q3).*cos(alphaAC-pi./2.0)))./lC+((z+LC.*sin(q3)).*(ddx-LC.*dq3.^2.*cos(q3).*cos(alphaAC-pi./2.0)))./lC-((dx-LC.*dq3.*sin(alphaAC).*sin(q3)).*(dz+LC.*dq3.*sin(pi./2.0).*cos(q3)))./lC-((ddz-LC.*dq3.^2.*sin(pi./2.0).*sin(q3)).*(x+aC.*sin(alphaAC)-eC.*sin(alphaAC)+LC.*cos(q3).*sin(alphaAC)))./lC).*2.0)./lC+(((IlCzz.*((LC.*sin(q3).*cos(alphaAC-pi./2.0).*(y+aC.*cos(alphaAC)-eC.*cos(alphaAC)+LC.*cos(alphaAC).*cos(q3)))./lC+(LC.*sin(alphaAC-pi./2.0).*sin(q3).*(x+aC.*sin(alphaAC)-eC.*sin(alphaAC)+LC.*cos(q3).*sin(alphaAC)))./lC))./(lC.*2.0)+(IlCxz.*((LC.*sin(pi./2.0).*cos(q3).*(y+aC.*cos(alphaAC)-eC.*cos(alphaAC)+LC.*cos(alphaAC).*cos(q3)))./lC-(LC.*sin(alphaAC-pi./2.0).*sin(q3).*(z+LC.*sin(q3)))./lC))./(lC.*2.0)-(IlCyz.*((LC.*sin(q3).*cos(alphaAC-pi./2.0).*(z+LC.*sin(q3)))./lC+(LC.*sin(pi./2.0).*cos(q3).*(x+aC.*sin(alphaAC)-eC.*sin(alphaAC)+LC.*cos(q3).*sin(alphaAC)))./lC))./(lC.*2.0)).*(((ddx-LC.*dq3.^2.*cos(q3).*cos(alphaAC-pi./2.0)).*(y+aC.*cos(alphaAC)-eC.*cos(alphaAC)+LC.*cos(alphaAC).*cos(q3)))./lC+((dy-LC.*dq3.*cos(alphaAC).*sin(q3)).*(dx-LC.*dq3.*sin(q3).*cos(alphaAC-pi./2.0)))./lC-((dx-LC.*dq3.*sin(alphaAC).*sin(q3)).*(dy+LC.*dq3.*sin(alphaAC-pi./2.0).*sin(q3)))./lC-((ddy+LC.*dq3.^2.*sin(alphaAC-pi./2.0).*cos(q3)).*(x+aC.*sin(alphaAC)-eC.*sin(alphaAC)+LC.*cos(q3).*sin(alphaAC)))./lC).*2.0)./lC+(((IlCyz.*(((dx-LC.*dq3.*sin(q3).*cos(alphaAC-pi./2.0)).*(y+aC.*cos(alphaAC)-eC.*cos(alphaAC)+LC.*cos(alphaAC).*cos(q3)))./lC-((dy+LC.*dq3.*sin(alphaAC-pi./2.0).*sin(q3)).*(x+aC.*sin(alphaAC)-eC.*sin(alphaAC)+LC.*cos(q3).*sin(alphaAC)))./lC).*(-1.0./2.0))./lC+(IlCxy.*(((dz+LC.*dq3.*sin(pi./2.0).*cos(q3)).*(y+aC.*cos(alphaAC)-eC.*cos(alphaAC)+LC.*cos(alphaAC).*cos(q3)))./lC-((z+LC.*sin(q3)).*(dy+LC.*dq3.*sin(alphaAC-pi./2.0).*sin(q3)))./lC))./(lC.*2.0)+(IlCyy.*(((z+LC.*sin(q3)).*(dx-LC.*dq3.*sin(q3).*cos(alphaAC-pi./2.0)))./lC-((dz+LC.*dq3.*sin(pi./2.0).*cos(q3)).*(x+aC.*sin(alphaAC)-eC.*sin(alphaAC)+LC.*cos(q3).*sin(alphaAC)))./lC))./(lC.*2.0)).*((LC.*cos(q3).*(dx-LC.*dq3.*sin(q3).*cos(alphaAC-pi./2.0)))./lC+(LC.*sin(alphaAC).*sin(q3).*(dz+LC.*dq3.*sin(pi./2.0).*cos(q3)))./lC-(LC.*dq3.*cos(q3).*cos(alphaAC-pi./2.0).*(z+LC.*sin(q3)))./lC+(LC.*dq3.*sin(pi./2.0).*sin(q3).*(x+aC.*sin(alphaAC)-eC.*sin(alphaAC)+LC.*cos(q3).*sin(alphaAC)))./lC).*2.0)./lC+(((IlCyz.*(((dx-LC.*dq3.*sin(q3).*cos(alphaAC-pi./2.0)).*(y+aC.*cos(alphaAC)-eC.*cos(alphaAC)+LC.*cos(alphaAC).*cos(q3)))./lC-((dy+LC.*dq3.*sin(alphaAC-pi./2.0).*sin(q3)).*(x+aC.*sin(alphaAC)-eC.*sin(alphaAC)+LC.*cos(q3).*sin(alphaAC)))./lC).*(-1.0./2.0))./lC+(IlCxy.*(((dz+LC.*dq3.*sin(pi./2.0).*cos(q3)).*(y+aC.*cos(alphaAC)-eC.*cos(alphaAC)+LC.*cos(alphaAC).*cos(q3)))./lC-((z+LC.*sin(q3)).*(dy+LC.*dq3.*sin(alphaAC-pi./2.0).*sin(q3)))./lC))./(lC.*2.0)+(IlCyy.*(((z+LC.*sin(q3)).*(dx-LC.*dq3.*sin(q3).*cos(alphaAC-pi./2.0)))./lC-((dz+LC.*dq3.*sin(pi./2.0).*cos(q3)).*(x+aC.*sin(alphaAC)-eC.*sin(alphaAC)+LC.*cos(q3).*sin(alphaAC)))./lC))./(lC.*2.0)).*((LC.*sin(pi./2.0).*cos(q3).*(dx-LC.*dq3.*sin(alphaAC).*sin(q3)))./lC+(LC.*sin(q3).*cos(alphaAC-pi./2.0).*(dz+LC.*dq3.*cos(q3)))./lC+(LC.*dq3.*cos(q3).*cos(alphaAC-pi./2.0).*(z+LC.*sin(q3)))./lC-(LC.*dq3.*sin(pi./2.0).*sin(q3).*(x+aC.*sin(alphaAC)-eC.*sin(alphaAC)+LC.*cos(q3).*sin(alphaAC)))./lC).*2.0)./lC+((((dz+LC.*dq3.*sin(pi./2.0).*cos(q3)).*(y+aC.*cos(alphaAC)-eC.*cos(alphaAC)+LC.*cos(alphaAC).*cos(q3)))./lC-((z+LC.*sin(q3)).*(dy+LC.*dq3.*sin(alphaAC-pi./2.0).*sin(q3)))./lC).*((IlCxx.*((LC.*cos(q3).*(dy+LC.*dq3.*sin(alphaAC-pi./2.0).*sin(q3)))./lC+(LC.*cos(alphaAC).*sin(q3).*(dz+LC.*dq3.*sin(pi./2.0).*cos(q3)))./lC+(LC.*dq3.*sin(alphaAC-pi./2.0).*cos(q3).*(z+LC.*sin(q3)))./lC+(LC.*dq3.*sin(pi./2.0).*sin(q3).*(y+aC.*cos(alphaAC)-eC.*cos(alphaAC)+LC.*cos(alphaAC).*cos(q3)))./lC).*(-1.0./2.0))./lC+(IlCxy.*((LC.*cos(q3).*(dx-LC.*dq3.*sin(q3).*cos(alphaAC-pi./2.0)))./lC+(LC.*sin(alphaAC).*sin(q3).*(dz+LC.*dq3.*sin(pi./2.0).*cos(q3)))./lC-(LC.*dq3.*cos(q3).*cos(alphaAC-pi./2.0).*(z+LC.*sin(q3)))./lC+(LC.*dq3.*sin(pi./2.0).*sin(q3).*(x+aC.*sin(alphaAC)-eC.*sin(alphaAC)+LC.*cos(q3).*sin(alphaAC)))./lC))./(lC.*2.0)+(IlCxz.*((LC.*cos(alphaAC).*sin(q3).*(dx-LC.*dq3.*sin(q3).*cos(alphaAC-pi./2.0)))./lC-(LC.*sin(alphaAC).*sin(q3).*(dy+LC.*dq3.*sin(alphaAC-pi./2.0).*sin(q3)))./lC+(LC.*dq3.*sin(alphaAC-pi./2.0).*cos(q3).*(x+aC.*sin(alphaAC)-eC.*sin(alphaAC)+LC.*cos(q3).*sin(alphaAC)))./lC+(LC.*dq3.*cos(q3).*cos(alphaAC-pi./2.0).*(y+aC.*cos(alphaAC)-eC.*cos(alphaAC)+LC.*cos(alphaAC).*cos(q3)))./lC))./(lC.*2.0)).*2.0)./lC+((((dz+LC.*dq3.*sin(pi./2.0).*cos(q3)).*(y+aC.*cos(alphaAC)-eC.*cos(alphaAC)+LC.*cos(alphaAC).*cos(q3)))./lC-((z+LC.*sin(q3)).*(dy+LC.*dq3.*sin(alphaAC-pi./2.0).*sin(q3)))./lC).*((IlCxx.*((LC.*sin(alphaAC-pi./2.0).*sin(q3).*(dz+LC.*dq3.*cos(q3)))./lC-(LC.*sin(pi./2.0).*cos(q3).*(dy-LC.*dq3.*cos(alphaAC).*sin(q3)))./lC+(LC.*dq3.*sin(alphaAC-pi./2.0).*cos(q3).*(z+LC.*sin(q3)))./lC+(LC.*dq3.*sin(pi./2.0).*sin(q3).*(y+aC.*cos(alphaAC)-eC.*cos(alphaAC)+LC.*cos(alphaAC).*cos(q3)))./lC))./(lC.*2.0)+(IlCxy.*((LC.*sin(pi./2.0).*cos(q3).*(dx-LC.*dq3.*sin(alphaAC).*sin(q3)))./lC+(LC.*sin(q3).*cos(alphaAC-pi./2.0).*(dz+LC.*dq3.*cos(q3)))./lC+(LC.*dq3.*cos(q3).*cos(alphaAC-pi./2.0).*(z+LC.*sin(q3)))./lC-(LC.*dq3.*sin(pi./2.0).*sin(q3).*(x+aC.*sin(alphaAC)-eC.*sin(alphaAC)+LC.*cos(q3).*sin(alphaAC)))./lC))./(lC.*2.0)-(IlCxz.*((LC.*sin(q3).*cos(alphaAC-pi./2.0).*(dy-LC.*dq3.*cos(alphaAC).*sin(q3)))./lC+(LC.*sin(alphaAC-pi./2.0).*sin(q3).*(dx-LC.*dq3.*sin(alphaAC).*sin(q3)))./lC+(LC.*dq3.*sin(alphaAC-pi./2.0).*cos(q3).*(x+aC.*sin(alphaAC)-eC.*sin(alphaAC)+LC.*cos(q3).*sin(alphaAC)))./lC+(LC.*dq3.*cos(q3).*cos(alphaAC-pi./2.0).*(y+aC.*cos(alphaAC)-eC.*cos(alphaAC)+LC.*cos(alphaAC).*cos(q3)))./lC))./(lC.*2.0)).*2.0)./lC+(((IlCzz.*(((dx-LC.*dq3.*sin(q3).*cos(alphaAC-pi./2.0)).*(y+aC.*cos(alphaAC)-eC.*cos(alphaAC)+LC.*cos(alphaAC).*cos(q3)))./lC-((dy+LC.*dq3.*sin(alphaAC-pi./2.0).*sin(q3)).*(x+aC.*sin(alphaAC)-eC.*sin(alphaAC)+LC.*cos(q3).*sin(alphaAC)))./lC).*(-1.0./2.0))./lC+(IlCxz.*(((dz+LC.*dq3.*sin(pi./2.0).*cos(q3)).*(y+aC.*cos(alphaAC)-eC.*cos(alphaAC)+LC.*cos(alphaAC).*cos(q3)))./lC-((z+LC.*sin(q3)).*(dy+LC.*dq3.*sin(alphaAC-pi./2.0).*sin(q3)))./lC))./(lC.*2.0)+(IlCyz.*(((z+LC.*sin(q3)).*(dx-LC.*dq3.*sin(q3).*cos(alphaAC-pi./2.0)))./lC-((dz+LC.*dq3.*sin(pi./2.0).*cos(q3)).*(x+aC.*sin(alphaAC)-eC.*sin(alphaAC)+LC.*cos(q3).*sin(alphaAC)))./lC))./(lC.*2.0)).*((LC.*cos(alphaAC).*sin(q3).*(dx-LC.*dq3.*sin(q3).*cos(alphaAC-pi./2.0)))./lC-(LC.*sin(alphaAC).*sin(q3).*(dy+LC.*dq3.*sin(alphaAC-pi./2.0).*sin(q3)))./lC+(LC.*dq3.*sin(alphaAC-pi./2.0).*cos(q3).*(x+aC.*sin(alphaAC)-eC.*sin(alphaAC)+LC.*cos(q3).*sin(alphaAC)))./lC+(LC.*dq3.*cos(q3).*cos(alphaAC-pi./2.0).*(y+aC.*cos(alphaAC)-eC.*cos(alphaAC)+LC.*cos(alphaAC).*cos(q3)))./lC).*2.0)./lC-(((IlCzz.*(((dx-LC.*dq3.*sin(q3).*cos(alphaAC-pi./2.0)).*(y+aC.*cos(alphaAC)-eC.*cos(alphaAC)+LC.*cos(alphaAC).*cos(q3)))./lC-((dy+LC.*dq3.*sin(alphaAC-pi./2.0).*sin(q3)).*(x+aC.*sin(alphaAC)-eC.*sin(alphaAC)+LC.*cos(q3).*sin(alphaAC)))./lC).*(-1.0./2.0))./lC+(IlCxz.*(((dz+LC.*dq3.*sin(pi./2.0).*cos(q3)).*(y+aC.*cos(alphaAC)-eC.*cos(alphaAC)+LC.*cos(alphaAC).*cos(q3)))./lC-((z+LC.*sin(q3)).*(dy+LC.*dq3.*sin(alphaAC-pi./2.0).*sin(q3)))./lC))./(lC.*2.0)+(IlCyz.*(((z+LC.*sin(q3)).*(dx-LC.*dq3.*sin(q3).*cos(alphaAC-pi./2.0)))./lC-((dz+LC.*dq3.*sin(pi./2.0).*cos(q3)).*(x+aC.*sin(alphaAC)-eC.*sin(alphaAC)+LC.*cos(q3).*sin(alphaAC)))./lC))./(lC.*2.0)).*((LC.*sin(q3).*cos(alphaAC-pi./2.0).*(dy-LC.*dq3.*cos(alphaAC).*sin(q3)))./lC+(LC.*sin(alphaAC-pi./2.0).*sin(q3).*(dx-LC.*dq3.*sin(alphaAC).*sin(q3)))./lC+(LC.*dq3.*sin(alphaAC-pi./2.0).*cos(q3).*(x+aC.*sin(alphaAC)-eC.*sin(alphaAC)+LC.*cos(q3).*sin(alphaAC)))./lC+(LC.*dq3.*cos(q3).*cos(alphaAC-pi./2.0).*(y+aC.*cos(alphaAC)-eC.*cos(alphaAC)+LC.*cos(alphaAC).*cos(q3)))./lC).*2.0)./lC+((((z+LC.*sin(q3)).*(dx-LC.*dq3.*sin(q3).*cos(alphaAC-pi./2.0)))./lC-((dz+LC.*dq3.*sin(pi./2.0).*cos(q3)).*(x+aC.*sin(alphaAC)-eC.*sin(alphaAC)+LC.*cos(q3).*sin(alphaAC)))./lC).*((IlCxy.*((LC.*cos(q3).*(dy+LC.*dq3.*sin(alphaAC-pi./2.0).*sin(q3)))./lC+(LC.*cos(alphaAC).*sin(q3).*(dz+LC.*dq3.*sin(pi./2.0).*cos(q3)))./lC+(LC.*dq3.*sin(alphaAC-pi./2.0).*cos(q3).*(z+LC.*sin(q3)))./lC+(LC.*dq3.*sin(pi./2.0).*sin(q3).*(y+aC.*cos(alphaAC)-eC.*cos(alphaAC)+LC.*cos(alphaAC).*cos(q3)))./lC).*(-1.0./2.0))./lC+(IlCyy.*((LC.*cos(q3).*(dx-LC.*dq3.*sin(q3).*cos(alphaAC-pi./2.0)))./lC+(LC.*sin(alphaAC).*sin(q3).*(dz+LC.*dq3.*sin(pi./2.0).*cos(q3)))./lC-(LC.*dq3.*cos(q3).*cos(alphaAC-pi./2.0).*(z+LC.*sin(q3)))./lC+(LC.*dq3.*sin(pi./2.0).*sin(q3).*(x+aC.*sin(alphaAC)-eC.*sin(alphaAC)+LC.*cos(q3).*sin(alphaAC)))./lC))./(lC.*2.0)+(IlCyz.*((LC.*cos(alphaAC).*sin(q3).*(dx-LC.*dq3.*sin(q3).*cos(alphaAC-pi./2.0)))./lC-(LC.*sin(alphaAC).*sin(q3).*(dy+LC.*dq3.*sin(alphaAC-pi./2.0).*sin(q3)))./lC+(LC.*dq3.*sin(alphaAC-pi./2.0).*cos(q3).*(x+aC.*sin(alphaAC)-eC.*sin(alphaAC)+LC.*cos(q3).*sin(alphaAC)))./lC+(LC.*dq3.*cos(q3).*cos(alphaAC-pi./2.0).*(y+aC.*cos(alphaAC)-eC.*cos(alphaAC)+LC.*cos(alphaAC).*cos(q3)))./lC))./(lC.*2.0)).*2.0)./lC+((((z+LC.*sin(q3)).*(dx-LC.*dq3.*sin(q3).*cos(alphaAC-pi./2.0)))./lC-((dz+LC.*dq3.*sin(pi./2.0).*cos(q3)).*(x+aC.*sin(alphaAC)-eC.*sin(alphaAC)+LC.*cos(q3).*sin(alphaAC)))./lC).*((IlCxy.*((LC.*sin(alphaAC-pi./2.0).*sin(q3).*(dz+LC.*dq3.*cos(q3)))./lC-(LC.*sin(pi./2.0).*cos(q3).*(dy-LC.*dq3.*cos(alphaAC).*sin(q3)))./lC+(LC.*dq3.*sin(alphaAC-pi./2.0).*cos(q3).*(z+LC.*sin(q3)))./lC+(LC.*dq3.*sin(pi./2.0).*sin(q3).*(y+aC.*cos(alphaAC)-eC.*cos(alphaAC)+LC.*cos(alphaAC).*cos(q3)))./lC))./(lC.*2.0)+(IlCyy.*((LC.*sin(pi./2.0).*cos(q3).*(dx-LC.*dq3.*sin(alphaAC).*sin(q3)))./lC+(LC.*sin(q3).*cos(alphaAC-pi./2.0).*(dz+LC.*dq3.*cos(q3)))./lC+(LC.*dq3.*cos(q3).*cos(alphaAC-pi./2.0).*(z+LC.*sin(q3)))./lC-(LC.*dq3.*sin(pi./2.0).*sin(q3).*(x+aC.*sin(alphaAC)-eC.*sin(alphaAC)+LC.*cos(q3).*sin(alphaAC)))./lC))./(lC.*2.0)-(IlCyz.*((LC.*sin(q3).*cos(alphaAC-pi./2.0).*(dy-LC.*dq3.*cos(alphaAC).*sin(q3)))./lC+(LC.*sin(alphaAC-pi./2.0).*sin(q3).*(dx-LC.*dq3.*sin(alphaAC).*sin(q3)))./lC+(LC.*dq3.*sin(alphaAC-pi./2.0).*cos(q3).*(x+aC.*sin(alphaAC)-eC.*sin(alphaAC)+LC.*cos(q3).*sin(alphaAC)))./lC+(LC.*dq3.*cos(q3).*cos(alphaAC-pi./2.0).*(y+aC.*cos(alphaAC)-eC.*cos(alphaAC)+LC.*cos(alphaAC).*cos(q3)))./lC))./(lC.*2.0)).*2.0)./lC+(((LC.*sin(pi./2.0).*cos(q3).*(y+aC.*cos(alphaAC)-eC.*cos(alphaAC)+LC.*cos(alphaAC).*cos(q3)))./lC-(LC.*sin(alphaAC-pi./2.0).*sin(q3).*(z+LC.*sin(q3)))./lC).*((IlCxx.*(((dz+LC.*dq3.*cos(q3)).*(dy+LC.*dq3.*sin(alphaAC-pi./2.0).*sin(q3)))./lC-((dy-LC.*dq3.*cos(alphaAC).*sin(q3)).*(dz+LC.*dq3.*sin(pi./2.0).*cos(q3)))./lC+((ddy+LC.*dq3.^2.*sin(alphaAC-pi./2.0).*cos(q3)).*(z+LC.*sin(q3)))./lC-((ddz-LC.*dq3.^2.*sin(pi./2.0).*sin(q3)).*(y+aC.*cos(alphaAC)-eC.*cos(alphaAC)+LC.*cos(alphaAC).*cos(q3)))./lC))./(lC.*2.0)-(IlCxy.*(((dz+LC.*dq3.*cos(q3)).*(dx-LC.*dq3.*sin(q3).*cos(alphaAC-pi./2.0)))./lC+((z+LC.*sin(q3)).*(ddx-LC.*dq3.^2.*cos(q3).*cos(alphaAC-pi./2.0)))./lC-((dx-LC.*dq3.*sin(alphaAC).*sin(q3)).*(dz+LC.*dq3.*sin(pi./2.0).*cos(q3)))./lC-((ddz-LC.*dq3.^2.*sin(pi./2.0).*sin(q3)).*(x+aC.*sin(alphaAC)-eC.*sin(alphaAC)+LC.*cos(q3).*sin(alphaAC)))./lC))./(lC.*2.0)+(IlCxz.*(((ddx-LC.*dq3.^2.*cos(q3).*cos(alphaAC-pi./2.0)).*(y+aC.*cos(alphaAC)-eC.*cos(alphaAC)+LC.*cos(alphaAC).*cos(q3)))./lC+((dy-LC.*dq3.*cos(alphaAC).*sin(q3)).*(dx-LC.*dq3.*sin(q3).*cos(alphaAC-pi./2.0)))./lC-((dx-LC.*dq3.*sin(alphaAC).*sin(q3)).*(dy+LC.*dq3.*sin(alphaAC-pi./2.0).*sin(q3)))./lC-((ddy+LC.*dq3.^2.*sin(alphaAC-pi./2.0).*cos(q3)).*(x+aC.*sin(alphaAC)-eC.*sin(alphaAC)+LC.*cos(q3).*sin(alphaAC)))./lC))./(lC.*2.0)).*2.0)./lC-(((LC.*sin(q3).*cos(alphaAC-pi./2.0).*(z+LC.*sin(q3)))./lC+(LC.*sin(pi./2.0).*cos(q3).*(x+aC.*sin(alphaAC)-eC.*sin(alphaAC)+LC.*cos(q3).*sin(alphaAC)))./lC).*((IlCxy.*(((dz+LC.*dq3.*cos(q3)).*(dy+LC.*dq3.*sin(alphaAC-pi./2.0).*sin(q3)))./lC-((dy-LC.*dq3.*cos(alphaAC).*sin(q3)).*(dz+LC.*dq3.*sin(pi./2.0).*cos(q3)))./lC+((ddy+LC.*dq3.^2.*sin(alphaAC-pi./2.0).*cos(q3)).*(z+LC.*sin(q3)))./lC-((ddz-LC.*dq3.^2.*sin(pi./2.0).*sin(q3)).*(y+aC.*cos(alphaAC)-eC.*cos(alphaAC)+LC.*cos(alphaAC).*cos(q3)))./lC))./(lC.*2.0)-(IlCyy.*(((dz+LC.*dq3.*cos(q3)).*(dx-LC.*dq3.*sin(q3).*cos(alphaAC-pi./2.0)))./lC+((z+LC.*sin(q3)).*(ddx-LC.*dq3.^2.*cos(q3).*cos(alphaAC-pi./2.0)))./lC-((dx-LC.*dq3.*sin(alphaAC).*sin(q3)).*(dz+LC.*dq3.*sin(pi./2.0).*cos(q3)))./lC-((ddz-LC.*dq3.^2.*sin(pi./2.0).*sin(q3)).*(x+aC.*sin(alphaAC)-eC.*sin(alphaAC)+LC.*cos(q3).*sin(alphaAC)))./lC))./(lC.*2.0)+(IlCyz.*(((ddx-LC.*dq3.^2.*cos(q3).*cos(alphaAC-pi./2.0)).*(y+aC.*cos(alphaAC)-eC.*cos(alphaAC)+LC.*cos(alphaAC).*cos(q3)))./lC+((dy-LC.*dq3.*cos(alphaAC).*sin(q3)).*(dx-LC.*dq3.*sin(q3).*cos(alphaAC-pi./2.0)))./lC-((dx-LC.*dq3.*sin(alphaAC).*sin(q3)).*(dy+LC.*dq3.*sin(alphaAC-pi./2.0).*sin(q3)))./lC-((ddy+LC.*dq3.^2.*sin(alphaAC-pi./2.0).*cos(q3)).*(x+aC.*sin(alphaAC)-eC.*sin(alphaAC)+LC.*cos(q3).*sin(alphaAC)))./lC))./(lC.*2.0)).*2.0)./lC-(LC.*g.*mLC.*cos(q3))./2.0-LC.*g.*mlC.*cos(q3)-(LC.*mlC.*sin(q3).*cos(alphaAC-pi./2.0).*(ddx./2.0+(LC.*dq3.^2.*cos(q3).*cos(alphaAC-pi./2.0))./2.0))./2.0-LC.*mlC.*sin(q3).*cos(alphaAC-pi./2.0).*(ddx./4.0+(LC.*dq3.^2.*cos(q3).*cos(alphaAC-pi./2.0))./4.0)+(LC.*mlC.*sin(alphaAC-pi./2.0).*sin(q3).*(ddy./2.0-(LC.*dq3.^2.*sin(alphaAC-pi./2.0).*cos(q3))./2.0))./2.0+LC.*mlC.*sin(alphaAC-pi./2.0).*sin(q3).*(ddy./4.0-(LC.*dq3.^2.*sin(alphaAC-pi./2.0).*cos(q3))./4.0)+(LC.*mlC.*sin(pi./2.0).*cos(q3).*(ddz./2.0+(LC.*dq3.^2.*sin(pi./2.0).*sin(q3))./2.0))./2.0+LC.*mlC.*sin(pi./2.0).*cos(q3).*(ddz./4.0+(LC.*dq3.^2.*sin(pi./2.0).*sin(q3))./4.0)];

Mtimesddq = M*ddq;

tau = Mtimesddq - f;
